simulink model "Control_model_10DOF_fin"  (R2016b)
settings: Solver=FixedStepAuto  StartTime=0.0  StopTime=10  FixedStep=0.0001  RelTol=1e-3
InitFcn:
  | Initialisation_ctr_10DOF_fin
values from neighbouring files (symbols this model uses):
  COM_Parameters = [-lpelvis/2;r2;0]    [Initialisation_ctr_10DOF_fin.m]
  DH_Parameters = [hfoot 0 ... (first row only)    [Initialisation_ctr_10DOF_fin.m]
  dTrunk = trunklbd(3)    [Initialisation_ctr_10DOF_fin.m]
  dxFootSM = dxFoot    [Initialisation_ctr_10DOF_fin.m]
  dxTrunk = 0.1    [Initialisation_ctr_10DOF_fin.m]
  Foot_Parameters = [0;-(lFoot/2-lHeel);0]    [Initialisation_ctr_10DOF_fin.m]
  HAA2HEE = [0; 0; 0.001]    [Initialisation_ctr_10DOF_fin.m]
  HEE2HFE = 0.5*[0.2; 0; 0]    [Initialisation_ctr_10DOF_fin.m]
  height_vrp = CoM_position(1)    [Initialisation_ctr_10DOF_fin.m]
  hTrunk = trunklbd(1)    [Initialisation_ctr_10DOF_fin.m]
  initial_CoM_position = R*CoM_position    [Initialisation_ctr_10DOF_fin.m]
  initial_CoM_velocity = [0;0;0]    [Initialisation_ctr_10DOF_fin.m]
  initial_left_foot = [0;0;-stance_width/2]    [Initialisation_ctr_10DOF_fin.m]
  initial_right_foot = [0;0;stance_width/2]    [Initialisation_ctr_10DOF_fin.m]
  initial_RorL = 0    [Initialisation_ctr_10DOF_fin.m]
  jointsinitial = [9;-15;6;0;0;6;-15;9]/180*pi    [Initialisation_ctr_10DOF_fin.m]
  K_DCM = 4.3*[1 0 0 ... (first row only)    [Initialisation_ctr_10DOF_fin.m]
  kD_left = mbody*[0.95 0 0 0 ... (first row only)    [Initialisation_ctr_10DOF_fin.m]
  kD_right = mbody*[0.12 0 0 0 ... (first row only)    [Initialisation_ctr_10DOF_fin.m]
  kI_left = mbody*[35 0 0 0 ... (first row only)    [Initialisation_ctr_10DOF_fin.m]
  kI_right = mbody*[38.2 0 0 0 ... (first row only)    [Initialisation_ctr_10DOF_fin.m]
  kP_left = mbody*[75 0 0 0 ... (first row only)    [Initialisation_ctr_10DOF_fin.m]
  kP_right = mbody*[5.6 0 0 0 ... (first row only)    [Initialisation_ctr_10DOF_fin.m]
  Lenght = [lShank;lThigh]    [Initialisation_ctr_10DOF_fin.m]
  lFootSM = lFoot    [Initialisation_ctr_10DOF_fin.m]
  lpelvis = wPelvis    [Initialisation_ctr_10DOF_fin.m]
  mass = mbody    (= 60)    [Initialisation_ctr_10DOF_fin.m]
  Masses = [mThigh; mShank; mTrunk]    [Initialisation_ctr_10DOF_fin.m]
  nb_step = 4    [Initialisation_ctr_10DOF_fin.m]
  nb_step_pattern = 20    [Initialisation_ctr_10DOF_fin.m]
  Pelvis_Parameters = [-lpelvis/2;hTrunk/2;0]    [Initialisation_ctr_10DOF_fin.m]
  stance_width = lpelvis    [Initialisation_ctr_10DOF_fin.m]
  stride_lenght = 0.50    (= 0.5)    [Initialisation_ctr_10DOF_fin.m]
  T_DS = time_DS    (= 0.4)    [Initialisation_ctr_10DOF_fin.m]
  T_IT = time_DS    (= 0.4)    [Initialisation_ctr_10DOF_fin.m]
  T_SS = time_swing    (= 1.6)    [Initialisation_ctr_10DOF_fin.m]
  time_DS = (time_stance-time_swing)/2    (= 0.4)    [Initialisation_ctr_10DOF_fin.m]
  time_stance = 60/100*time_stride    (= 2.4)    [Initialisation_ctr_10DOF_fin.m]
  time_step = time_stride/2    (= 2)    [Initialisation_ctr_10DOF_fin.m]
  time_swing = 40/100*time_stride    (= 1.6)    [Initialisation_ctr_10DOF_fin.m]
  validity_angle = [-20*pi/180 20*pi/180 ... (first row only)    [Initialisation_ctr_10DOF_fin.m]
  wTrunk = trunklbd(2)    [Initialisation_ctr_10DOF_fin.m]
  x4CoM = CoM_position(1)-XR4(1)    [Initialisation_ctr_10DOF_fin.m]
undefined symbols (not defined in the file or in its folder): dsegment, hFoot, l, lFoot, omega0_x, omega0_z, rho, wPelvis, X, Xp_x, Xp_z, Y, Z
undefined symbols (not defined in the file): k_grf, lShankSM, lThighSM, mShank, mThigh
libraries: nesl_utility x247, sm_lib x215, dspindex x12, FootPlacementLibrary x8, dspsigops x4, dspswit3 x1
(part 16 of 18)

== matlab function Control_model_10DOF_fin/Forward Kinematics/Forward Kinematics ==
  data: TR0 output; TR1 output; TR2 output; TR3 output; TR4 output; TR5 output; TR6 output; TR7 output; TR8 output; TR9 output; TRL output; TRthighR output; TRshankR output; TRtrunk output; TRshankL output; TRthighL output; TL9 output; TL8 output; TL7 output; TL6 output; TL5 output; TL4 output; TL3 output; TL2 output; TL1 output; TL0 output; TLR output; TLthighL output; TLshankL output; TLtrunk output; TLshankR output; TLthighR output; TWR output; TWL output; TW0 output; TW1 output; TW2 output; TW3 output; TW4 output; TW5 output; TW6 output; TW7 output; TW8 output; TW9 output; TWthighR output; TWthighL output; TWshankR output; TWshankL output; TWtrunk output; XRcom output; XLcom output; XWcom output; joint_angle input double; DH_Parameters parameter double size=[9 2]; COM_Parameters parameter double size=[3 1]; Foot_Parameters parameter double size=[3 1]; inactuated_joint_angle input; V_CoM input; R_foot_Rotation input; Masses parameter; Lenght parameter; Pelvis_Parameters parameter; R_foot_pos input; VWcom output; AWcom output; L_foot_Rotation input; L_foot_pos input; JRcom output; JLcom output; A_CoM input
function [TR0,TR1,TR2,TR3,TR4,TR5,TR6,TR7,TR8,TR9,TRL,TRthighR,TRshankR,TRtrunk,TRshankL,TRthighL,TL9,TL8,TL7,TL6,TL5,TL4,TL3,TL2,TL1,TL0,TLR,TLthighL,TLshankL,TLtrunk,TLshankR,TLthighR,TWR,TWL,TW0,TW1,TW2,TW3,TW4,TW5,TW6,TW7,TW8,TW9,TWthighR,TWthighL,TWshankR,TWshankL,TWtrunk,XRcom,XLcom,XWcom,VWcom,AWcom,JRcom,JLcom]=Forward_Kinematics(joint_angle,DH_Parameters, COM_Parameters, Foot_Parameters,inactuated_joint_angle,V_CoM,R_foot_Rotation,Masses, Lenght,Pelvis_Parameters,R_foot_pos,L_foot_Rotation,L_foot_pos,A_CoM)

%% angle
theta1=joint_angle(1);
theta2=joint_angle(2);
theta3=joint_angle(3);
theta4=joint_angle(4);
theta5=joint_angle(5);
theta6=joint_angle(6);
theta7=joint_angle(7);
theta8=joint_angle(8);
theta0=inactuated_joint_angle(1);
theta9=inactuated_joint_angle(2);

%% Denavit-Hartenberg parmeters
a0=DH_Parameters(1,1);
d1=DH_Parameters(1,2);
a1=DH_Parameters(2,1);
d2=DH_Parameters(2,2);
a2=DH_Parameters(3,1);
d3=DH_Parameters(3,2);
a3=DH_Parameters(4,1);
d4=DH_Parameters(4,2);
a4=DH_Parameters(5,1);
d5=DH_Parameters(5,2);
a5=DH_Parameters(6,1);
d6=DH_Parameters(6,2);
a6=DH_Parameters(7,1);
d7=DH_Parameters(7,2);
a7=DH_Parameters(8,1);
d8=DH_Parameters(8,2);
a8=DH_Parameters(9,1);
d9=DH_Parameters(9,2);

xcom=COM_Parameters(1);
ycom=COM_Parameters(2);
zcom=COM_Parameters(3);
xfoot=Foot_Parameters(1);
yfoot=Foot_Parameters(2);
zfoot=Foot_Parameters(3);

%% Pelvis Parameters
xpelvis=Pelvis_Parameters(1);
ypelvis=Pelvis_Parameters(2);
zpelvis=Pelvis_Parameters(3);


%% Masses
mthigh=Masses(1);
mshank=Masses(2);
mtrunk=Masses(3);

%% Lenght
lshank=Lenght(1);
lthigh=Lenght(2);


%Matrice de Transformation Homogéne

% World -> Right foot marker R

TWR_D=[R_foot_Rotation(1,1) R_foot_Rotation(1,2) R_foot_Rotation(1,3) R_foot_pos(1);
    R_foot_Rotation(2,1) R_foot_Rotation(2,2) R_foot_Rotation(2,3) R_foot_pos(2);
    R_foot_Rotation(3,1) R_foot_Rotation(3,2) R_foot_Rotation(3,3) R_foot_pos(3);
    0 0 0 1];

T=[0 1 0 0;
    1 0 0 0;
    0 0 -1 0;
    0 0 0 1];

TWR=TWR_D*T;

RWR=TWR(1:3,1:3);
XWR=TWR(1:3,4);

% World -> Left foot marker L

TWL_D=[L_foot_Rotation(1,1) L_foot_Rotation(1,2) L_foot_Rotation(1,3) L_foot_pos(1);
    L_foot_Rotation(2,1) L_foot_Rotation(2,2) L_foot_Rotation(2,3) L_foot_pos(2);
    L_foot_Rotation(3,1) L_foot_Rotation(3,2) L_foot_Rotation(3,3) L_foot_pos(3);
    0 0 0 1];

T=[0 -1 0 0;
    1 0 0 0;
    0 0 1 0;
    0 0 0 1];

TWL=TWL_D*T;

RWL=TWL(1:3,1:3);
XWL=TWL(1:3,4);


%Right foot marker R -> Right foot marker 0

TR0=[1 0 0 xfoot;
    0 1 0 yfoot;
    0 0 1 zfoot;
    0 0 0 1];

T0R=[1 0 0 -xfoot;
    0 1 0 -yfoot;
    0 0 1 -zfoot;
    0 0 0 1];

% Right foot marker 0 -> Right ankle eversion/inversion

T0ankleR=[cos(theta0) 0 sin(theta0) a0;
    0 1 0 0;
    -sin(theta0) 0 cos(theta0) 0;
    0 0 0 1];

R0ankleR=[cos(theta0) 0 sin(theta0);
    0 1 0;
    -sin(theta0) 0 cos(theta0)];

O0OankleR=[a0;0;0];

TankleR0=[R0ankleR.' -R0ankleR.'*O0OankleR;
    0 0 0 1];

% Right ankle eversion/inversion -> Right ankle flexion/extension

TankleR1=[cos(theta1) -sin(theta1) 0 0;
    sin(theta1) cos(theta1) 0 0;
    0 0 1 0;
    0 0 0 1];

RankleR1=[cos(theta1) -sin(theta1) 0;
    sin(theta1) cos(theta1) 0;
    0 0 1];

OankleRO1=[0;0;0];

T1ankleR=[RankleR1.' OankleRO1;
    0 0 0 1];

% Right ankle -> Right knee

T12=[cos(theta2) -sin(theta2) 0 a1;
    sin(theta2) cos(theta2) 0 0;
    0 0 1 0;
    0 0 0 1];

R12=[cos(theta2) -sin(theta2) 0;
    sin(theta2) cos(theta2) 0;
    0 0 1];

O1O2=[a1;0;0];

T21=[R12.' -R12.'*O1O2;
    0 0 0 1];

% Right knee -> Right hip flexion/extension

T23=[cos(theta3) -sin(theta3) 0 a2;
    sin(theta3) cos(theta3) 0 0;
    0 0 1 d3;
    0 0 0 1];

R23=[cos(theta3) -sin(theta3) 0;
    sin(theta3) cos(theta3) 0;
    0 0 1];

O2O3=[a2;0;d3];

T32=[R23.' -R23.'*O2O3;
    0 0 0 1];

% Right hip flexion/extension -> Right hip abduction

T34=[cos(theta4-pi/2) -sin(theta4-pi/2) 0 0;
    0 0 -1 0;
    sin(theta4-pi/2) cos(theta4-pi/2) 0 0;
    0 0 0 1];

R34=[cos(theta4-pi/2) -sin(theta4-pi/2) 0;
    0 0 -1;
    sin(theta4-pi/2) cos(theta4-pi/2) 0];

O3O4=[0;0;0];

T43=[R34.' -R34.'*O3O4;
    0 0 0 1];

%Right hip abduction -> Left hip aduction

T45=[cos(theta5-pi/2) -sin(theta5-pi/2) 0 a4;
    -sin(theta5-pi/2) -cos(theta5-pi/2) 0 0;
    0 0 -1 0;
    0 0 0 1];

R45=[cos(theta5-pi/2) -sin(theta5-pi/2) 0;
    -sin(theta5-pi/2) -cos(theta5-pi/2) 0;
    0 0 -1];

O4O5=[a4;0;0];

T54=[R45 -R45*O4O5;
    0 0 0 1];

% Left hip abduction -> Left hip flexion

T56=[cos(theta6) -sin(theta6) 0 0;
    0 0 1 0;
    -sin(theta6) -cos(theta6) 0 0;
    0 0 0 1];

R56=[cos(theta6) -sin(theta6) 0;
    0 0 1;
    -sin(theta6) -cos(theta6) 0];

O5O6=[0;0;0];

T65=[R56.' -R56.'*O5O6;
    0 0 0 1];

% Left hip flexion -> Left knee

T67=[cos(theta7) -sin(theta7) 0 a6;
    sin(theta7) cos(theta7) 0 0;
    0 0 1 d7;
    0 0 0 1];

R67=[cos(theta7) -sin(theta7) 0;
    sin(theta7) cos(theta7) 0;
    0 0 1];

O6O7=[a6;0;d7];

T76=[R67.' -R67.'*O6O7;
    0 0 0 1];

% Left knee -> Left ankle flexion/extension

T78=[cos(theta8) -sin(theta8) 0 a7;
    sin(theta8) cos(theta8) 0 0;
    0 0 1 0;
    0 0 0 1];

R78=[cos(theta8) -sin(theta8) 0;
    sin(theta8) cos(theta8) 0;
    0 0 1];

O7O8=[a7;0;0];

T87=[R78.' -R78.'*O7O8;
    0 0 0 1];

% Left ankle flexion/extension -> Left ankle eversion/inversion

T8ankleL=[cos(theta9) 0 -sin(theta9) 0;
    0 1 0 0;
    sin(theta9) 0 cos(theta9) 0;
    0 0 0 1];

R8ankleL=[cos(theta9) 0 -sin(theta9);
    0 1 0;
    sin(theta9) 0 cos(theta9)];

O8OankleL=[0;0;0];

TankleL8=[R8ankleL.' -R8ankleL.'*O8OankleL;
    0 0 0 1];


% Left ankle eversion/inversion -> Left foot marker 9

TankleL9=[1 0 0 a8;
    0 1 0 0;
    0 0 1 0;
    0 0 0 1];

T9ankleL=[1 0 0 -a8;
    0 1 0 0;
    0 0 1 0;
    0 0 0 1];

% Left foot marker L

T9L=[1 0 0 -xfoot;
    0 1 0 yfoot;
    0 0 1 zfoot;
    0 0 0 1];

TL9=[1 0 0 xfoot;
    0 1 0 -yfoot;
    0 0 1 -zfoot;
    0 0 0 1];

% Right ankle -> Right shank

T1shank=[1 0 0 lshank/2;
    0 1 0 0;
    0 0 1 0;
    0 0 0 1];

Tshank1=[1 0 0 -lshank/2;
    0 1 0 0;
    0 0 1 0;
    0 0 0 1];

% Left knee -> Left Shank

T7shank=[1 0 0 -lshank/2;
    0 1 0 0;
    0 0 1 0;
    0 0 0 1];

Tshank7=[1 0 0 lshank/2;
    0 1 0 0;
    0 0 1 0;
    0 0 0 1];

% Right knee -> Right thigh

T2thigh=[1 0 0 lthigh/2;
    0 1 0 0;
    0 0 1 0;
    0 0 0 1];

Tthigh2=[1 0 0 -lthigh/2;
    0 1 0 0;
    0 0 1 0;
    0 0 0 1];

% Left hip -> Left thigh

T6thigh=[1 0 0 -lthigh/2;
    0 1 0 0 ;
    0 0 1 d7;
    0 0 0 1];

Tthigh6=[1 0 0 lthigh/2;
    0 1 0 0 ;
    0 0 1 -d7;
    0 0 0 1];

% Right hip -> Trunk

T4trunk=[1 0 0 xpelvis;
    0 1 0 ypelvis;
    0 0 1 zpelvis;
    0 0 0 1];

Ttrunk4=[1 0 0 -xpelvis;
    0 1 0 -ypelvis;
    0 0 1 -zpelvis;
    0 0 0 1];

% Right foot frame marker 0

T01=T0ankleR*TankleR1;
T02=T01*T12;
T03=T02*T23;
T04=T03*T34;
T05=T04*T45;
T06=T05*T56;
T07=T06*T67;
T08=T07*T78;
T0ankleL=T08*T8ankleL;
T09=T0ankleL*TankleL9;
T0L=T09*T9L;

T0thighR=T02*T2thigh;
T0thighL=T06*T6thigh;
T0shankR=T01*T1shank;
T0shankL=T07*T7shank;
T0trunk=T04*T4trunk;

X0thighR=T0thighR(1:3,4);
X0thighL=T0thighL(1:3,4);
X0shankR=T0shankR(1:3,4);
X0shankL=T0shankL(1:3,4);
X0trunk=T0trunk(1:3,4);

X0com=(mthigh*X0thighR+mthigh*X0thighL+mshank*X0shankR+mshank*X0shankL+mtrunk*X0trunk)/(2*mthigh+2*mshank+mtrunk);


% Right foot frame marker R

TR1=TR0*T0ankleR*TankleR1;
TR2=TR1*T12;
TR3=TR2*T23;
TR4=TR3*T34;
TR5=TR4*T45;
TR6=TR5*T56;
TR7=TR6*T67;
TR8=TR7*T78;
TRankleL=TR8*T8ankleL;
TR9=TRankleL*TankleL9;
TRL=TR9*T9L;

TRthighR=TR2*T2thigh;
TRthighL=TR6*T6thigh;
TRshankR=TR1*T1shank;
TRshankL=TR7*T7shank;
TRtrunk=TR4*T4trunk;

XRthighR=TRthighR(1:3,4);
XRthighL=TRthighL(1:3,4);
XRshankR=TRshankR(1:3,4);
XRshankL=TRshankL(1:3,4);
XRtrunk=TRtrunk(1:3,4);

XRcom=(mthigh*XRthighR+mthigh*XRthighL+mshank*XRshankR+mshank*XRshankL+mtrunk*XRtrunk)/(2*mthigh+2*mshank+mtrunk);

% TRcom
% 
% xRcom=XRcom(1);
% yRcom=yRcom(2);

%Left foot frame marker 9

T98=T9ankleL*TankleL8;
T97=T98*T87;
T96=T97*T76;
T95=T96*T65;
T94=T95*T54;
T93=T94*T43;
T92=T93*T32;
T91=T92*T21;
T90=T91*T1ankleR*TankleR0;
T9R=T90*T0R;

T9thighL=T96*T6thigh;
T9thighR=T92*T2thigh;
T9shankL=T97*T7shank;
T9shankR=T91*T1shank;
T9trunk=T94*T4trunk;

X9thighL=T9thighL(1:3,4);
X9thighR=T9thighR(1:3,4);
X9shankL=T9shankL(1:3,4);
X9shankR=T9shankR(1:3,4);
X9trunk=T9trunk(1:3,4);

X9com=(mthigh*X9thighR+mthigh*X9thighL+mshank*X9shankR+mshank*X9shankL+mtrunk*X9trunk)/(2*mthigh+2*mshank+mtrunk);


%Left foot repere marker L

TL8=TL9*T9ankleL*TankleL8;
TL7=TL8*T87;
TL6=TL7*T76;
TL5=TL6*T65;
TL4=TL5*T54;
TL3=TL4*T43;
TL2=TL3*T32;
TL1=TL2*T21;
TL0=TL1*T1ankleR*TankleR0;
TLR=TL0*T0R;

TLthighL=TL6*T6thigh;
TLthighR=TL2*T2thigh;
TLshankL=TL7*T7shank;
TLshankR=TL1*T1shank;
TLtrunk=TL4*T4trunk;

XLthighL=TLthighL(1:3,4);
XLthighR=TLthighR(1:3,4);
XLshankL=TLshankL(1:3,4);
XLshankR=TLshankR(1:3,4);
XLtrunk=TLtrunk(1:3,4);

XLcom=(mthigh*XLthighR+mthigh*XLthighL+mshank*XLshankR+mshank*XLshankL+mtrunk*XLtrunk)/(2*mthigh+2*mshank+mtrunk);


% World frame

TW0=TWR*TR0;
TW1=TWR*TR1;
TW2=TWR*TR2;
TW3=TWR*TR3;
TW4=TWR*TR4;
TW5=TWL*TL5;
TW6=TWL*TL6;
TW7=TWL*TL7;
TW8=TWL*TL8;
TW9=TWL*TL9;


% TW0=TWL*TL0;
% TW1=TWL*TL1;
% TW2=TWL*TL2;
% TW3=TWL*TL3;
% TW4=TWL*TL4;
% TW5=TWL*TL5;
% TW6=TWL*TL6;
% TW7=TWL*TL7;
% TW8=TWL*TL8;
% TW9=TWL*TL9;



TWthighR=TW2*T2thigh;
TWthighL=TW6*T6thigh;
TWshankR=TW1*T1shank;
TWshankL=TW7*T7shank;
TWtrunk=TW4*T4trunk;

XWshankR=TWshankR(1:3,4);
XWshankL=TWshankL(1:3,4);
XWthighR=TWthighR(1:3,4);
XWthighL=TWthighL(1:3,4);
XWtrunk=TWtrunk(1:3,4);

XWcom=(mthigh*XWthighR+mthigh*XWthighL+mshank*XWshankR+mshank*XWshankL+mtrunk*XWtrunk)/(2*mthigh+2*mshank+mtrunk);



%%%%%%%%%%%%%%%%%%%%%%%%%%%%%%%%%%%%%%%%%%%%%%%%%%%%%%%%%%%%%%%%%%%%%%%%%%%%%%%%%%%%%%%%%%%%%%%%%%

JRcom=zeros(3,8);
JLcom=zeros(3,8);

    %CoM jacobian right foot repere

% JRcom(1,1)=zcom*cos(theta1 + theta2 + theta3)*cos(theta0) - a1*cos(theta0)*sin(theta1) - a2*sin(theta1 + theta2)*cos(theta0) - ycom*sin(theta1 + theta2 + theta3)*cos(theta0)*cos(theta4) - xcom*sin(theta1 + theta2 + theta3)*cos(theta0)*sin(theta4);
% JRcom(1,2)=zcom*cos(theta1 + theta2 + theta3)*cos(theta0) - a2*sin(theta1 + theta2)*cos(theta0) - ycom*sin(theta1 + theta2 + theta3)*cos(theta0)*cos(theta4) - xcom*sin(theta1 + theta2 + theta3)*cos(theta0)*sin(theta4);
% JRcom(1,3)=zcom*cos(theta1 + theta2 + theta3)*cos(theta0) - ycom*sin(theta1 + theta2 + theta3)*cos(theta0)*cos(theta4) - xcom*sin(theta1 + theta2 + theta3)*cos(theta0)*sin(theta4);
% JRcom(1,4)=ycom*cos(theta4)*sin(theta0) + xcom*sin(theta0)*sin(theta4) + xcom*cos(theta1 + theta2 + theta3)*cos(theta0)*cos(theta4) - ycom*cos(theta1 + theta2 + theta3)*cos(theta0)*sin(theta4);
% 
% JRcom(2,1)=zcom*sin(theta1 + theta2 + theta3) + a2*cos(theta1 + theta2) + (ycom*cos(theta1 + theta2 + theta3 + theta4))/2 + (xcom*sin(theta1 + theta2 + theta3 + theta4))/2 + a1*cos(theta1) + (ycom*cos(theta1 + theta2 + theta3 - theta4))/2 - (xcom*sin(theta1 + theta2 + theta3 - theta4))/2;
% JRcom(2,2)=zcom*sin(theta1 + theta2 + theta3) + a2*cos(theta1 + theta2) + (ycom*cos(theta1 + theta2 + theta3 + theta4))/2 + (xcom*sin(theta1 + theta2 + theta3 + theta4))/2 + (ycom*cos(theta1 + theta2 + theta3 - theta4))/2 - (xcom*sin(theta1 + theta2 + theta3 - theta4))/2;
% JRcom(2,3)=zcom*sin(theta1 + theta2 + theta3) + (ycom*cos(theta1 + theta2 + theta3 + theta4))/2 + (xcom*sin(theta1 + theta2 + theta3 + theta4))/2 + (ycom*cos(theta1 + theta2 + theta3 - theta4))/2 - (xcom*sin(theta1 + theta2 + theta3 - theta4))/2;
% JRcom(2,4)=(ycom*cos(theta1 + theta2 + theta3 + theta4))/2 + (xcom*sin(theta1 + theta2 + theta3 + theta4))/2 - (ycom*cos(theta1 + theta2 + theta3 - theta4))/2 + (xcom*sin(theta1 + theta2 + theta3 - theta4))/2;
% 
% JRcom(3,1)=a2*sin(theta1 + theta2)*sin(theta0) + a1*sin(theta0)*sin(theta1) - zcom*cos(theta1 + theta2 + theta3)*sin(theta0) + ycom*sin(theta1 + theta2 + theta3)*cos(theta4)*sin(theta0) + xcom*sin(theta1 + theta2 + theta3)*sin(theta0)*sin(theta4);
% JRcom(3,2)=a2*sin(theta1 + theta2)*sin(theta0) - zcom*cos(theta1 + theta2 + theta3)*sin(theta0) + ycom*sin(theta1 + theta2 + theta3)*cos(theta4)*sin(theta0) + xcom*sin(theta1 + theta2 + theta3)*sin(theta0)*sin(theta4);
% JRcom(3,3)=ycom*sin(theta1 + theta2 + theta3)*cos(theta4)*sin(theta0) - zcom*cos(theta1 + theta2 + theta3)*sin(theta0) + xcom*sin(theta1 + theta2 + theta3)*sin(theta0)*sin(theta4);
% JRcom(3,4)=xcom*(cos(theta0)*sin(theta4) - cos(theta1 + theta2 + theta3)*cos(theta4)*sin(theta0)) + ycom*(cos(theta0)*cos(theta4) + cos(theta1 + theta2 + theta3)*sin(theta0)*sin(theta4));

JRcom(1,1)=-(2*a1*mshank*cos(theta0)*sin(theta1) + 4*a1*mthigh*cos(theta0)*sin(theta1) + 2*a1*mtrunk*cos(theta0)*sin(theta1) + lshank*mshank*cos(theta0)*sin(theta1) + 2*a2*mshank*cos(theta0)*cos(theta1)*sin(theta2) + 2*a2*mshank*cos(theta0)*cos(theta2)*sin(theta1) + 2*a2*mthigh*cos(theta0)*cos(theta1)*sin(theta2) + 2*a2*mthigh*cos(theta0)*cos(theta2)*sin(theta1) + 2*a2*mtrunk*cos(theta0)*cos(theta1)*sin(theta2) + 2*a2*mtrunk*cos(theta0)*cos(theta2)*sin(theta1) + lthigh*mthigh*cos(theta0)*cos(theta1)*sin(theta2) + lthigh*mthigh*cos(theta0)*cos(theta2)*sin(theta1) - 2*mtrunk*zpelvis*cos(theta0)*cos(theta1)*cos(theta2)*cos(theta3) + 2*mtrunk*zpelvis*cos(theta0)*cos(theta1)*sin(theta2)*sin(theta3) + 2*mtrunk*zpelvis*cos(theta0)*cos(theta2)*sin(theta1)*sin(theta3) + 2*mtrunk*zpelvis*cos(theta0)*cos(theta3)*sin(theta1)*sin(theta2) - 2*a6*mshank*cos(theta0)*cos(theta1)*cos(theta2)*cos(theta3)*sin(theta6) + lthigh*mthigh*cos(theta0)*cos(theta1)*cos(theta2)*cos(theta3)*sin(theta6) + 2*a4*mshank*cos(theta0)*cos(theta1)*cos(theta2)*sin(theta3)*sin(theta4) + 2*a4*mshank*cos(theta0)*cos(theta1)*cos(theta3)*sin(theta2)*sin(theta4) + 2*a4*mshank*cos(theta0)*cos(theta2)*cos(theta3)*sin(theta1)*sin(theta4) + 2*a4*mthigh*cos(theta0)*cos(theta1)*cos(theta2)*sin(theta3)*sin(theta4) + 2*a4*mthigh*cos(theta0)*cos(theta1)*cos(theta3)*sin(theta2)*sin(theta4) + 2*a4*mthigh*cos(theta0)*cos(theta2)*cos(theta3)*sin(theta1)*sin(theta4) + 2*mtrunk*ypelvis*cos(theta0)*cos(theta1)*cos(theta2)*cos(theta4)*sin(theta3) + 2*mtrunk*ypelvis*cos(theta0)*cos(theta1)*cos(theta3)*cos(theta4)*sin(theta2) + 2*mtrunk*ypelvis*cos(theta0)*cos(theta2)*cos(theta3)*cos(theta4)*sin(theta1) + 2*a6*mshank*cos(theta0)*cos(theta1)*sin(theta2)*sin(theta3)*sin(theta6) + 2*a6*mshank*cos(theta0)*cos(theta2)*sin(theta1)*sin(theta3)*sin(theta6) + 2*a6*mshank*cos(theta0)*cos(theta3)*sin(theta1)*sin(theta2)*sin(theta6) + 2*mtrunk*xpelvis*cos(theta0)*cos(theta1)*cos(theta2)*sin(theta3)*sin(theta4) + 2*mtrunk*xpelvis*cos(theta0)*cos(theta1)*cos(theta3)*sin(theta2)*sin(theta4) + 2*mtrunk*xpelvis*cos(theta0)*cos(theta2)*cos(theta3)*sin(theta1)*sin(theta4) - lthigh*mthigh*cos(theta0)*cos(theta1)*sin(theta2)*sin(theta3)*sin(theta6) - lthigh*mthigh*cos(theta0)*cos(theta2)*sin(theta1)*sin(theta3)*sin(theta6) - lthigh*mthigh*cos(theta0)*cos(theta3)*sin(theta1)*sin(theta2)*sin(theta6) - 2*a4*mshank*cos(theta0)*sin(theta1)*sin(theta2)*sin(theta3)*sin(theta4) - 2*a4*mthigh*cos(theta0)*sin(theta1)*sin(theta2)*sin(theta3)*sin(theta4) - 2*mtrunk*ypelvis*cos(theta0)*cos(theta4)*sin(theta1)*sin(theta2)*sin(theta3) - 2*mtrunk*xpelvis*cos(theta0)*sin(theta1)*sin(theta2)*sin(theta3)*sin(theta4) + lshank*mshank*cos(theta0)*cos(theta1)*cos(theta2)*cos(theta3)*cos(theta6)*sin(theta7) + lshank*mshank*cos(theta0)*cos(theta1)*cos(theta2)*cos(theta3)*cos(theta7)*sin(theta6) - 2*d7*mshank*cos(theta0)*cos(theta1)*cos(theta2)*cos(theta4)*sin(theta3)*sin(theta5) + 2*d7*mshank*cos(theta0)*cos(theta1)*cos(theta2)*cos(theta5)*sin(theta3)*sin(theta4) - 2*d7*mshank*cos(theta0)*cos(theta1)*cos(theta3)*cos(theta4)*sin(theta2)*sin(theta5) + 2*d7*mshank*cos(theta0)*cos(theta1)*cos(theta3)*cos(theta5)*sin(theta2)*sin(theta4) - 2*d7*mshank*cos(theta0)*cos(theta2)*cos(theta3)*cos(theta4)*sin(theta1)*sin(theta5) + 2*d7*mshank*cos(theta0)*cos(theta2)*cos(theta3)*cos(theta5)*sin(theta1)*sin(theta4) - 2*d7*mthigh*cos(theta0)*cos(theta1)*cos(theta2)*cos(theta4)*sin(theta3)*sin(theta5) + 2*d7*mthigh*cos(theta0)*cos(theta1)*cos(theta2)*cos(theta5)*sin(theta3)*sin(theta4) - 2*d7*mthigh*cos(theta0)*cos(theta1)*cos(theta3)*cos(theta4)*sin(theta2)*sin(theta5) + 2*d7*mthigh*cos(theta0)*cos(theta1)*cos(theta3)*cos(theta5)*sin(theta2)*sin(theta4) - 2*d7*mthigh*cos(theta0)*cos(theta2)*cos(theta3)*cos(theta4)*sin(theta1)*sin(theta5) + 2*d7*mthigh*cos(theta0)*cos(theta2)*cos(theta3)*cos(theta5)*sin(theta1)*sin(theta4) - lshank*mshank*cos(theta0)*cos(theta1)*cos(theta6)*sin(theta2)*sin(theta3)*sin(theta7) - lshank*mshank*cos(theta0)*cos(theta1)*cos(theta7)*sin(theta2)*sin(theta3)*sin(theta6) - lshank*mshank*cos(theta0)*cos(theta2)*cos(theta6)*sin(theta1)*sin(theta3)*sin(theta7) - lshank*mshank*cos(theta0)*cos(theta2)*cos(theta7)*sin(theta1)*sin(theta3)*sin(theta6) - lshank*mshank*cos(theta0)*cos(theta3)*cos(theta6)*sin(theta1)*sin(theta2)*sin(theta7) - lshank*mshank*cos(theta0)*cos(theta3)*cos(theta7)*sin(theta1)*sin(theta2)*sin(theta6) + 2*d7*mshank*cos(theta0)*cos(theta4)*sin(theta1)*sin(theta2)*sin(theta3)*sin(theta5) - 2*d7*mshank*cos(theta0)*cos(theta5)*sin(theta1)*sin(theta2)*sin(theta3)*sin(theta4) + 2*d7*mthigh*cos(theta0)*cos(theta4)*sin(theta1)*sin(theta2)*sin(theta3)*sin(theta5) - 2*d7*mthigh*cos(theta0)*cos(theta5)*sin(theta1)*sin(theta2)*sin(theta3)*sin(theta4) + 2*a6*mshank*cos(theta0)*cos(theta1)*cos(theta2)*cos(theta4)*cos(theta5)*cos(theta6)*sin(theta3) + 2*a6*mshank*cos(theta0)*cos(theta1)*cos(theta3)*cos(theta4)*cos(theta5)*cos(theta6)*sin(theta2) + 2*a6*mshank*cos(theta0)*cos(theta2)*cos(theta3)*cos(theta4)*cos(theta5)*cos(theta6)*sin(theta1) - lthigh*mthigh*cos(theta0)*cos(theta1)*cos(theta2)*cos(theta4)*cos(theta5)*cos(theta6)*sin(theta3) - lthigh*mthigh*cos(theta0)*cos(theta1)*cos(theta3)*cos(theta4)*cos(theta5)*cos(theta6)*sin(theta2) - lthigh*mthigh*cos(theta0)*cos(theta2)*cos(theta3)*cos(theta4)*cos(theta5)*cos(theta6)*sin(theta1) + 2*a6*mshank*cos(theta0)*cos(theta1)*cos(theta2)*cos(theta6)*sin(theta3)*sin(theta4)*sin(theta5) + 2*a6*mshank*cos(theta0)*cos(theta1)*cos(theta3)*cos(theta6)*sin(theta2)*sin(theta4)*sin(theta5) + 2*a6*mshank*cos(theta0)*cos(theta2)*cos(theta3)*cos(theta6)*sin(theta1)*sin(theta4)*sin(theta5) - 2*a6*mshank*cos(theta0)*cos(theta4)*cos(theta5)*cos(theta6)*sin(theta1)*sin(theta2)*sin(theta3) - lthigh*mthigh*cos(theta0)*cos(theta1)*cos(theta2)*cos(theta6)*sin(theta3)*sin(theta4)*sin(theta5) - lthigh*mthigh*cos(theta0)*cos(theta1)*cos(theta3)*cos(theta6)*sin(theta2)*sin(theta4)*sin(theta5) - lthigh*mthigh*cos(theta0)*cos(theta2)*cos(theta3)*cos(theta6)*sin(theta1)*sin(theta4)*sin(theta5) + lthigh*mthigh*cos(theta0)*cos(theta4)*cos(theta5)*cos(theta6)*sin(theta1)*sin(theta2)*sin(theta3) - 2*a6*mshank*cos(theta0)*cos(theta6)*sin(theta1)*sin(theta2)*sin(theta3)*sin(theta4)*sin(theta5) + lthigh*mthigh*cos(theta0)*cos(theta6)*sin(theta1)*sin(theta2)*sin(theta3)*sin(theta4)*sin(theta5) - lshank*mshank*cos(theta0)*cos(theta1)*cos(theta2)*cos(theta4)*cos(theta5)*cos(theta6)*cos(theta7)*sin(theta3) - lshank*mshank*cos(theta0)*cos(theta1)*cos(theta3)*cos(theta4)*cos(theta5)*cos(theta6)*cos(theta7)*sin(theta2) - lshank*mshank*cos(theta0)*cos(theta2)*cos(theta3)*cos(theta4)*cos(theta5)*cos(theta6)*cos(theta7)*sin(theta1) + lshank*mshank*cos(theta0)*cos(theta1)*cos(theta2)*cos(theta4)*cos(theta5)*sin(theta3)*sin(theta6)*sin(theta7) - lshank*mshank*cos(theta0)*cos(theta1)*cos(theta2)*cos(theta6)*cos(theta7)*sin(theta3)*sin(theta4)*sin(theta5) + lshank*mshank*cos(theta0)*cos(theta1)*cos(theta3)*cos(theta4)*cos(theta5)*sin(theta2)*sin(theta6)*sin(theta7) - lshank*mshank*cos(theta0)*cos(theta1)*cos(theta3)*cos(theta6)*cos(theta7)*sin(theta2)*sin(theta4)*sin(theta5) + lshank*mshank*cos(theta0)*cos(theta2)*cos(theta3)*cos(theta4)*cos(theta5)*sin(theta1)*sin(theta6)*sin(theta7) - lshank*mshank*cos(theta0)*cos(theta2)*cos(theta3)*cos(theta6)*cos(theta7)*sin(theta1)*sin(theta4)*sin(theta5) + lshank*mshank*cos(theta0)*cos(theta4)*cos(theta5)*cos(theta6)*cos(theta7)*sin(theta1)*sin(theta2)*sin(theta3) + lshank*mshank*cos(theta0)*cos(theta1)*cos(theta2)*sin(theta3)*sin(theta4)*sin(theta5)*sin(theta6)*sin(theta7) + lshank*mshank*cos(theta0)*cos(theta1)*cos(theta3)*sin(theta2)*sin(theta4)*sin(theta5)*sin(theta6)*sin(theta7) + lshank*mshank*cos(theta0)*cos(theta2)*cos(theta3)*sin(theta1)*sin(theta4)*sin(theta5)*sin(theta6)*sin(theta7) - lshank*mshank*cos(theta0)*cos(theta4)*cos(theta5)*sin(theta1)*sin(theta2)*sin(theta3)*sin(theta6)*sin(theta7) + lshank*mshank*cos(theta0)*cos(theta6)*cos(theta7)*sin(theta1)*sin(theta2)*sin(theta3)*sin(theta4)*sin(theta5) - lshank*mshank*cos(theta0)*sin(theta1)*sin(theta2)*sin(theta3)*sin(theta4)*sin(theta5)*sin(theta6)*sin(theta7))/(4*mshank + 4*mthigh + 2*mtrunk);
JRcom(1,2)=-(2*a2*mshank*cos(theta0)*cos(theta1)*sin(theta2) + 2*a2*mshank*cos(theta0)*cos(theta2)*sin(theta1) + 2*a2*mthigh*cos(theta0)*cos(theta1)*sin(theta2) + 2*a2*mthigh*cos(theta0)*cos(theta2)*sin(theta1) + 2*a2*mtrunk*cos(theta0)*cos(theta1)*sin(theta2) + 2*a2*mtrunk*cos(theta0)*cos(theta2)*sin(theta1) + lthigh*mthigh*cos(theta0)*cos(theta1)*sin(theta2) + lthigh*mthigh*cos(theta0)*cos(theta2)*sin(theta1) - 2*mtrunk*zpelvis*cos(theta0)*cos(theta1)*cos(theta2)*cos(theta3) + 2*mtrunk*zpelvis*cos(theta0)*cos(theta1)*sin(theta2)*sin(theta3) + 2*mtrunk*zpelvis*cos(theta0)*cos(theta2)*sin(theta1)*sin(theta3) + 2*mtrunk*zpelvis*cos(theta0)*cos(theta3)*sin(theta1)*sin(theta2) - 2*a6*mshank*cos(theta0)*cos(theta1)*cos(theta2)*cos(theta3)*sin(theta6) + lthigh*mthigh*cos(theta0)*cos(theta1)*cos(theta2)*cos(theta3)*sin(theta6) + 2*a4*mshank*cos(theta0)*cos(theta1)*cos(theta2)*sin(theta3)*sin(theta4) + 2*a4*mshank*cos(theta0)*cos(theta1)*cos(theta3)*sin(theta2)*sin(theta4) + 2*a4*mshank*cos(theta0)*cos(theta2)*cos(theta3)*sin(theta1)*sin(theta4) + 2*a4*mthigh*cos(theta0)*cos(theta1)*cos(theta2)*sin(theta3)*sin(theta4) + 2*a4*mthigh*cos(theta0)*cos(theta1)*cos(theta3)*sin(theta2)*sin(theta4) + 2*a4*mthigh*cos(theta0)*cos(theta2)*cos(theta3)*sin(theta1)*sin(theta4) + 2*mtrunk*ypelvis*cos(theta0)*cos(theta1)*cos(theta2)*cos(theta4)*sin(theta3) + 2*mtrunk*ypelvis*cos(theta0)*cos(theta1)*cos(theta3)*cos(theta4)*sin(theta2) + 2*mtrunk*ypelvis*cos(theta0)*cos(theta2)*cos(theta3)*cos(theta4)*sin(theta1) + 2*a6*mshank*cos(theta0)*cos(theta1)*sin(theta2)*sin(theta3)*sin(theta6) + 2*a6*mshank*cos(theta0)*cos(theta2)*sin(theta1)*sin(theta3)*sin(theta6) + 2*a6*mshank*cos(theta0)*cos(theta3)*sin(theta1)*sin(theta2)*sin(theta6) + 2*mtrunk*xpelvis*cos(theta0)*cos(theta1)*cos(theta2)*sin(theta3)*sin(theta4) + 2*mtrunk*xpelvis*cos(theta0)*cos(theta1)*cos(theta3)*sin(theta2)*sin(theta4) + 2*mtrunk*xpelvis*cos(theta0)*cos(theta2)*cos(theta3)*sin(theta1)*sin(theta4) - lthigh*mthigh*cos(theta0)*cos(theta1)*sin(theta2)*sin(theta3)*sin(theta6) - lthigh*mthigh*cos(theta0)*cos(theta2)*sin(theta1)*sin(theta3)*sin(theta6) - lthigh*mthigh*cos(theta0)*cos(theta3)*sin(theta1)*sin(theta2)*sin(theta6) - 2*a4*mshank*cos(theta0)*sin(theta1)*sin(theta2)*sin(theta3)*sin(theta4) - 2*a4*mthigh*cos(theta0)*sin(theta1)*sin(theta2)*sin(theta3)*sin(theta4) - 2*mtrunk*ypelvis*cos(theta0)*cos(theta4)*sin(theta1)*sin(theta2)*sin(theta3) - 2*mtrunk*xpelvis*cos(theta0)*sin(theta1)*sin(theta2)*sin(theta3)*sin(theta4) + lshank*mshank*cos(theta0)*cos(theta1)*cos(theta2)*cos(theta3)*cos(theta6)*sin(theta7) + lshank*mshank*cos(theta0)*cos(theta1)*cos(theta2)*cos(theta3)*cos(theta7)*sin(theta6) - 2*d7*mshank*cos(theta0)*cos(theta1)*cos(theta2)*cos(theta4)*sin(theta3)*sin(theta5) + 2*d7*mshank*cos(theta0)*cos(theta1)*cos(theta2)*cos(theta5)*sin(theta3)*sin(theta4) - 2*d7*mshank*cos(theta0)*cos(theta1)*cos(theta3)*cos(theta4)*sin(theta2)*sin(theta5) + 2*d7*mshank*cos(theta0)*cos(theta1)*cos(theta3)*cos(theta5)*sin(theta2)*sin(theta4) - 2*d7*mshank*cos(theta0)*cos(theta2)*cos(theta3)*cos(theta4)*sin(theta1)*sin(theta5) + 2*d7*mshank*cos(theta0)*cos(theta2)*cos(theta3)*cos(theta5)*sin(theta1)*sin(theta4) - 2*d7*mthigh*cos(theta0)*cos(theta1)*cos(theta2)*cos(theta4)*sin(theta3)*sin(theta5) + 2*d7*mthigh*cos(theta0)*cos(theta1)*cos(theta2)*cos(theta5)*sin(theta3)*sin(theta4) - 2*d7*mthigh*cos(theta0)*cos(theta1)*cos(theta3)*cos(theta4)*sin(theta2)*sin(theta5) + 2*d7*mthigh*cos(theta0)*cos(theta1)*cos(theta3)*cos(theta5)*sin(theta2)*sin(theta4) - 2*d7*mthigh*cos(theta0)*cos(theta2)*cos(theta3)*cos(theta4)*sin(theta1)*sin(theta5) + 2*d7*mthigh*cos(theta0)*cos(theta2)*cos(theta3)*cos(theta5)*sin(theta1)*sin(theta4) - lshank*mshank*cos(theta0)*cos(theta1)*cos(theta6)*sin(theta2)*sin(theta3)*sin(theta7) - lshank*mshank*cos(theta0)*cos(theta1)*cos(theta7)*sin(theta2)*sin(theta3)*sin(theta6) - lshank*mshank*cos(theta0)*cos(theta2)*cos(theta6)*sin(theta1)*sin(theta3)*sin(theta7) - lshank*mshank*cos(theta0)*cos(theta2)*cos(theta7)*sin(theta1)*sin(theta3)*sin(theta6) - lshank*mshank*cos(theta0)*cos(theta3)*cos(theta6)*sin(theta1)*sin(theta2)*sin(theta7) - lshank*mshank*cos(theta0)*cos(theta3)*cos(theta7)*sin(theta1)*sin(theta2)*sin(theta6) + 2*d7*mshank*cos(theta0)*cos(theta4)*sin(theta1)*sin(theta2)*sin(theta3)*sin(theta5) - 2*d7*mshank*cos(theta0)*cos(theta5)*sin(theta1)*sin(theta2)*sin(theta3)*sin(theta4) + 2*d7*mthigh*cos(theta0)*cos(theta4)*sin(theta1)*sin(theta2)*sin(theta3)*sin(theta5) - 2*d7*mthigh*cos(theta0)*cos(theta5)*sin(theta1)*sin(theta2)*sin(theta3)*sin(theta4) + 2*a6*mshank*cos(theta0)*cos(theta1)*cos(theta2)*cos(theta4)*cos(theta5)*cos(theta6)*sin(theta3) + 2*a6*mshank*cos(theta0)*cos(theta1)*cos(theta3)*cos(theta4)*cos(theta5)*cos(theta6)*sin(theta2) + 2*a6*mshank*cos(theta0)*cos(theta2)*cos(theta3)*cos(theta4)*cos(theta5)*cos(theta6)*sin(theta1) - lthigh*mthigh*cos(theta0)*cos(theta1)*cos(theta2)*cos(theta4)*cos(theta5)*cos(theta6)*sin(theta3) - lthigh*mthigh*cos(theta0)*cos(theta1)*cos(theta3)*cos(theta4)*cos(theta5)*cos(theta6)*sin(theta2) - lthigh*mthigh*cos(theta0)*cos(theta2)*cos(theta3)*cos(theta4)*cos(theta5)*cos(theta6)*sin(theta1) + 2*a6*mshank*cos(theta0)*cos(theta1)*cos(theta2)*cos(theta6)*sin(theta3)*sin(theta4)*sin(theta5) + 2*a6*mshank*cos(theta0)*cos(theta1)*cos(theta3)*cos(theta6)*sin(theta2)*sin(theta4)*sin(theta5) + 2*a6*mshank*cos(theta0)*cos(theta2)*cos(theta3)*cos(theta6)*sin(theta1)*sin(theta4)*sin(theta5) - 2*a6*mshank*cos(theta0)*cos(theta4)*cos(theta5)*cos(theta6)*sin(theta1)*sin(theta2)*sin(theta3) - lthigh*mthigh*cos(theta0)*cos(theta1)*cos(theta2)*cos(theta6)*sin(theta3)*sin(theta4)*sin(theta5) - lthigh*mthigh*cos(theta0)*cos(theta1)*cos(theta3)*cos(theta6)*sin(theta2)*sin(theta4)*sin(theta5) - lthigh*mthigh*cos(theta0)*cos(theta2)*cos(theta3)*cos(theta6)*sin(theta1)*sin(theta4)*sin(theta5) + lthigh*mthigh*cos(theta0)*cos(theta4)*cos(theta5)*cos(theta6)*sin(theta1)*sin(theta2)*sin(theta3) - 2*a6*mshank*cos(theta0)*cos(theta6)*sin(theta1)*sin(theta2)*sin(theta3)*sin(theta4)*sin(theta5) + lthigh*mthigh*cos(theta0)*cos(theta6)*sin(theta1)*sin(theta2)*sin(theta3)*sin(theta4)*sin(theta5) - lshank*mshank*cos(theta0)*cos(theta1)*cos(theta2)*cos(theta4)*cos(theta5)*cos(theta6)*cos(theta7)*sin(theta3) - lshank*mshank*cos(theta0)*cos(theta1)*cos(theta3)*cos(theta4)*cos(theta5)*cos(theta6)*cos(theta7)*sin(theta2) - lshank*mshank*cos(theta0)*cos(theta2)*cos(theta3)*cos(theta4)*cos(theta5)*cos(theta6)*cos(theta7)*sin(theta1) + lshank*mshank*cos(theta0)*cos(theta1)*cos(theta2)*cos(theta4)*cos(theta5)*sin(theta3)*sin(theta6)*sin(theta7) - lshank*mshank*cos(theta0)*cos(theta1)*cos(theta2)*cos(theta6)*cos(theta7)*sin(theta3)*sin(theta4)*sin(theta5) + lshank*mshank*cos(theta0)*cos(theta1)*cos(theta3)*cos(theta4)*cos(theta5)*sin(theta2)*sin(theta6)*sin(theta7) - lshank*mshank*cos(theta0)*cos(theta1)*cos(theta3)*cos(theta6)*cos(theta7)*sin(theta2)*sin(theta4)*sin(theta5) + lshank*mshank*cos(theta0)*cos(theta2)*cos(theta3)*cos(theta4)*cos(theta5)*sin(theta1)*sin(theta6)*sin(theta7) - lshank*mshank*cos(theta0)*cos(theta2)*cos(theta3)*cos(theta6)*cos(theta7)*sin(theta1)*sin(theta4)*sin(theta5) + lshank*mshank*cos(theta0)*cos(theta4)*cos(theta5)*cos(theta6)*cos(theta7)*sin(theta1)*sin(theta2)*sin(theta3) + lshank*mshank*cos(theta0)*cos(theta1)*cos(theta2)*sin(theta3)*sin(theta4)*sin(theta5)*sin(theta6)*sin(theta7) + lshank*mshank*cos(theta0)*cos(theta1)*cos(theta3)*sin(theta2)*sin(theta4)*sin(theta5)*sin(theta6)*sin(theta7) + lshank*mshank*cos(theta0)*cos(theta2)*cos(theta3)*sin(theta1)*sin(theta4)*sin(theta5)*sin(theta6)*sin(theta7) - lshank*mshank*cos(theta0)*cos(theta4)*cos(theta5)*sin(theta1)*sin(theta2)*sin(theta3)*sin(theta6)*sin(theta7) + lshank*mshank*cos(theta0)*cos(theta6)*cos(theta7)*sin(theta1)*sin(theta2)*sin(theta3)*sin(theta4)*sin(theta5) - lshank*mshank*cos(theta0)*sin(theta1)*sin(theta2)*sin(theta3)*sin(theta4)*sin(theta5)*sin(theta6)*sin(theta7))/(4*mshank + 4*mthigh + 2*mtrunk);
JRcom(1,3)=-(2*mtrunk*zpelvis*cos(theta0)*cos(theta1)*sin(theta2)*sin(theta3) - 2*mtrunk*zpelvis*cos(theta0)*cos(theta1)*cos(theta2)*cos(theta3) + 2*mtrunk*zpelvis*cos(theta0)*cos(theta2)*sin(theta1)*sin(theta3) + 2*mtrunk*zpelvis*cos(theta0)*cos(theta3)*sin(theta1)*sin(theta2) - 2*a6*mshank*cos(theta0)*cos(theta1)*cos(theta2)*cos(theta3)*sin(theta6) + lthigh*mthigh*cos(theta0)*cos(theta1)*cos(theta2)*cos(theta3)*sin(theta6) + 2*a4*mshank*cos(theta0)*cos(theta1)*cos(theta2)*sin(theta3)*sin(theta4) + 2*a4*mshank*cos(theta0)*cos(theta1)*cos(theta3)*sin(theta2)*sin(theta4) + 2*a4*mshank*cos(theta0)*cos(theta2)*cos(theta3)*sin(theta1)*sin(theta4) + 2*a4*mthigh*cos(theta0)*cos(theta1)*cos(theta2)*sin(theta3)*sin(theta4) + 2*a4*mthigh*cos(theta0)*cos(theta1)*cos(theta3)*sin(theta2)*sin(theta4) + 2*a4*mthigh*cos(theta0)*cos(theta2)*cos(theta3)*sin(theta1)*sin(theta4) + 2*mtrunk*ypelvis*cos(theta0)*cos(theta1)*cos(theta2)*cos(theta4)*sin(theta3) + 2*mtrunk*ypelvis*cos(theta0)*cos(theta1)*cos(theta3)*cos(theta4)*sin(theta2) + 2*mtrunk*ypelvis*cos(theta0)*cos(theta2)*cos(theta3)*cos(theta4)*sin(theta1) + 2*a6*mshank*cos(theta0)*cos(theta1)*sin(theta2)*sin(theta3)*sin(theta6) + 2*a6*mshank*cos(theta0)*cos(theta2)*sin(theta1)*sin(theta3)*sin(theta6) + 2*a6*mshank*cos(theta0)*cos(theta3)*sin(theta1)*sin(theta2)*sin(theta6) + 2*mtrunk*xpelvis*cos(theta0)*cos(theta1)*cos(theta2)*sin(theta3)*sin(theta4) + 2*mtrunk*xpelvis*cos(theta0)*cos(theta1)*cos(theta3)*sin(theta2)*sin(theta4) + 2*mtrunk*xpelvis*cos(theta0)*cos(theta2)*cos(theta3)*sin(theta1)*sin(theta4) - lthigh*mthigh*cos(theta0)*cos(theta1)*sin(theta2)*sin(theta3)*sin(theta6) - lthigh*mthigh*cos(theta0)*cos(theta2)*sin(theta1)*sin(theta3)*sin(theta6) - lthigh*mthigh*cos(theta0)*cos(theta3)*sin(theta1)*sin(theta2)*sin(theta6) - 2*a4*mshank*cos(theta0)*sin(theta1)*sin(theta2)*sin(theta3)*sin(theta4) - 2*a4*mthigh*cos(theta0)*sin(theta1)*sin(theta2)*sin(theta3)*sin(theta4) - 2*mtrunk*ypelvis*cos(theta0)*cos(theta4)*sin(theta1)*sin(theta2)*sin(theta3) - 2*mtrunk*xpelvis*cos(theta0)*sin(theta1)*sin(theta2)*sin(theta3)*sin(theta4) + lshank*mshank*cos(theta0)*cos(theta1)*cos(theta2)*cos(theta3)*cos(theta6)*sin(theta7) + lshank*mshank*cos(theta0)*cos(theta1)*cos(theta2)*cos(theta3)*cos(theta7)*sin(theta6) - 2*d7*mshank*cos(theta0)*cos(theta1)*cos(theta2)*cos(theta4)*sin(theta3)*sin(theta5) + 2*d7*mshank*cos(theta0)*cos(theta1)*cos(theta2)*cos(theta5)*sin(theta3)*sin(theta4) - 2*d7*mshank*cos(theta0)*cos(theta1)*cos(theta3)*cos(theta4)*sin(theta2)*sin(theta5) + 2*d7*mshank*cos(theta0)*cos(theta1)*cos(theta3)*cos(theta5)*sin(theta2)*sin(theta4) - 2*d7*mshank*cos(theta0)*cos(theta2)*cos(theta3)*cos(theta4)*sin(theta1)*sin(theta5) + 2*d7*mshank*cos(theta0)*cos(theta2)*cos(theta3)*cos(theta5)*sin(theta1)*sin(theta4) - 2*d7*mthigh*cos(theta0)*cos(theta1)*cos(theta2)*cos(theta4)*sin(theta3)*sin(theta5) + 2*d7*mthigh*cos(theta0)*cos(theta1)*cos(theta2)*cos(theta5)*sin(theta3)*sin(theta4) - 2*d7*mthigh*cos(theta0)*cos(theta1)*cos(theta3)*cos(theta4)*sin(theta2)*sin(theta5) + 2*d7*mthigh*cos(theta0)*cos(theta1)*cos(theta3)*cos(theta5)*sin(theta2)*sin(theta4) - 2*d7*mthigh*cos(theta0)*cos(theta2)*cos(theta3)*cos(theta4)*sin(theta1)*sin(theta5) + 2*d7*mthigh*cos(theta0)*cos(theta2)*cos(theta3)*cos(theta5)*sin(theta1)*sin(theta4) - lshank*mshank*cos(theta0)*cos(theta1)*cos(theta6)*sin(theta2)*sin(theta3)*sin(theta7) - lshank*mshank*cos(theta0)*cos(theta1)*cos(theta7)*sin(theta2)*sin(theta3)*sin(theta6) - lshank*mshank*cos(theta0)*cos(theta2)*cos(theta6)*sin(theta1)*sin(theta3)*sin(theta7) - lshank*mshank*cos(theta0)*cos(theta2)*cos(theta7)*sin(theta1)*sin(theta3)*sin(theta6) - lshank*mshank*cos(theta0)*cos(theta3)*cos(theta6)*sin(theta1)*sin(theta2)*sin(theta7) - lshank*mshank*cos(theta0)*cos(theta3)*cos(theta7)*sin(theta1)*sin(theta2)*sin(theta6) + 2*d7*mshank*cos(theta0)*cos(theta4)*sin(theta1)*sin(theta2)*sin(theta3)*sin(theta5) - 2*d7*mshank*cos(theta0)*cos(theta5)*sin(theta1)*sin(theta2)*sin(theta3)*sin(theta4) + 2*d7*mthigh*cos(theta0)*cos(theta4)*sin(theta1)*sin(theta2)*sin(theta3)*sin(theta5) - 2*d7*mthigh*cos(theta0)*cos(theta5)*sin(theta1)*sin(theta2)*sin(theta3)*sin(theta4) + 2*a6*mshank*cos(theta0)*cos(theta1)*cos(theta2)*cos(theta4)*cos(theta5)*cos(theta6)*sin(theta3) + 2*a6*mshank*cos(theta0)*cos(theta1)*cos(theta3)*cos(theta4)*cos(theta5)*cos(theta6)*sin(theta2) + 2*a6*mshank*cos(theta0)*cos(theta2)*cos(theta3)*cos(theta4)*cos(theta5)*cos(theta6)*sin(theta1) - lthigh*mthigh*cos(theta0)*cos(theta1)*cos(theta2)*cos(theta4)*cos(theta5)*cos(theta6)*sin(theta3) - lthigh*mthigh*cos(theta0)*cos(theta1)*cos(theta3)*cos(theta4)*cos(theta5)*cos(theta6)*sin(theta2) - lthigh*mthigh*cos(theta0)*cos(theta2)*cos(theta3)*cos(theta4)*cos(theta5)*cos(theta6)*sin(theta1) + 2*a6*mshank*cos(theta0)*cos(theta1)*cos(theta2)*cos(theta6)*sin(theta3)*sin(theta4)*sin(theta5) + 2*a6*mshank*cos(theta0)*cos(theta1)*cos(theta3)*cos(theta6)*sin(theta2)*sin(theta4)*sin(theta5) + 2*a6*mshank*cos(theta0)*cos(theta2)*cos(theta3)*cos(theta6)*sin(theta1)*sin(theta4)*sin(theta5) - 2*a6*mshank*cos(theta0)*cos(theta4)*cos(theta5)*cos(theta6)*sin(theta1)*sin(theta2)*sin(theta3) - lthigh*mthigh*cos(theta0)*cos(theta1)*cos(theta2)*cos(theta6)*sin(theta3)*sin(theta4)*sin(theta5) - lthigh*mthigh*cos(theta0)*cos(theta1)*cos(theta3)*cos(theta6)*sin(theta2)*sin(theta4)*sin(theta5) - lthigh*mthigh*cos(theta0)*cos(theta2)*cos(theta3)*cos(theta6)*sin(theta1)*sin(theta4)*sin(theta5) + lthigh*mthigh*cos(theta0)*cos(theta4)*cos(theta5)*cos(theta6)*sin(theta1)*sin(theta2)*sin(theta3) - 2*a6*mshank*cos(theta0)*cos(theta6)*sin(theta1)*sin(theta2)*sin(theta3)*sin(theta4)*sin(theta5) + lthigh*mthigh*cos(theta0)*cos(theta6)*sin(theta1)*sin(theta2)*sin(theta3)*sin(theta4)*sin(theta5) - lshank*mshank*cos(theta0)*cos(theta1)*cos(theta2)*cos(theta4)*cos(theta5)*cos(theta6)*cos(theta7)*sin(theta3) - lshank*mshank*cos(theta0)*cos(theta1)*cos(theta3)*cos(theta4)*cos(theta5)*cos(theta6)*cos(theta7)*sin(theta2) - lshank*mshank*cos(theta0)*cos(theta2)*cos(theta3)*cos(theta4)*cos(theta5)*cos(theta6)*cos(theta7)*sin(theta1) + lshank*mshank*cos(theta0)*cos(theta1)*cos(theta2)*cos(theta4)*cos(theta5)*sin(theta3)*sin(theta6)*sin(theta7) - lshank*mshank*cos(theta0)*cos(theta1)*cos(theta2)*cos(theta6)*cos(theta7)*sin(theta3)*sin(theta4)*sin(theta5) + lshank*mshank*cos(theta0)*cos(theta1)*cos(theta3)*cos(theta4)*cos(theta5)*sin(theta2)*sin(theta6)*sin(theta7) - lshank*mshank*cos(theta0)*cos(theta1)*cos(theta3)*cos(theta6)*cos(theta7)*sin(theta2)*sin(theta4)*sin(theta5) + lshank*mshank*cos(theta0)*cos(theta2)*cos(theta3)*cos(theta4)*cos(theta5)*sin(theta1)*sin(theta6)*sin(theta7) - lshank*mshank*cos(theta0)*cos(theta2)*cos(theta3)*cos(theta6)*cos(theta7)*sin(theta1)*sin(theta4)*sin(theta5) + lshank*mshank*cos(theta0)*cos(theta4)*cos(theta5)*cos(theta6)*cos(theta7)*sin(theta1)*sin(theta2)*sin(theta3) + lshank*mshank*cos(theta0)*cos(theta1)*cos(theta2)*sin(theta3)*sin(theta4)*sin(theta5)*sin(theta6)*sin(theta7) + lshank*mshank*cos(theta0)*cos(theta1)*cos(theta3)*sin(theta2)*sin(theta4)*sin(theta5)*sin(theta6)*sin(theta7) + lshank*mshank*cos(theta0)*cos(theta2)*cos(theta3)*sin(theta1)*sin(theta4)*sin(theta5)*sin(theta6)*sin(theta7) - lshank*mshank*cos(theta0)*cos(theta4)*cos(theta5)*sin(theta1)*sin(theta2)*sin(theta3)*sin(theta6)*sin(theta7) + lshank*mshank*cos(theta0)*cos(theta6)*cos(theta7)*sin(theta1)*sin(theta2)*sin(theta3)*sin(theta4)*sin(theta5) - lshank*mshank*cos(theta0)*sin(theta1)*sin(theta2)*sin(theta3)*sin(theta4)*sin(theta5)*sin(theta6)*sin(theta7))/(4*mshank + 4*mthigh + 2*mtrunk);
JRcom(1,4)=-(2*d7*mshank*cos(theta4)*sin(theta0)*sin(theta5) - 2*mtrunk*xpelvis*sin(theta0)*sin(theta4) - 2*a4*mshank*sin(theta0)*sin(theta4) - 2*a4*mthigh*sin(theta0)*sin(theta4) - 2*mtrunk*ypelvis*cos(theta4)*sin(theta0) - 2*d7*mshank*cos(theta5)*sin(theta0)*sin(theta4) + 2*d7*mthigh*cos(theta4)*sin(theta0)*sin(theta5) - 2*d7*mthigh*cos(theta5)*sin(theta0)*sin(theta4) - 2*a6*mshank*cos(theta4)*cos(theta5)*cos(theta6)*sin(theta0) + lthigh*mthigh*cos(theta4)*cos(theta5)*cos(theta6)*sin(theta0) - 2*a6*mshank*cos(theta6)*sin(theta0)*sin(theta4)*sin(theta5) + lthigh*mthigh*cos(theta6)*sin(theta0)*sin(theta4)*sin(theta5) - 2*a4*mshank*cos(theta0)*cos(theta1)*cos(theta2)*cos(theta3)*cos(theta4) - 2*a4*mthigh*cos(theta0)*cos(theta1)*cos(theta2)*cos(theta3)*cos(theta4) - 2*mtrunk*xpelvis*cos(theta0)*cos(theta1)*cos(theta2)*cos(theta3)*cos(theta4) + lshank*mshank*cos(theta4)*cos(theta5)*cos(theta6)*cos(theta7)*sin(theta0) + 2*a4*mshank*cos(theta0)*cos(theta1)*cos(theta4)*sin(theta2)*sin(theta3) + 2*a4*mshank*cos(theta0)*cos(theta2)*cos(theta4)*sin(theta1)*sin(theta3) + 2*a4*mshank*cos(theta0)*cos(theta3)*cos(theta4)*sin(theta1)*sin(theta2) + 2*a4*mthigh*cos(theta0)*cos(theta1)*cos(theta4)*sin(theta2)*sin(theta3) + 2*a4*mthigh*cos(theta0)*cos(theta2)*cos(theta4)*sin(theta1)*sin(theta3) + 2*a4*mthigh*cos(theta0)*cos(theta3)*cos(theta4)*sin(theta1)*sin(theta2) + 2*mtrunk*ypelvis*cos(theta0)*cos(theta1)*cos(theta2)*cos(theta3)*sin(theta4) + 2*mtrunk*xpelvis*cos(theta0)*cos(theta1)*cos(theta4)*sin(theta2)*sin(theta3) + 2*mtrunk*xpelvis*cos(theta0)*cos(theta2)*cos(theta4)*sin(theta1)*sin(theta3) + 2*mtrunk*xpelvis*cos(theta0)*cos(theta3)*cos(theta4)*sin(theta1)*sin(theta2) - lshank*mshank*cos(theta4)*cos(theta5)*sin(theta0)*sin(theta6)*sin(theta7) + lshank*mshank*cos(theta6)*cos(theta7)*sin(theta0)*sin(theta4)*sin(theta5) - 2*mtrunk*ypelvis*cos(theta0)*cos(theta1)*sin(theta2)*sin(theta3)*sin(theta4) - 2*mtrunk*ypelvis*cos(theta0)*cos(theta2)*sin(theta1)*sin(theta3)*sin(theta4) - 2*mtrunk*ypelvis*cos(theta0)*cos(theta3)*sin(theta1)*sin(theta2)*sin(theta4) - lshank*mshank*sin(theta0)*sin(theta4)*sin(theta5)*sin(theta6)*sin(theta7) - 2*d7*mshank*cos(theta0)*cos(theta1)*cos(theta2)*cos(theta3)*cos(theta4)*cos(theta5) - 2*d7*mthigh*cos(theta0)*cos(theta1)*cos(theta2)*cos(theta3)*cos(theta4)*cos(theta5) - 2*d7*mshank*cos(theta0)*cos(theta1)*cos(theta2)*cos(theta3)*sin(theta4)*sin(theta5) + 2*d7*mshank*cos(theta0)*cos(theta1)*cos(theta4)*cos(theta5)*sin(theta2)*sin(theta3) + 2*d7*mshank*cos(theta0)*cos(theta2)*cos(theta4)*cos(theta5)*sin(theta1)*sin(theta3) + 2*d7*mshank*cos(theta0)*cos(theta3)*cos(theta4)*cos(theta5)*sin(theta1)*sin(theta2) - 2*d7*mthigh*cos(theta0)*cos(theta1)*cos(theta2)*cos(theta3)*sin(theta4)*sin(theta5) + 2*d7*mthigh*cos(theta0)*cos(theta1)*cos(theta4)*cos(theta5)*sin(theta2)*sin(theta3) + 2*d7*mthigh*cos(theta0)*cos(theta2)*cos(theta4)*cos(theta5)*sin(theta1)*sin(theta3) + 2*d7*mthigh*cos(theta0)*cos(theta3)*cos(theta4)*cos(theta5)*sin(theta1)*sin(theta2) + 2*d7*mshank*cos(theta0)*cos(theta1)*sin(theta2)*sin(theta3)*sin(theta4)*sin(theta5) + 2*d7*mshank*cos(theta0)*cos(theta2)*sin(theta1)*sin(theta3)*sin(theta4)*sin(theta5) + 2*d7*mshank*cos(theta0)*cos(theta3)*sin(theta1)*sin(theta2)*sin(theta4)*sin(theta5) + 2*d7*mthigh*cos(theta0)*cos(theta1)*sin(theta2)*sin(theta3)*sin(theta4)*sin(theta5) + 2*d7*mthigh*cos(theta0)*cos(theta2)*sin(theta1)*sin(theta3)*sin(theta4)*sin(theta5) + 2*d7*mthigh*cos(theta0)*cos(theta3)*sin(theta1)*sin(theta2)*sin(theta4)*sin(theta5) - 2*a6*mshank*cos(theta0)*cos(theta1)*cos(theta2)*cos(theta3)*cos(theta4)*cos(theta6)*sin(theta5) + 2*a6*mshank*cos(theta0)*cos(theta1)*cos(theta2)*cos(theta3)*cos(theta5)*cos(theta6)*sin(theta4) + lthigh*mthigh*cos(theta0)*cos(theta1)*cos(theta2)*cos(theta3)*cos(theta4)*cos(theta6)*sin(theta5) - lthigh*mthigh*cos(theta0)*cos(theta1)*cos(theta2)*cos(theta3)*cos(theta5)*cos(theta6)*sin(theta4) + 2*a6*mshank*cos(theta0)*cos(theta1)*cos(theta4)*cos(theta6)*sin(theta2)*sin(theta3)*sin(theta5) - 2*a6*mshank*cos(theta0)*cos(theta1)*cos(theta5)*cos(theta6)*sin(theta2)*sin(theta3)*sin(theta4) + 2*a6*mshank*cos(theta0)*cos(theta2)*cos(theta4)*cos(theta6)*sin(theta1)*sin(theta3)*sin(theta5) - 2*a6*mshank*cos(theta0)*cos(theta2)*cos(theta5)*cos(theta6)*sin(theta1)*sin(theta3)*sin(theta4) + 2*a6*mshank*cos(theta0)*cos(theta3)*cos(theta4)*cos(theta6)*sin(theta1)*sin(theta2)*sin(theta5) - 2*a6*mshank*cos(theta0)*cos(theta3)*cos(theta5)*cos(theta6)*sin(theta1)*sin(theta2)*sin(theta4) - lthigh*mthigh*cos(theta0)*cos(theta1)*cos(theta4)*cos(theta6)*sin(theta2)*sin(theta3)*sin(theta5) + lthigh*mthigh*cos(theta0)*cos(theta1)*cos(theta5)*cos(theta6)*sin(theta2)*sin(theta3)*sin(theta4) - lthigh*mthigh*cos(theta0)*cos(theta2)*cos(theta4)*cos(theta6)*sin(theta1)*sin(theta3)*sin(theta5) + lthigh*mthigh*cos(theta0)*cos(theta2)*cos(theta5)*cos(theta6)*sin(theta1)*sin(theta3)*sin(theta4) - lthigh*mthigh*cos(theta0)*cos(theta3)*cos(theta4)*cos(theta6)*sin(theta1)*sin(theta2)*sin(theta5) + lthigh*mthigh*cos(theta0)*cos(theta3)*cos(theta5)*cos(theta6)*sin(theta1)*sin(theta2)*sin(theta4) + lshank*mshank*cos(theta0)*cos(theta1)*cos(theta2)*cos(theta3)*cos(theta4)*cos(theta6)*cos(theta7)*sin(theta5) - lshank*mshank*cos(theta0)*cos(theta1)*cos(theta2)*cos(theta3)*cos(theta5)*cos(theta6)*cos(theta7)*sin(theta4) - lshank*mshank*cos(theta0)*cos(theta1)*cos(theta2)*cos(theta3)*cos(theta4)*sin(theta5)*sin(theta6)*sin(theta7) + lshank*mshank*cos(theta0)*cos(theta1)*cos(theta2)*cos(theta3)*cos(theta5)*sin(theta4)*sin(theta6)*sin(theta7) - lshank*mshank*cos(theta0)*cos(theta1)*cos(theta4)*cos(theta6)*cos(theta7)*sin(theta2)*sin(theta3)*sin(theta5) + lshank*mshank*cos(theta0)*cos(theta1)*cos(theta5)*cos(theta6)*cos(theta7)*sin(theta2)*sin(theta3)*sin(theta4) - lshank*mshank*cos(theta0)*cos(theta2)*cos(theta4)*cos(theta6)*cos(theta7)*sin(theta1)*sin(theta3)*sin(theta5) + lshank*mshank*cos(theta0)*cos(theta2)*cos(theta5)*cos(theta6)*cos(theta7)*sin(theta1)*sin(theta3)*sin(theta4) - lshank*mshank*cos(theta0)*cos(theta3)*cos(theta4)*cos(theta6)*cos(theta7)*sin(theta1)*sin(theta2)*sin(theta5) + lshank*mshank*cos(theta0)*cos(theta3)*cos(theta5)*cos(theta6)*cos(theta7)*sin(theta1)*sin(theta2)*sin(theta4) + lshank*mshank*cos(theta0)*cos(theta1)*cos(theta4)*sin(theta2)*sin(theta3)*sin(theta5)*sin(theta6)*sin(theta7) - lshank*mshank*cos(theta0)*cos(theta1)*cos(theta5)*sin(theta2)*sin(theta3)*sin(theta4)*sin(theta6)*sin(theta7) + lshank*mshank*cos(theta0)*cos(theta2)*cos(theta4)*sin(theta1)*sin(theta3)*sin(theta5)*sin(theta6)*sin(theta7) - lshank*mshank*cos(theta0)*cos(theta2)*cos(theta5)*sin(theta1)*sin(theta3)*sin(theta4)*sin(theta6)*sin(theta7) + lshank*mshank*cos(theta0)*cos(theta3)*cos(theta4)*sin(theta1)*sin(theta2)*sin(theta5)*sin(theta6)*sin(theta7) - lshank*mshank*cos(theta0)*cos(theta3)*cos(theta5)*sin(theta1)*sin(theta2)*sin(theta4)*sin(theta6)*sin(theta7))/(4*mshank + 4*mthigh + 2*mtrunk);

JRcom(2,1)=(8*a1*mshank*cos(theta1) - 2*lshank*mshank*cos(theta1 + theta2 + theta3 - theta6 - theta7) + 16*a1*mthigh*cos(theta1) + 8*a1*mtrunk*cos(theta1) + 2*a6*mshank*cos(theta1 + theta2 + theta3 + theta4 - theta5 + theta6) + 2*a6*mshank*cos(theta1 + theta2 + theta3 - theta4 + theta5 + theta6) + 4*lshank*mshank*cos(theta1) - lthigh*mthigh*cos(theta1 + theta2 + theta3 + theta4 - theta5 + theta6) - lthigh*mthigh*cos(theta1 + theta2 + theta3 - theta4 + theta5 + theta6) + 4*a6*mshank*cos(theta1 + theta2 + theta3 - theta6) - 2*lthigh*mthigh*cos(theta1 + theta2 + theta3 - theta6) - 4*a4*mshank*sin(theta1 + theta2 + theta3 - theta4) - 4*a4*mthigh*sin(theta1 + theta2 + theta3 - theta4) + 4*mtrunk*ypelvis*cos(theta1 + theta2 + theta3 - theta4) + 2*lshank*mshank*cos(theta1 + theta2 + theta3 + theta6 + theta7) - 4*mtrunk*xpelvis*sin(theta1 + theta2 + theta3 - theta4) - lshank*mshank*cos(theta1 + theta2 + theta3 + theta4 - theta5 - theta6 - theta7) - lshank*mshank*cos(theta1 + theta2 + theta3 - theta4 + theta5 - theta6 - theta7) + 2*a6*mshank*cos(theta1 + theta2 + theta3 + theta4 - theta5 - theta6) + 2*a6*mshank*cos(theta1 + theta2 + theta3 - theta4 + theta5 - theta6) - lthigh*mthigh*cos(theta1 + theta2 + theta3 + theta4 - theta5 - theta6) - lthigh*mthigh*cos(theta1 + theta2 + theta3 - theta4 + theta5 - theta6) + 8*mtrunk*zpelvis*sin(theta1 + theta2 + theta3) - lshank*mshank*cos(theta1 + theta2 + theta3 + theta4 - theta5 + theta6 + theta7) - lshank*mshank*cos(theta1 + theta2 + theta3 - theta4 + theta5 + theta6 + theta7) + 4*d7*mshank*sin(theta1 + theta2 + theta3 + theta4 - theta5) - 4*d7*mshank*sin(theta1 + theta2 + theta3 - theta4 + theta5) + 4*d7*mthigh*sin(theta1 + theta2 + theta3 + theta4 - theta5) - 4*d7*mthigh*sin(theta1 + theta2 + theta3 - theta4 + theta5) - 4*a6*mshank*cos(theta1 + theta2 + theta3 + theta6) + 2*lthigh*mthigh*cos(theta1 + theta2 + theta3 + theta6) + 4*a4*mshank*sin(theta1 + theta2 + theta3 + theta4) + 4*a4*mthigh*sin(theta1 + theta2 + theta3 + theta4) + 8*a2*mshank*cos(theta1 + theta2) + 8*a2*mthigh*cos(theta1 + theta2) + 8*a2*mtrunk*cos(theta1 + theta2) + 4*mtrunk*ypelvis*cos(theta1 + theta2 + theta3 + theta4) + 4*lthigh*mthigh*cos(theta1 + theta2) + 4*mtrunk*xpelvis*sin(theta1 + theta2 + theta3 + theta4))/(8*(2*mshank + 2*mthigh + mtrunk));
JRcom(2,2)=(2*a6*mshank*cos(theta1 + theta2 + theta3 + theta4 - theta5 + theta6) - 2*lshank*mshank*cos(theta1 + theta2 + theta3 - theta6 - theta7) + 2*a6*mshank*cos(theta1 + theta2 + theta3 - theta4 + theta5 + theta6) - lthigh*mthigh*cos(theta1 + theta2 + theta3 + theta4 - theta5 + theta6) - lthigh*mthigh*cos(theta1 + theta2 + theta3 - theta4 + theta5 + theta6) + 4*a6*mshank*cos(theta1 + theta2 + theta3 - theta6) - 2*lthigh*mthigh*cos(theta1 + theta2 + theta3 - theta6) - 4*a4*mshank*sin(theta1 + theta2 + theta3 - theta4) - 4*a4*mthigh*sin(theta1 + theta2 + theta3 - theta4) + 4*mtrunk*ypelvis*cos(theta1 + theta2 + theta3 - theta4) + 2*lshank*mshank*cos(theta1 + theta2 + theta3 + theta6 + theta7) - 4*mtrunk*xpelvis*sin(theta1 + theta2 + theta3 - theta4) - lshank*mshank*cos(theta1 + theta2 + theta3 + theta4 - theta5 - theta6 - theta7) - lshank*mshank*cos(theta1 + theta2 + theta3 - theta4 + theta5 - theta6 - theta7) + 2*a6*mshank*cos(theta1 + theta2 + theta3 + theta4 - theta5 - theta6) + 2*a6*mshank*cos(theta1 + theta2 + theta3 - theta4 + theta5 - theta6) - lthigh*mthigh*cos(theta1 + theta2 + theta3 + theta4 - theta5 - theta6) - lthigh*mthigh*cos(theta1 + theta2 + theta3 - theta4 + theta5 - theta6) + 8*mtrunk*zpelvis*sin(theta1 + theta2 + theta3) - lshank*mshank*cos(theta1 + theta2 + theta3 + theta4 - theta5 + theta6 + theta7) - lshank*mshank*cos(theta1 + theta2 + theta3 - theta4 + theta5 + theta6 + theta7) + 4*d7*mshank*sin(theta1 + theta2 + theta3 + theta4 - theta5) - 4*d7*mshank*sin(theta1 + theta2 + theta3 - theta4 + theta5) + 4*d7*mthigh*sin(theta1 + theta2 + theta3 + theta4 - theta5) - 4*d7*mthigh*sin(theta1 + theta2 + theta3 - theta4 + theta5) - 4*a6*mshank*cos(theta1 + theta2 + theta3 + theta6) + 2*lthigh*mthigh*cos(theta1 + theta2 + theta3 + theta6) + 4*a4*mshank*sin(theta1 + theta2 + theta3 + theta4) + 4*a4*mthigh*sin(theta1 + theta2 + theta3 + theta4) + 8*a2*mshank*cos(theta1 + theta2) + 8*a2*mthigh*cos(theta1 + theta2) + 8*a2*mtrunk*cos(theta1 + theta2) + 4*mtrunk*ypelvis*cos(theta1 + theta2 + theta3 + theta4) + 4*lthigh*mthigh*cos(theta1 + theta2) + 4*mtrunk*xpelvis*sin(theta1 + theta2 + theta3 + theta4))/(8*(2*mshank + 2*mthigh + mtrunk));
JRcom(2,3)=-(2*lshank*mshank*cos(theta1 + theta2 + theta3 - theta6 - theta7) - 2*a6*mshank*cos(theta1 + theta2 + theta3 + theta4 - theta5 + theta6) - 2*a6*mshank*cos(theta1 + theta2 + theta3 - theta4 + theta5 + theta6) + lthigh*mthigh*cos(theta1 + theta2 + theta3 + theta4 - theta5 + theta6) + lthigh*mthigh*cos(theta1 + theta2 + theta3 - theta4 + theta5 + theta6) - 4*a6*mshank*cos(theta1 + theta2 + theta3 - theta6) + 2*lthigh*mthigh*cos(theta1 + theta2 + theta3 - theta6) + 4*a4*mshank*sin(theta1 + theta2 + theta3 - theta4) + 4*a4*mthigh*sin(theta1 + theta2 + theta3 - theta4) - 4*mtrunk*ypelvis*cos(theta1 + theta2 + theta3 - theta4) - 2*lshank*mshank*cos(theta1 + theta2 + theta3 + theta6 + theta7) + 4*mtrunk*xpelvis*sin(theta1 + theta2 + theta3 - theta4) + lshank*mshank*cos(theta1 + theta2 + theta3 + theta4 - theta5 - theta6 - theta7) + lshank*mshank*cos(theta1 + theta2 + theta3 - theta4 + theta5 - theta6 - theta7) - 2*a6*mshank*cos(theta1 + theta2 + theta3 + theta4 - theta5 - theta6) - 2*a6*mshank*cos(theta1 + theta2 + theta3 - theta4 + theta5 - theta6) + lthigh*mthigh*cos(theta1 + theta2 + theta3 + theta4 - theta5 - theta6) + lthigh*mthigh*cos(theta1 + theta2 + theta3 - theta4 + theta5 - theta6) - 8*mtrunk*zpelvis*sin(theta1 + theta2 + theta3) + lshank*mshank*cos(theta1 + theta2 + theta3 + theta4 - theta5 + theta6 + theta7) + lshank*mshank*cos(theta1 + theta2 + theta3 - theta4 + theta5 + theta6 + theta7) - 4*d7*mshank*sin(theta1 + theta2 + theta3 + theta4 - theta5) + 4*d7*mshank*sin(theta1 + theta2 + theta3 - theta4 + theta5) - 4*d7*mthigh*sin(theta1 + theta2 + theta3 + theta4 - theta5) + 4*d7*mthigh*sin(theta1 + theta2 + theta3 - theta4 + theta5) + 4*a6*mshank*cos(theta1 + theta2 + theta3 + theta6) - 2*lthigh*mthigh*cos(theta1 + theta2 + theta3 + theta6) - 4*a4*mshank*sin(theta1 + theta2 + theta3 + theta4) - 4*a4*mthigh*sin(theta1 + theta2 + theta3 + theta4) - 4*mtrunk*ypelvis*cos(theta1 + theta2 + theta3 + theta4) - 4*mtrunk*xpelvis*sin(theta1 + theta2 + theta3 + theta4))/(8*(2*mshank + 2*mthigh + mtrunk));
JRcom(2,4)=(2*a6*mshank*cos(theta1 + theta2 + theta3 + theta4 - theta5 + theta6) - 2*a6*mshank*cos(theta1 + theta2 + theta3 - theta4 + theta5 + theta6) - lthigh*mthigh*cos(theta1 + theta2 + theta3 + theta4 - theta5 + theta6) + lthigh*mthigh*cos(theta1 + theta2 + theta3 - theta4 + theta5 + theta6) + 4*a4*mshank*sin(theta1 + theta2 + theta3 - theta4) + 4*a4*mthigh*sin(theta1 + theta2 + theta3 - theta4) - 4*mtrunk*ypelvis*cos(theta1 + theta2 + theta3 - theta4) + 4*mtrunk*xpelvis*sin(theta1 + theta2 + theta3 - theta4) - lshank*mshank*cos(theta1 + theta2 + theta3 + theta4 - theta5 - theta6 - theta7) + lshank*mshank*cos(theta1 + theta2 + theta3 - theta4 + theta5 - theta6 - theta7) + 2*a6*mshank*cos(theta1 + theta2 + theta3 + theta4 - theta5 - theta6) - 2*a6*mshank*cos(theta1 + theta2 + theta3 - theta4 + theta5 - theta6) - lthigh*mthigh*cos(theta1 + theta2 + theta3 + theta4 - theta5 - theta6) + lthigh*mthigh*cos(theta1 + theta2 + theta3 - theta4 + theta5 - theta6) - lshank*mshank*cos(theta1 + theta2 + theta3 + theta4 - theta5 + theta6 + theta7) + lshank*mshank*cos(theta1 + theta2 + theta3 - theta4 + theta5 + theta6 + theta7) + 4*d7*mshank*sin(theta1 + theta2 + theta3 + theta4 - theta5) + 4*d7*mshank*sin(theta1 + theta2 + theta3 - theta4 + theta5) + 4*d7*mthigh*sin(theta1 + theta2 + theta3 + theta4 - theta5) + 4*d7*mthigh*sin(theta1 + theta2 + theta3 - theta4 + theta5) + 4*a4*mshank*sin(theta1 + theta2 + theta3 + theta4) + 4*a4*mthigh*sin(theta1 + theta2 + theta3 + theta4) + 4*mtrunk*ypelvis*cos(theta1 + theta2 + theta3 + theta4) + 4*mtrunk*xpelvis*sin(theta1 + theta2 + theta3 + theta4))/(8*(2*mshank + 2*mthigh + mtrunk));

JRcom(3,1)=(lshank*mshank*sin(theta0)*sin(theta1) + 2*a1*mshank*sin(theta0)*sin(theta1) + 4*a1*mthigh*sin(theta0)*sin(theta1) + 2*a1*mtrunk*sin(theta0)*sin(theta1) + 2*a2*mshank*cos(theta1)*sin(theta0)*sin(theta2) + 2*a2*mshank*cos(theta2)*sin(theta0)*sin(theta1) + 2*a2*mthigh*cos(theta1)*sin(theta0)*sin(theta2) + 2*a2*mthigh*cos(theta2)*sin(theta0)*sin(theta1) + 2*a2*mtrunk*cos(theta1)*sin(theta0)*sin(theta2) + 2*a2*mtrunk*cos(theta2)*sin(theta0)*sin(theta1) + lthigh*mthigh*cos(theta1)*sin(theta0)*sin(theta2) + lthigh*mthigh*cos(theta2)*sin(theta0)*sin(theta1) - 2*mtrunk*zpelvis*cos(theta1)*cos(theta2)*cos(theta3)*sin(theta0) + 2*mtrunk*zpelvis*cos(theta1)*sin(theta0)*sin(theta2)*sin(theta3) + 2*mtrunk*zpelvis*cos(theta2)*sin(theta0)*sin(theta1)*sin(theta3) + 2*mtrunk*zpelvis*cos(theta3)*sin(theta0)*sin(theta1)*sin(theta2) - 2*a6*mshank*cos(theta1)*cos(theta2)*cos(theta3)*sin(theta0)*sin(theta6) + lthigh*mthigh*cos(theta1)*cos(theta2)*cos(theta3)*sin(theta0)*sin(theta6) + 2*a4*mshank*cos(theta1)*cos(theta2)*sin(theta0)*sin(theta3)*sin(theta4) + 2*a4*mshank*cos(theta1)*cos(theta3)*sin(theta0)*sin(theta2)*sin(theta4) + 2*a4*mshank*cos(theta2)*cos(theta3)*sin(theta0)*sin(theta1)*sin(theta4) + 2*a4*mthigh*cos(theta1)*cos(theta2)*sin(theta0)*sin(theta3)*sin(theta4) + 2*a4*mthigh*cos(theta1)*cos(theta3)*sin(theta0)*sin(theta2)*sin(theta4) + 2*a4*mthigh*cos(theta2)*cos(theta3)*sin(theta0)*sin(theta1)*sin(theta4) + 2*mtrunk*ypelvis*cos(theta1)*cos(theta2)*cos(theta4)*sin(theta0)*sin(theta3) + 2*mtrunk*ypelvis*cos(theta1)*cos(theta3)*cos(theta4)*sin(theta0)*sin(theta2) + 2*mtrunk*ypelvis*cos(theta2)*cos(theta3)*cos(theta4)*sin(theta0)*sin(theta1) + 2*a6*mshank*cos(theta1)*sin(theta0)*sin(theta2)*sin(theta3)*sin(theta6) + 2*a6*mshank*cos(theta2)*sin(theta0)*sin(theta1)*sin(theta3)*sin(theta6) + 2*a6*mshank*cos(theta3)*sin(theta0)*sin(theta1)*sin(theta2)*sin(theta6) + 2*mtrunk*xpelvis*cos(theta1)*cos(theta2)*sin(theta0)*sin(theta3)*sin(theta4) + 2*mtrunk*xpelvis*cos(theta1)*cos(theta3)*sin(theta0)*sin(theta2)*sin(theta4) + 2*mtrunk*xpelvis*cos(theta2)*cos(theta3)*sin(theta0)*sin(theta1)*sin(theta4) - lthigh*mthigh*cos(theta1)*sin(theta0)*sin(theta2)*sin(theta3)*sin(theta6) - lthigh*mthigh*cos(theta2)*sin(theta0)*sin(theta1)*sin(theta3)*sin(theta6) - lthigh*mthigh*cos(theta3)*sin(theta0)*sin(theta1)*sin(theta2)*sin(theta6) - 2*a4*mshank*sin(theta0)*sin(theta1)*sin(theta2)*sin(theta3)*sin(theta4) - 2*a4*mthigh*sin(theta0)*sin(theta1)*sin(theta2)*sin(theta3)*sin(theta4) - 2*mtrunk*ypelvis*cos(theta4)*sin(theta0)*sin(theta1)*sin(theta2)*sin(theta3) - 2*mtrunk*xpelvis*sin(theta0)*sin(theta1)*sin(theta2)*sin(theta3)*sin(theta4) + lshank*mshank*cos(theta1)*cos(theta2)*cos(theta3)*cos(theta6)*sin(theta0)*sin(theta7) + lshank*mshank*cos(theta1)*cos(theta2)*cos(theta3)*cos(theta7)*sin(theta0)*sin(theta6) - 2*d7*mshank*cos(theta1)*cos(theta2)*cos(theta4)*sin(theta0)*sin(theta3)*sin(theta5) + 2*d7*mshank*cos(theta1)*cos(theta2)*cos(theta5)*sin(theta0)*sin(theta3)*sin(theta4) - 2*d7*mshank*cos(theta1)*cos(theta3)*cos(theta4)*sin(theta0)*sin(theta2)*sin(theta5) + 2*d7*mshank*cos(theta1)*cos(theta3)*cos(theta5)*sin(theta0)*sin(theta2)*sin(theta4) - 2*d7*mshank*cos(theta2)*cos(theta3)*cos(theta4)*sin(theta0)*sin(theta1)*sin(theta5) + 2*d7*mshank*cos(theta2)*cos(theta3)*cos(theta5)*sin(theta0)*sin(theta1)*sin(theta4) - 2*d7*mthigh*cos(theta1)*cos(theta2)*cos(theta4)*sin(theta0)*sin(theta3)*sin(theta5) + 2*d7*mthigh*cos(theta1)*cos(theta2)*cos(theta5)*sin(theta0)*sin(theta3)*sin(theta4) - 2*d7*mthigh*cos(theta1)*cos(theta3)*cos(theta4)*sin(theta0)*sin(theta2)*sin(theta5) + 2*d7*mthigh*cos(theta1)*cos(theta3)*cos(theta5)*sin(theta0)*sin(theta2)*sin(theta4) - 2*d7*mthigh*cos(theta2)*cos(theta3)*cos(theta4)*sin(theta0)*sin(theta1)*sin(theta5) + 2*d7*mthigh*cos(theta2)*cos(theta3)*cos(theta5)*sin(theta0)*sin(theta1)*sin(theta4) - lshank*mshank*cos(theta1)*cos(theta6)*sin(theta0)*sin(theta2)*sin(theta3)*sin(theta7) - lshank*mshank*cos(theta1)*cos(theta7)*sin(theta0)*sin(theta2)*sin(theta3)*sin(theta6) - lshank*mshank*cos(theta2)*cos(theta6)*sin(theta0)*sin(theta1)*sin(theta3)*sin(theta7) - lshank*mshank*cos(theta2)*cos(theta7)*sin(theta0)*sin(theta1)*sin(theta3)*sin(theta6) - lshank*mshank*cos(theta3)*cos(theta6)*sin(theta0)*sin(theta1)*sin(theta2)*sin(theta7) - lshank*mshank*cos(theta3)*cos(theta7)*sin(theta0)*sin(theta1)*sin(theta2)*sin(theta6) + 2*d7*mshank*cos(theta4)*sin(theta0)*sin(theta1)*sin(theta2)*sin(theta3)*sin(theta5) - 2*d7*mshank*cos(theta5)*sin(theta0)*sin(theta1)*sin(theta2)*sin(theta3)*sin(theta4) + 2*d7*mthigh*cos(theta4)*sin(theta0)*sin(theta1)*sin(theta2)*sin(theta3)*sin(theta5) - 2*d7*mthigh*cos(theta5)*sin(theta0)*sin(theta1)*sin(theta2)*sin(theta3)*sin(theta4) + 2*a6*mshank*cos(theta1)*cos(theta2)*cos(theta4)*cos(theta5)*cos(theta6)*sin(theta0)*sin(theta3) + 2*a6*mshank*cos(theta1)*cos(theta3)*cos(theta4)*cos(theta5)*cos(theta6)*sin(theta0)*sin(theta2) + 2*a6*mshank*cos(theta2)*cos(theta3)*cos(theta4)*cos(theta5)*cos(theta6)*sin(theta0)*sin(theta1) - lthigh*mthigh*cos(theta1)*cos(theta2)*cos(theta4)*cos(theta5)*cos(theta6)*sin(theta0)*sin(theta3) - lthigh*mthigh*cos(theta1)*cos(theta3)*cos(theta4)*cos(theta5)*cos(theta6)*sin(theta0)*sin(theta2) - lthigh*mthigh*cos(theta2)*cos(theta3)*cos(theta4)*cos(theta5)*cos(theta6)*sin(theta0)*sin(theta1) + 2*a6*mshank*cos(theta1)*cos(theta2)*cos(theta6)*sin(theta0)*sin(theta3)*sin(theta4)*sin(theta5) + 2*a6*mshank*cos(theta1)*cos(theta3)*cos(theta6)*sin(theta0)*sin(theta2)*sin(theta4)*sin(theta5) + 2*a6*mshank*cos(theta2)*cos(theta3)*cos(theta6)*sin(theta0)*sin(theta1)*sin(theta4)*sin(theta5) - 2*a6*mshank*cos(theta4)*cos(theta5)*cos(theta6)*sin(theta0)*sin(theta1)*sin(theta2)*sin(theta3) - lthigh*mthigh*cos(theta1)*cos(theta2)*cos(theta6)*sin(theta0)*sin(theta3)*sin(theta4)*sin(theta5) - lthigh*mthigh*cos(theta1)*cos(theta3)*cos(theta6)*sin(theta0)*sin(theta2)*sin(theta4)*sin(theta5) - lthigh*mthigh*cos(theta2)*cos(theta3)*cos(theta6)*sin(theta0)*sin(theta1)*sin(theta4)*sin(theta5) + lthigh*mthigh*cos(theta4)*cos(theta5)*cos(theta6)*sin(theta0)*sin(theta1)*sin(theta2)*sin(theta3) - 2*a6*mshank*cos(theta6)*sin(theta0)*sin(theta1)*sin(theta2)*sin(theta3)*sin(theta4)*sin(theta5) + lthigh*mthigh*cos(theta6)*sin(theta0)*sin(theta1)*sin(theta2)*sin(theta3)*sin(theta4)*sin(theta5) - lshank*mshank*cos(theta1)*cos(theta2)*cos(theta4)*cos(theta5)*cos(theta6)*cos(theta7)*sin(theta0)*sin(theta3) - lshank*mshank*cos(theta1)*cos(theta3)*cos(theta4)*cos(theta5)*cos(theta6)*cos(theta7)*sin(theta0)*sin(theta2) - lshank*mshank*cos(theta2)*cos(theta3)*cos(theta4)*cos(theta5)*cos(theta6)*cos(theta7)*sin(theta0)*sin(theta1) + lshank*mshank*cos(theta1)*cos(theta2)*cos(theta4)*cos(theta5)*sin(theta0)*sin(theta3)*sin(theta6)*sin(theta7) - lshank*mshank*cos(theta1)*cos(theta2)*cos(theta6)*cos(theta7)*sin(theta0)*sin(theta3)*sin(theta4)*sin(theta5) + lshank*mshank*cos(theta1)*cos(theta3)*cos(theta4)*cos(theta5)*sin(theta0)*sin(theta2)*sin(theta6)*sin(theta7) - lshank*mshank*cos(theta1)*cos(theta3)*cos(theta6)*cos(theta7)*sin(theta0)*sin(theta2)*sin(theta4)*sin(theta5) + lshank*mshank*cos(theta2)*cos(theta3)*cos(theta4)*cos(theta5)*sin(theta0)*sin(theta1)*sin(theta6)*sin(theta7) - lshank*mshank*cos(theta2)*cos(theta3)*cos(theta6)*cos(theta7)*sin(theta0)*sin(theta1)*sin(theta4)*sin(theta5) + lshank*mshank*cos(theta4)*cos(theta5)*cos(theta6)*cos(theta7)*sin(theta0)*sin(theta1)*sin(theta2)*sin(theta3) + lshank*mshank*cos(theta1)*cos(theta2)*sin(theta0)*sin(theta3)*sin(theta4)*sin(theta5)*sin(theta6)*sin(theta7) + lshank*mshank*cos(theta1)*cos(theta3)*sin(theta0)*sin(theta2)*sin(theta4)*sin(theta5)*sin(theta6)*sin(theta7) + lshank*mshank*cos(theta2)*cos(theta3)*sin(theta0)*sin(theta1)*sin(theta4)*sin(theta5)*sin(theta6)*sin(theta7) - lshank*mshank*cos(theta4)*cos(theta5)*sin(theta0)*sin(theta1)*sin(theta2)*sin(theta3)*sin(theta6)*sin(theta7) + lshank*mshank*cos(theta6)*cos(theta7)*sin(theta0)*sin(theta1)*sin(theta2)*sin(theta3)*sin(theta4)*sin(theta5) - lshank*mshank*sin(theta0)*sin(theta1)*sin(theta2)*sin(theta3)*sin(theta4)*sin(theta5)*sin(theta6)*sin(theta7))/(4*mshank + 4*mthigh + 2*mtrunk);
JRcom(3,2)=(2*a2*mshank*cos(theta1)*sin(theta0)*sin(theta2) + 2*a2*mshank*cos(theta2)*sin(theta0)*sin(theta1) + 2*a2*mthigh*cos(theta1)*sin(theta0)*sin(theta2) + 2*a2*mthigh*cos(theta2)*sin(theta0)*sin(theta1) + 2*a2*mtrunk*cos(theta1)*sin(theta0)*sin(theta2) + 2*a2*mtrunk*cos(theta2)*sin(theta0)*sin(theta1) + lthigh*mthigh*cos(theta1)*sin(theta0)*sin(theta2) + lthigh*mthigh*cos(theta2)*sin(theta0)*sin(theta1) - 2*mtrunk*zpelvis*cos(theta1)*cos(theta2)*cos(theta3)*sin(theta0) + 2*mtrunk*zpelvis*cos(theta1)*sin(theta0)*sin(theta2)*sin(theta3) + 2*mtrunk*zpelvis*cos(theta2)*sin(theta0)*sin(theta1)*sin(theta3) + 2*mtrunk*zpelvis*cos(theta3)*sin(theta0)*sin(theta1)*sin(theta2) - 2*a6*mshank*cos(theta1)*cos(theta2)*cos(theta3)*sin(theta0)*sin(theta6) + lthigh*mthigh*cos(theta1)*cos(theta2)*cos(theta3)*sin(theta0)*sin(theta6) + 2*a4*mshank*cos(theta1)*cos(theta2)*sin(theta0)*sin(theta3)*sin(theta4) + 2*a4*mshank*cos(theta1)*cos(theta3)*sin(theta0)*sin(theta2)*sin(theta4) + 2*a4*mshank*cos(theta2)*cos(theta3)*sin(theta0)*sin(theta1)*sin(theta4) + 2*a4*mthigh*cos(theta1)*cos(theta2)*sin(theta0)*sin(theta3)*sin(theta4) + 2*a4*mthigh*cos(theta1)*cos(theta3)*sin(theta0)*sin(theta2)*sin(theta4) + 2*a4*mthigh*cos(theta2)*cos(theta3)*sin(theta0)*sin(theta1)*sin(theta4) + 2*mtrunk*ypelvis*cos(theta1)*cos(theta2)*cos(theta4)*sin(theta0)*sin(theta3) + 2*mtrunk*ypelvis*cos(theta1)*cos(theta3)*cos(theta4)*sin(theta0)*sin(theta2) + 2*mtrunk*ypelvis*cos(theta2)*cos(theta3)*cos(theta4)*sin(theta0)*sin(theta1) + 2*a6*mshank*cos(theta1)*sin(theta0)*sin(theta2)*sin(theta3)*sin(theta6) + 2*a6*mshank*cos(theta2)*sin(theta0)*sin(theta1)*sin(theta3)*sin(theta6) + 2*a6*mshank*cos(theta3)*sin(theta0)*sin(theta1)*sin(theta2)*sin(theta6) + 2*mtrunk*xpelvis*cos(theta1)*cos(theta2)*sin(theta0)*sin(theta3)*sin(theta4) + 2*mtrunk*xpelvis*cos(theta1)*cos(theta3)*sin(theta0)*sin(theta2)*sin(theta4) + 2*mtrunk*xpelvis*cos(theta2)*cos(theta3)*sin(theta0)*sin(theta1)*sin(theta4) - lthigh*mthigh*cos(theta1)*sin(theta0)*sin(theta2)*sin(theta3)*sin(theta6) - lthigh*mthigh*cos(theta2)*sin(theta0)*sin(theta1)*sin(theta3)*sin(theta6) - lthigh*mthigh*cos(theta3)*sin(theta0)*sin(theta1)*sin(theta2)*sin(theta6) - 2*a4*mshank*sin(theta0)*sin(theta1)*sin(theta2)*sin(theta3)*sin(theta4) - 2*a4*mthigh*sin(theta0)*sin(theta1)*sin(theta2)*sin(theta3)*sin(theta4) - 2*mtrunk*ypelvis*cos(theta4)*sin(theta0)*sin(theta1)*sin(theta2)*sin(theta3) - 2*mtrunk*xpelvis*sin(theta0)*sin(theta1)*sin(theta2)*sin(theta3)*sin(theta4) + lshank*mshank*cos(theta1)*cos(theta2)*cos(theta3)*cos(theta6)*sin(theta0)*sin(theta7) + lshank*mshank*cos(theta1)*cos(theta2)*cos(theta3)*cos(theta7)*sin(theta0)*sin(theta6) - 2*d7*mshank*cos(theta1)*cos(theta2)*cos(theta4)*sin(theta0)*sin(theta3)*sin(theta5) + 2*d7*mshank*cos(theta1)*cos(theta2)*cos(theta5)*sin(theta0)*sin(theta3)*sin(theta4) - 2*d7*mshank*cos(theta1)*cos(theta3)*cos(theta4)*sin(theta0)*sin(theta2)*sin(theta5) + 2*d7*mshank*cos(theta1)*cos(theta3)*cos(theta5)*sin(theta0)*sin(theta2)*sin(theta4) - 2*d7*mshank*cos(theta2)*cos(theta3)*cos(theta4)*sin(theta0)*sin(theta1)*sin(theta5) + 2*d7*mshank*cos(theta2)*cos(theta3)*cos(theta5)*sin(theta0)*sin(theta1)*sin(theta4) - 2*d7*mthigh*cos(theta1)*cos(theta2)*cos(theta4)*sin(theta0)*sin(theta3)*sin(theta5) + 2*d7*mthigh*cos(theta1)*cos(theta2)*cos(theta5)*sin(theta0)*sin(theta3)*sin(theta4) - 2*d7*mthigh*cos(theta1)*cos(theta3)*cos(theta4)*sin(theta0)*sin(theta2)*sin(theta5) + 2*d7*mthigh*cos(theta1)*cos(theta3)*cos(theta5)*sin(theta0)*sin(theta2)*sin(theta4) - 2*d7*mthigh*cos(theta2)*cos(theta3)*cos(theta4)*sin(theta0)*sin(theta1)*sin(theta5) + 2*d7*mthigh*cos(theta2)*cos(theta3)*cos(theta5)*sin(theta0)*sin(theta1)*sin(theta4) - lshank*mshank*cos(theta1)*cos(theta6)*sin(theta0)*sin(theta2)*sin(theta3)*sin(theta7) - lshank*mshank*cos(theta1)*cos(theta7)*sin(theta0)*sin(theta2)*sin(theta3)*sin(theta6) - lshank*mshank*cos(theta2)*cos(theta6)*sin(theta0)*sin(theta1)*sin(theta3)*sin(theta7) - lshank*mshank*cos(theta2)*cos(theta7)*sin(theta0)*sin(theta1)*sin(theta3)*sin(theta6) - lshank*mshank*cos(theta3)*cos(theta6)*sin(theta0)*sin(theta1)*sin(theta2)*sin(theta7) - lshank*mshank*cos(theta3)*cos(theta7)*sin(theta0)*sin(theta1)*sin(theta2)*sin(theta6) + 2*d7*mshank*cos(theta4)*sin(theta0)*sin(theta1)*sin(theta2)*sin(theta3)*sin(theta5) - 2*d7*mshank*cos(theta5)*sin(theta0)*sin(theta1)*sin(theta2)*sin(theta3)*sin(theta4) + 2*d7*mthigh*cos(theta4)*sin(theta0)*sin(theta1)*sin(theta2)*sin(theta3)*sin(theta5) - 2*d7*mthigh*cos(theta5)*sin(theta0)*sin(theta1)*sin(theta2)*sin(theta3)*sin(theta4) + 2*a6*mshank*cos(theta1)*cos(theta2)*cos(theta4)*cos(theta5)*cos(theta6)*sin(theta0)*sin(theta3) + 2*a6*mshank*cos(theta1)*cos(theta3)*cos(theta4)*cos(theta5)*cos(theta6)*sin(theta0)*sin(theta2) + 2*a6*mshank*cos(theta2)*cos(theta3)*cos(theta4)*cos(theta5)*cos(theta6)*sin(theta0)*sin(theta1) - lthigh*mthigh*cos(theta1)*cos(theta2)*cos(theta4)*cos(theta5)*cos(theta6)*sin(theta0)*sin(theta3) - lthigh*mthigh*cos(theta1)*cos(theta3)*cos(theta4)*cos(theta5)*cos(theta6)*sin(theta0)*sin(theta2) - lthigh*mthigh*cos(theta2)*cos(theta3)*cos(theta4)*cos(theta5)*cos(theta6)*sin(theta0)*sin(theta1) + 2*a6*mshank*cos(theta1)*cos(theta2)*cos(theta6)*sin(theta0)*sin(theta3)*sin(theta4)*sin(theta5) + 2*a6*mshank*cos(theta1)*cos(theta3)*cos(theta6)*sin(theta0)*sin(theta2)*sin(theta4)*sin(theta5) + 2*a6*mshank*cos(theta2)*cos(theta3)*cos(theta6)*sin(theta0)*sin(theta1)*sin(theta4)*sin(theta5) - 2*a6*mshank*cos(theta4)*cos(theta5)*cos(theta6)*sin(theta0)*sin(theta1)*sin(theta2)*sin(theta3) - lthigh*mthigh*cos(theta1)*cos(theta2)*cos(theta6)*sin(theta0)*sin(theta3)*sin(theta4)*sin(theta5) - lthigh*mthigh*cos(theta1)*cos(theta3)*cos(theta6)*sin(theta0)*sin(theta2)*sin(theta4)*sin(theta5) - lthigh*mthigh*cos(theta2)*cos(theta3)*cos(theta6)*sin(theta0)*sin(theta1)*sin(theta4)*sin(theta5) + lthigh*mthigh*cos(theta4)*cos(theta5)*cos(theta6)*sin(theta0)*sin(theta1)*sin(theta2)*sin(theta3) - 2*a6*mshank*cos(theta6)*sin(theta0)*sin(theta1)*sin(theta2)*sin(theta3)*sin(theta4)*sin(theta5) + lthigh*mthigh*cos(theta6)*sin(theta0)*sin(theta1)*sin(theta2)*sin(theta3)*sin(theta4)*sin(theta5) - lshank*mshank*cos(theta1)*cos(theta2)*cos(theta4)*cos(theta5)*cos(theta6)*cos(theta7)*sin(theta0)*sin(theta3) - lshank*mshank*cos(theta1)*cos(theta3)*cos(theta4)*cos(theta5)*cos(theta6)*cos(theta7)*sin(theta0)*sin(theta2) - lshank*mshank*cos(theta2)*cos(theta3)*cos(theta4)*cos(theta5)*cos(theta6)*cos(theta7)*sin(theta0)*sin(theta1) + lshank*mshank*cos(theta1)*cos(theta2)*cos(theta4)*cos(theta5)*sin(theta0)*sin(theta3)*sin(theta6)*sin(theta7) - lshank*mshank*cos(theta1)*cos(theta2)*cos(theta6)*cos(theta7)*sin(theta0)*sin(theta3)*sin(theta4)*sin(theta5) + lshank*mshank*cos(theta1)*cos(theta3)*cos(theta4)*cos(theta5)*sin(theta0)*sin(theta2)*sin(theta6)*sin(theta7) - lshank*mshank*cos(theta1)*cos(theta3)*cos(theta6)*cos(theta7)*sin(theta0)*sin(theta2)*sin(theta4)*sin(theta5) + lshank*mshank*cos(theta2)*cos(theta3)*cos(theta4)*cos(theta5)*sin(theta0)*sin(theta1)*sin(theta6)*sin(theta7) - lshank*mshank*cos(theta2)*cos(theta3)*cos(theta6)*cos(theta7)*sin(theta0)*sin(theta1)*sin(theta4)*sin(theta5) + lshank*mshank*cos(theta4)*cos(theta5)*cos(theta6)*cos(theta7)*sin(theta0)*sin(theta1)*sin(theta2)*sin(theta3) + lshank*mshank*cos(theta1)*cos(theta2)*sin(theta0)*sin(theta3)*sin(theta4)*sin(theta5)*sin(theta6)*sin(theta7) + lshank*mshank*cos(theta1)*cos(theta3)*sin(theta0)*sin(theta2)*sin(theta4)*sin(theta5)*sin(theta6)*sin(theta7) + lshank*mshank*cos(theta2)*cos(theta3)*sin(theta0)*sin(theta1)*sin(theta4)*sin(theta5)*sin(theta6)*sin(theta7) - lshank*mshank*cos(theta4)*cos(theta5)*sin(theta0)*sin(theta1)*sin(theta2)*sin(theta3)*sin(theta6)*sin(theta7) + lshank*mshank*cos(theta6)*cos(theta7)*sin(theta0)*sin(theta1)*sin(theta2)*sin(theta3)*sin(theta4)*sin(theta5) - lshank*mshank*sin(theta0)*sin(theta1)*sin(theta2)*sin(theta3)*sin(theta4)*sin(theta5)*sin(theta6)*sin(theta7))/(4*mshank + 4*mthigh + 2*mtrunk);
JRcom(3,3)=(2*mtrunk*zpelvis*cos(theta1)*sin(theta0)*sin(theta2)*sin(theta3) - 2*mtrunk*zpelvis*cos(theta1)*cos(theta2)*cos(theta3)*sin(theta0) + 2*mtrunk*zpelvis*cos(theta2)*sin(theta0)*sin(theta1)*sin(theta3) + 2*mtrunk*zpelvis*cos(theta3)*sin(theta0)*sin(theta1)*sin(theta2) - 2*a6*mshank*cos(theta1)*cos(theta2)*cos(theta3)*sin(theta0)*sin(theta6) + lthigh*mthigh*cos(theta1)*cos(theta2)*cos(theta3)*sin(theta0)*sin(theta6) + 2*a4*mshank*cos(theta1)*cos(theta2)*sin(theta0)*sin(theta3)*sin(theta4) + 2*a4*mshank*cos(theta1)*cos(theta3)*sin(theta0)*sin(theta2)*sin(theta4) + 2*a4*mshank*cos(theta2)*cos(theta3)*sin(theta0)*sin(theta1)*sin(theta4) + 2*a4*mthigh*cos(theta1)*cos(theta2)*sin(theta0)*sin(theta3)*sin(theta4) + 2*a4*mthigh*cos(theta1)*cos(theta3)*sin(theta0)*sin(theta2)*sin(theta4) + 2*a4*mthigh*cos(theta2)*cos(theta3)*sin(theta0)*sin(theta1)*sin(theta4) + 2*mtrunk*ypelvis*cos(theta1)*cos(theta2)*cos(theta4)*sin(theta0)*sin(theta3) + 2*mtrunk*ypelvis*cos(theta1)*cos(theta3)*cos(theta4)*sin(theta0)*sin(theta2) + 2*mtrunk*ypelvis*cos(theta2)*cos(theta3)*cos(theta4)*sin(theta0)*sin(theta1) + 2*a6*mshank*cos(theta1)*sin(theta0)*sin(theta2)*sin(theta3)*sin(theta6) + 2*a6*mshank*cos(theta2)*sin(theta0)*sin(theta1)*sin(theta3)*sin(theta6) + 2*a6*mshank*cos(theta3)*sin(theta0)*sin(theta1)*sin(theta2)*sin(theta6) + 2*mtrunk*xpelvis*cos(theta1)*cos(theta2)*sin(theta0)*sin(theta3)*sin(theta4) + 2*mtrunk*xpelvis*cos(theta1)*cos(theta3)*sin(theta0)*sin(theta2)*sin(theta4) + 2*mtrunk*xpelvis*cos(theta2)*cos(theta3)*sin(theta0)*sin(theta1)*sin(theta4) - lthigh*mthigh*cos(theta1)*sin(theta0)*sin(theta2)*sin(theta3)*sin(theta6) - lthigh*mthigh*cos(theta2)*sin(theta0)*sin(theta1)*sin(theta3)*sin(theta6) - lthigh*mthigh*cos(theta3)*sin(theta0)*sin(theta1)*sin(theta2)*sin(theta6) - 2*a4*mshank*sin(theta0)*sin(theta1)*sin(theta2)*sin(theta3)*sin(theta4) - 2*a4*mthigh*sin(theta0)*sin(theta1)*sin(theta2)*sin(theta3)*sin(theta4) - 2*mtrunk*ypelvis*cos(theta4)*sin(theta0)*sin(theta1)*sin(theta2)*sin(theta3) - 2*mtrunk*xpelvis*sin(theta0)*sin(theta1)*sin(theta2)*sin(theta3)*sin(theta4) + lshank*mshank*cos(theta1)*cos(theta2)*cos(theta3)*cos(theta6)*sin(theta0)*sin(theta7) + lshank*mshank*cos(theta1)*cos(theta2)*cos(theta3)*cos(theta7)*sin(theta0)*sin(theta6) - 2*d7*mshank*cos(theta1)*cos(theta2)*cos(theta4)*sin(theta0)*sin(theta3)*sin(theta5) + 2*d7*mshank*cos(theta1)*cos(theta2)*cos(theta5)*sin(theta0)*sin(theta3)*sin(theta4) - 2*d7*mshank*cos(theta1)*cos(theta3)*cos(theta4)*sin(theta0)*sin(theta2)*sin(theta5) + 2*d7*mshank*cos(theta1)*cos(theta3)*cos(theta5)*sin(theta0)*sin(theta2)*sin(theta4) - 2*d7*mshank*cos(theta2)*cos(theta3)*cos(theta4)*sin(theta0)*sin(theta1)*sin(theta5) + 2*d7*mshank*cos(theta2)*cos(theta3)*cos(theta5)*sin(theta0)*sin(theta1)*sin(theta4) - 2*d7*mthigh*cos(theta1)*cos(theta2)*cos(theta4)*sin(theta0)*sin(theta3)*sin(theta5) + 2*d7*mthigh*cos(theta1)*cos(theta2)*cos(theta5)*sin(theta0)*sin(theta3)*sin(theta4) - 2*d7*mthigh*cos(theta1)*cos(theta3)*cos(theta4)*sin(theta0)*sin(theta2)*sin(theta5) + 2*d7*mthigh*cos(theta1)*cos(theta3)*cos(theta5)*sin(theta0)*sin(theta2)*sin(theta4) - 2*d7*mthigh*cos(theta2)*cos(theta3)*cos(theta4)*sin(theta0)*sin(theta1)*sin(theta5) + 2*d7*mthigh*cos(theta2)*cos(theta3)*cos(theta5)*sin(theta0)*sin(theta1)*sin(theta4) - lshank*mshank*cos(theta1)*cos(theta6)*sin(theta0)*sin(theta2)*sin(theta3)*sin(theta7) - lshank*mshank*cos(theta1)*cos(theta7)*sin(theta0)*sin(theta2)*sin(theta3)*sin(theta6) - lshank*mshank*cos(theta2)*cos(theta6)*sin(theta0)*sin(theta1)*sin(theta3)*sin(theta7) - lshank*mshank*cos(theta2)*cos(theta7)*sin(theta0)*sin(theta1)*sin(theta3)*sin(theta6) - lshank*mshank*cos(theta3)*cos(theta6)*sin(theta0)*sin(theta1)*sin(theta2)*sin(theta7) - lshank*mshank*cos(theta3)*cos(theta7)*sin(theta0)*sin(theta1)*sin(theta2)*sin(theta6) + 2*d7*mshank*cos(theta4)*sin(theta0)*sin(theta1)*sin(theta2)*sin(theta3)*sin(theta5) - 2*d7*mshank*cos(theta5)*sin(theta0)*sin(theta1)*sin(theta2)*sin(theta3)*sin(theta4) + 2*d7*mthigh*cos(theta4)*sin(theta0)*sin(theta1)*sin(theta2)*sin(theta3)*sin(theta5) - 2*d7*mthigh*cos(theta5)*sin(theta0)*sin(theta1)*sin(theta2)*sin(theta3)*sin(theta4) + 2*a6*mshank*cos(theta1)*cos(theta2)*cos(theta4)*cos(theta5)*cos(theta6)*sin(theta0)*sin(theta3) + 2*a6*mshank*cos(theta1)*cos(theta3)*cos(theta4)*cos(theta5)*cos(theta6)*sin(theta0)*sin(theta2) + 2*a6*mshank*cos(theta2)*cos(theta3)*cos(theta4)*cos(theta5)*cos(theta6)*sin(theta0)*sin(theta1) - lthigh*mthigh*cos(theta1)*cos(theta2)*cos(theta4)*cos(theta5)*cos(theta6)*sin(theta0)*sin(theta3) - lthigh*mthigh*cos(theta1)*cos(theta3)*cos(theta4)*cos(theta5)*cos(theta6)*sin(theta0)*sin(theta2) - lthigh*mthigh*cos(theta2)*cos(theta3)*cos(theta4)*cos(theta5)*cos(theta6)*sin(theta0)*sin(theta1) + 2*a6*mshank*cos(theta1)*cos(theta2)*cos(theta6)*sin(theta0)*sin(theta3)*sin(theta4)*sin(theta5) + 2*a6*mshank*cos(theta1)*cos(theta3)*cos(theta6)*sin(theta0)*sin(theta2)*sin(theta4)*sin(theta5) + 2*a6*mshank*cos(theta2)*cos(theta3)*cos(theta6)*sin(theta0)*sin(theta1)*sin(theta4)*sin(theta5) - 2*a6*mshank*cos(theta4)*cos(theta5)*cos(theta6)*sin(theta0)*sin(theta1)*sin(theta2)*sin(theta3) - lthigh*mthigh*cos(theta1)*cos(theta2)*cos(theta6)*sin(theta0)*sin(theta3)*sin(theta4)*sin(theta5) - lthigh*mthigh*cos(theta1)*cos(theta3)*cos(theta6)*sin(theta0)*sin(theta2)*sin(theta4)*sin(theta5) - lthigh*mthigh*cos(theta2)*cos(theta3)*cos(theta6)*sin(theta0)*sin(theta1)*sin(theta4)*sin(theta5) + lthigh*mthigh*cos(theta4)*cos(theta5)*cos(theta6)*sin(theta0)*sin(theta1)*sin(theta2)*sin(theta3) - 2*a6*mshank*cos(theta6)*sin(theta0)*sin(theta1)*sin(theta2)*sin(theta3)*sin(theta4)*sin(theta5) + lthigh*mthigh*cos(theta6)*sin(theta0)*sin(theta1)*sin(theta2)*sin(theta3)*sin(theta4)*sin(theta5) - lshank*mshank*cos(theta1)*cos(theta2)*cos(theta4)*cos(theta5)*cos(theta6)*cos(theta7)*sin(theta0)*sin(theta3) - lshank*mshank*cos(theta1)*cos(theta3)*cos(theta4)*cos(theta5)*cos(theta6)*cos(theta7)*sin(theta0)*sin(theta2) - lshank*mshank*cos(theta2)*cos(theta3)*cos(theta4)*cos(theta5)*cos(theta6)*cos(theta7)*sin(theta0)*sin(theta1) + lshank*mshank*cos(theta1)*cos(theta2)*cos(theta4)*cos(theta5)*sin(theta0)*sin(theta3)*sin(theta6)*sin(theta7) - lshank*mshank*cos(theta1)*cos(theta2)*cos(theta6)*cos(theta7)*sin(theta0)*sin(theta3)*sin(theta4)*sin(theta5) + lshank*mshank*cos(theta1)*cos(theta3)*cos(theta4)*cos(theta5)*sin(theta0)*sin(theta2)*sin(theta6)*sin(theta7) - lshank*mshank*cos(theta1)*cos(theta3)*cos(theta6)*cos(theta7)*sin(theta0)*sin(theta2)*sin(theta4)*sin(theta5) + lshank*mshank*cos(theta2)*cos(theta3)*cos(theta4)*cos(theta5)*sin(theta0)*sin(theta1)*sin(theta6)*sin(theta7) - lshank*mshank*cos(theta2)*cos(theta3)*cos(theta6)*cos(theta7)*sin(theta0)*sin(theta1)*sin(theta4)*sin(theta5) + lshank*mshank*cos(theta4)*cos(theta5)*cos(theta6)*cos(theta7)*sin(theta0)*sin(theta1)*sin(theta2)*sin(theta3) + lshank*mshank*cos(theta1)*cos(theta2)*sin(theta0)*sin(theta3)*sin(theta4)*sin(theta5)*sin(theta6)*sin(theta7) + lshank*mshank*cos(theta1)*cos(theta3)*sin(theta0)*sin(theta2)*sin(theta4)*sin(theta5)*sin(theta6)*sin(theta7) + lshank*mshank*cos(theta2)*cos(theta3)*sin(theta0)*sin(theta1)*sin(theta4)*sin(theta5)*sin(theta6)*sin(theta7) - lshank*mshank*cos(theta4)*cos(theta5)*sin(theta0)*sin(theta1)*sin(theta2)*sin(theta3)*sin(theta6)*sin(theta7) + lshank*mshank*cos(theta6)*cos(theta7)*sin(theta0)*sin(theta1)*sin(theta2)*sin(theta3)*sin(theta4)*sin(theta5) - lshank*mshank*sin(theta0)*sin(theta1)*sin(theta2)*sin(theta3)*sin(theta4)*sin(theta5)*sin(theta6)*sin(theta7))/(4*mshank + 4*mthigh + 2*mtrunk);
JRcom(3,4)=(2*mtrunk*xpelvis*cos(theta0)*sin(theta4) + 2*a4*mshank*cos(theta0)*sin(theta4) + 2*a4*mthigh*cos(theta0)*sin(theta4) + 2*mtrunk*ypelvis*cos(theta0)*cos(theta4) - 2*d7*mshank*cos(theta0)*cos(theta4)*sin(theta5) + 2*d7*mshank*cos(theta0)*cos(theta5)*sin(theta4) - 2*d7*mthigh*cos(theta0)*cos(theta4)*sin(theta5) + 2*d7*mthigh*cos(theta0)*cos(theta5)*sin(theta4) + 2*a6*mshank*cos(theta0)*cos(theta4)*cos(theta5)*cos(theta6) - lthigh*mthigh*cos(theta0)*cos(theta4)*cos(theta5)*cos(theta6) + 2*a6*mshank*cos(theta0)*cos(theta6)*sin(theta4)*sin(theta5) - lthigh*mthigh*cos(theta0)*cos(theta6)*sin(theta4)*sin(theta5) - lshank*mshank*cos(theta0)*cos(theta4)*cos(theta5)*cos(theta6)*cos(theta7) - 2*a4*mshank*cos(theta1)*cos(theta2)*cos(theta3)*cos(theta4)*sin(theta0) - 2*a4*mthigh*cos(theta1)*cos(theta2)*cos(theta3)*cos(theta4)*sin(theta0) - 2*mtrunk*xpelvis*cos(theta1)*cos(theta2)*cos(theta3)*cos(theta4)*sin(theta0) + lshank*mshank*cos(theta0)*cos(theta4)*cos(theta5)*sin(theta6)*sin(theta7) - lshank*mshank*cos(theta0)*cos(theta6)*cos(theta7)*sin(theta4)*sin(theta5) + 2*a4*mshank*cos(theta1)*cos(theta4)*sin(theta0)*sin(theta2)*sin(theta3) + 2*a4*mshank*cos(theta2)*cos(theta4)*sin(theta0)*sin(theta1)*sin(theta3) + 2*a4*mshank*cos(theta3)*cos(theta4)*sin(theta0)*sin(theta1)*sin(theta2) + 2*a4*mthigh*cos(theta1)*cos(theta4)*sin(theta0)*sin(theta2)*sin(theta3) + 2*a4*mthigh*cos(theta2)*cos(theta4)*sin(theta0)*sin(theta1)*sin(theta3) + 2*a4*mthigh*cos(theta3)*cos(theta4)*sin(theta0)*sin(theta1)*sin(theta2) + 2*mtrunk*ypelvis*cos(theta1)*cos(theta2)*cos(theta3)*sin(theta0)*sin(theta4) + 2*mtrunk*xpelvis*cos(theta1)*cos(theta4)*sin(theta0)*sin(theta2)*sin(theta3) + 2*mtrunk*xpelvis*cos(theta2)*cos(theta4)*sin(theta0)*sin(theta1)*sin(theta3) + 2*mtrunk*xpelvis*cos(theta3)*cos(theta4)*sin(theta0)*sin(theta1)*sin(theta2) + lshank*mshank*cos(theta0)*sin(theta4)*sin(theta5)*sin(theta6)*sin(theta7) - 2*mtrunk*ypelvis*cos(theta1)*sin(theta0)*sin(theta2)*sin(theta3)*sin(theta4) - 2*mtrunk*ypelvis*cos(theta2)*sin(theta0)*sin(theta1)*sin(theta3)*sin(theta4) - 2*mtrunk*ypelvis*cos(theta3)*sin(theta0)*sin(theta1)*sin(theta2)*sin(theta4) - 2*d7*mshank*cos(theta1)*cos(theta2)*cos(theta3)*cos(theta4)*cos(theta5)*sin(theta0) - 2*d7*mthigh*cos(theta1)*cos(theta2)*cos(theta3)*cos(theta4)*cos(theta5)*sin(theta0) - 2*d7*mshank*cos(theta1)*cos(theta2)*cos(theta3)*sin(theta0)*sin(theta4)*sin(theta5) + 2*d7*mshank*cos(theta1)*cos(theta4)*cos(theta5)*sin(theta0)*sin(theta2)*sin(theta3) + 2*d7*mshank*cos(theta2)*cos(theta4)*cos(theta5)*sin(theta0)*sin(theta1)*sin(theta3) + 2*d7*mshank*cos(theta3)*cos(theta4)*cos(theta5)*sin(theta0)*sin(theta1)*sin(theta2) - 2*d7*mthigh*cos(theta1)*cos(theta2)*cos(theta3)*sin(theta0)*sin(theta4)*sin(theta5) + 2*d7*mthigh*cos(theta1)*cos(theta4)*cos(theta5)*sin(theta0)*sin(theta2)*sin(theta3) + 2*d7*mthigh*cos(theta2)*cos(theta4)*cos(theta5)*sin(theta0)*sin(theta1)*sin(theta3) + 2*d7*mthigh*cos(theta3)*cos(theta4)*cos(theta5)*sin(theta0)*sin(theta1)*sin(theta2) + 2*d7*mshank*cos(theta1)*sin(theta0)*sin(theta2)*sin(theta3)*sin(theta4)*sin(theta5) + 2*d7*mshank*cos(theta2)*sin(theta0)*sin(theta1)*sin(theta3)*sin(theta4)*sin(theta5) + 2*d7*mshank*cos(theta3)*sin(theta0)*sin(theta1)*sin(theta2)*sin(theta4)*sin(theta5) + 2*d7*mthigh*cos(theta1)*sin(theta0)*sin(theta2)*sin(theta3)*sin(theta4)*sin(theta5) + 2*d7*mthigh*cos(theta2)*sin(theta0)*sin(theta1)*sin(theta3)*sin(theta4)*sin(theta5) + 2*d7*mthigh*cos(theta3)*sin(theta0)*sin(theta1)*sin(theta2)*sin(theta4)*sin(theta5) - 2*a6*mshank*cos(theta1)*cos(theta2)*cos(theta3)*cos(theta4)*cos(theta6)*sin(theta0)*sin(theta5) + 2*a6*mshank*cos(theta1)*cos(theta2)*cos(theta3)*cos(theta5)*cos(theta6)*sin(theta0)*sin(theta4) + lthigh*mthigh*cos(theta1)*cos(theta2)*cos(theta3)*cos(theta4)*cos(theta6)*sin(theta0)*sin(theta5) - lthigh*mthigh*cos(theta1)*cos(theta2)*cos(theta3)*cos(theta5)*cos(theta6)*sin(theta0)*sin(theta4) + 2*a6*mshank*cos(theta1)*cos(theta4)*cos(theta6)*sin(theta0)*sin(theta2)*sin(theta3)*sin(theta5) - 2*a6*mshank*cos(theta1)*cos(theta5)*cos(theta6)*sin(theta0)*sin(theta2)*sin(theta3)*sin(theta4) + 2*a6*mshank*cos(theta2)*cos(theta4)*cos(theta6)*sin(theta0)*sin(theta1)*sin(theta3)*sin(theta5) - 2*a6*mshank*cos(theta2)*cos(theta5)*cos(theta6)*sin(theta0)*sin(theta1)*sin(theta3)*sin(theta4) + 2*a6*mshank*cos(theta3)*cos(theta4)*cos(theta6)*sin(theta0)*sin(theta1)*sin(theta2)*sin(theta5) - 2*a6*mshank*cos(theta3)*cos(theta5)*cos(theta6)*sin(theta0)*sin(theta1)*sin(theta2)*sin(theta4) - lthigh*mthigh*cos(theta1)*cos(theta4)*cos(theta6)*sin(theta0)*sin(theta2)*sin(theta3)*sin(theta5) + lthigh*mthigh*cos(theta1)*cos(theta5)*cos(theta6)*sin(theta0)*sin(theta2)*sin(theta3)*sin(theta4) - lthigh*mthigh*cos(theta2)*cos(theta4)*cos(theta6)*sin(theta0)*sin(theta1)*sin(theta3)*sin(theta5) + lthigh*mthigh*cos(theta2)*cos(theta5)*cos(theta6)*sin(theta0)*sin(theta1)*sin(theta3)*sin(theta4) - lthigh*mthigh*cos(theta3)*cos(theta4)*cos(theta6)*sin(theta0)*sin(theta1)*sin(theta2)*sin(theta5) + lthigh*mthigh*cos(theta3)*cos(theta5)*cos(theta6)*sin(theta0)*sin(theta1)*sin(theta2)*sin(theta4) + lshank*mshank*cos(theta1)*cos(theta2)*cos(theta3)*cos(theta4)*cos(theta6)*cos(theta7)*sin(theta0)*sin(theta5) - lshank*mshank*cos(theta1)*cos(theta2)*cos(theta3)*cos(theta5)*cos(theta6)*cos(theta7)*sin(theta0)*sin(theta4) - lshank*mshank*cos(theta1)*cos(theta2)*cos(theta3)*cos(theta4)*sin(theta0)*sin(theta5)*sin(theta6)*sin(theta7) + lshank*mshank*cos(theta1)*cos(theta2)*cos(theta3)*cos(theta5)*sin(theta0)*sin(theta4)*sin(theta6)*sin(theta7) - lshank*mshank*cos(theta1)*cos(theta4)*cos(theta6)*cos(theta7)*sin(theta0)*sin(theta2)*sin(theta3)*sin(theta5) + lshank*mshank*cos(theta1)*cos(theta5)*cos(theta6)*cos(theta7)*sin(theta0)*sin(theta2)*sin(theta3)*sin(theta4) - lshank*mshank*cos(theta2)*cos(theta4)*cos(theta6)*cos(theta7)*sin(theta0)*sin(theta1)*sin(theta3)*sin(theta5) + lshank*mshank*cos(theta2)*cos(theta5)*cos(theta6)*cos(theta7)*sin(theta0)*sin(theta1)*sin(theta3)*sin(theta4) - lshank*mshank*cos(theta3)*cos(theta4)*cos(theta6)*cos(theta7)*sin(theta0)*sin(theta1)*sin(theta2)*sin(theta5) + lshank*mshank*cos(theta3)*cos(theta5)*cos(theta6)*cos(theta7)*sin(theta0)*sin(theta1)*sin(theta2)*sin(theta4) + lshank*mshank*cos(theta1)*cos(theta4)*sin(theta0)*sin(theta2)*sin(theta3)*sin(theta5)*sin(theta6)*sin(theta7) - lshank*mshank*cos(theta1)*cos(theta5)*sin(theta0)*sin(theta2)*sin(theta3)*sin(theta4)*sin(theta6)*sin(theta7) + lshank*mshank*cos(theta2)*cos(theta4)*sin(theta0)*sin(theta1)*sin(theta3)*sin(theta5)*sin(theta6)*sin(theta7) - lshank*mshank*cos(theta2)*cos(theta5)*sin(theta0)*sin(theta1)*sin(theta3)*sin(theta4)*sin(theta6)*sin(theta7) + lshank*mshank*cos(theta3)*cos(theta4)*sin(theta0)*sin(theta1)*sin(theta2)*sin(theta5)*sin(theta6)*sin(theta7) - lshank*mshank*cos(theta3)*cos(theta5)*sin(theta0)*sin(theta1)*sin(theta2)*sin(theta4)*sin(theta6)*sin(theta7))/(4*mshank + 4*mthigh + 2*mtrunk);

    %CoM jacobian left foot repere
    
% JLcom(1,5)= sin(theta9)*(- a4*sin(theta5) + xcom*sin(theta5) + ycom*cos(theta5)) + cos(theta6 + theta7 + theta8)*cos(theta9)*( - ycom*sin(theta5) - a4*cos(theta5) + xcom*cos(theta5));
% JLcom(1,6)= - sin(theta6 + theta7 + theta8)*cos(theta9)*(ycom*cos(theta5) - a4*sin(theta5) + xcom*sin(theta5)) + zcom*cos(theta6 + theta7 + theta8)*cos(theta9);
% JLcom(1,7)= - sin(theta6 + theta7 + theta8)*cos(theta9)*(ycom*cos(theta5) - a4*sin(theta5) + xcom*sin(theta5)) + zcom*cos(theta6 + theta7 + theta8)*cos(theta9) - a6*sin(theta7)*cos(theta8)*cos(theta9) + a6*cos(theta9)*cos(theta7)*sin(theta8);
% JLcom(1,8)= a7*sin(theta8)*cos(theta9) - sin(theta6 + theta7 + theta8)*cos(theta9)*(ycom*cos(theta5) - a4*sin(theta5) + xcom*sin(theta5)) + zcom*cos(theta6 + theta7 + theta8)*cos(theta9) + a6*cos(theta7)*sin(theta8)*cos(theta9) + a6*cos(theta9)*sin(theta7)*cos(theta8);
% 
% JLcom(2,5)= - sin(theta6 + theta7 + theta8)*( - ycom*sin(theta5) - a4*cos(theta5) + xcom*cos(theta5));
% JLcom(2,6)= - cos(theta6 + theta7 + theta8)*(ycom*cos(theta5) - a4*sin(theta5) + xcom*sin(theta5)) - zcom*sin(theta6 + theta7 + theta8);
% JLcom(2,7)= - cos(theta6 + theta7 + theta8)*(ycom*cos(theta5) - a4*sin(theta5) + xcom*sin(theta5)) - zcom*sin(theta6 + theta7 + theta8) - a6*sin(theta7)*sin(theta8) + a6*cos(theta8)*cos(theta7);
% JLcom(2,8)= a7*cos(theta8) - cos(theta6 + theta7 + theta8)*(ycom*cos(theta5) - a4*sin(theta5) + xcom*sin(theta5)) - zcom*sin(theta6 + theta7 + theta8) + a6*cos(theta7)*cos(theta8) - a6*sin(theta8)*sin(theta7);
% 
% JLcom(3,5)=cos(theta6 + theta7 + theta8)*sin(theta9)*( - ycom*sin(theta5) - a4*cos(theta5) + xcom*cos(theta5)) - cos(theta9)*( - a4*sin(theta5) + xcom*sin(theta5) + ycom*cos(theta5));
% JLcom(3,6)= - sin(theta6 + theta7 + theta8)*sin(theta9)*(ycom*cos(theta5) - a4*sin(theta5) + xcom*sin(theta5)) + zcom*cos(theta6 + theta7 + theta8)*sin(theta9);
% JLcom(3,7)= - sin(theta6 + theta7 + theta8)*sin(theta9)*(ycom*cos(theta5) - a4*sin(theta5) + xcom*sin(theta5)) + zcom*cos(theta6 + theta7 + theta8)*sin(theta9) + a6*sin(theta7)*cos(theta8)*sin(theta9) + a6*cos(theta7)*sin(theta8)*sin(theta9);
% JLcom(3,8)= - sin(theta6 + theta7 + theta8)*sin(theta9)*(ycom*cos(theta5) - a4*sin(theta5) + xcom*sin(theta5)) + a7*sin(theta8)*sin(theta9) + zcom*cos(theta6 + theta7 + theta8)*sin(theta9) + a6*cos(theta7)*sin(theta8)*sin(theta9) + a6*sin(theta7)*cos(theta8)*sin(theta9);

JLcom(1,5)=(2*a4*mshank*sin(theta5)*sin(theta9) - 2*mtrunk*xpelvis*sin(theta5)*sin(theta9) - 2*mtrunk*ypelvis*cos(theta5)*sin(theta9) + 2*a4*mthigh*sin(theta5)*sin(theta9) + 2*a4*mtrunk*sin(theta5)*sin(theta9) - 2*d3*mshank*cos(theta4)*sin(theta5)*sin(theta9) + 2*d3*mshank*cos(theta5)*sin(theta4)*sin(theta9) - 2*d3*mthigh*cos(theta4)*sin(theta5)*sin(theta9) + 2*d3*mthigh*cos(theta5)*sin(theta4)*sin(theta9) + 2*a2*mshank*cos(theta3)*cos(theta4)*cos(theta5)*sin(theta9) + 2*a2*mthigh*cos(theta3)*cos(theta4)*cos(theta5)*sin(theta9) - lthigh*mthigh*cos(theta3)*cos(theta4)*cos(theta5)*sin(theta9) + 2*a2*mshank*cos(theta3)*sin(theta4)*sin(theta5)*sin(theta9) + 2*a2*mthigh*cos(theta3)*sin(theta4)*sin(theta5)*sin(theta9) - lthigh*mthigh*cos(theta3)*sin(theta4)*sin(theta5)*sin(theta9) - 2*a4*mshank*cos(theta5)*cos(theta6)*cos(theta7)*cos(theta8)*cos(theta9) - 2*a4*mthigh*cos(theta5)*cos(theta6)*cos(theta7)*cos(theta8)*cos(theta9) - 2*a4*mtrunk*cos(theta5)*cos(theta6)*cos(theta7)*cos(theta8)*cos(theta9) + 2*a1*mshank*cos(theta2)*cos(theta3)*cos(theta4)*cos(theta5)*sin(theta9) + 2*mtrunk*xpelvis*cos(theta5)*cos(theta6)*cos(theta7)*cos(theta8)*cos(theta9) - lshank*mshank*cos(theta2)*cos(theta3)*cos(theta4)*cos(theta5)*sin(theta9) + 2*a4*mshank*cos(theta5)*cos(theta6)*cos(theta9)*sin(theta7)*sin(theta8) + 2*a4*mshank*cos(theta5)*cos(theta7)*cos(theta9)*sin(theta6)*sin(theta8) + 2*a4*mshank*cos(theta5)*cos(theta8)*cos(theta9)*sin(theta6)*sin(theta7) + 2*a4*mthigh*cos(theta5)*cos(theta6)*cos(theta9)*sin(theta7)*sin(theta8) + 2*a4*mthigh*cos(theta5)*cos(theta7)*cos(theta9)*sin(theta6)*sin(theta8) + 2*a4*mthigh*cos(theta5)*cos(theta8)*cos(theta9)*sin(theta6)*sin(theta7) + 2*a4*mtrunk*cos(theta5)*cos(theta6)*cos(theta9)*sin(theta7)*sin(theta8) + 2*a4*mtrunk*cos(theta5)*cos(theta7)*cos(theta9)*sin(theta6)*sin(theta8) + 2*a4*mtrunk*cos(theta5)*cos(theta8)*cos(theta9)*sin(theta6)*sin(theta7) - 2*mtrunk*ypelvis*cos(theta6)*cos(theta7)*cos(theta8)*cos(theta9)*sin(theta5) + 2*a1*mshank*cos(theta2)*cos(theta3)*sin(theta4)*sin(theta5)*sin(theta9) - 2*a1*mshank*cos(theta4)*cos(theta5)*sin(theta2)*sin(theta3)*sin(theta9) - 2*mtrunk*xpelvis*cos(theta5)*cos(theta6)*cos(theta9)*sin(theta7)*sin(theta8) - 2*mtrunk*xpelvis*cos(theta5)*cos(theta7)*cos(theta9)*sin(theta6)*sin(theta8) - 2*mtrunk*xpelvis*cos(theta5)*cos(theta8)*cos(theta9)*sin(theta6)*sin(theta7) - lshank*mshank*cos(theta2)*cos(theta3)*sin(theta4)*sin(theta5)*sin(theta9) + lshank*mshank*cos(theta4)*cos(theta5)*sin(theta2)*sin(theta3)*sin(theta9) + 2*mtrunk*ypelvis*cos(theta6)*cos(theta9)*sin(theta5)*sin(theta7)*sin(theta8) + 2*mtrunk*ypelvis*cos(theta7)*cos(theta9)*sin(theta5)*sin(theta6)*sin(theta8) + 2*mtrunk*ypelvis*cos(theta8)*cos(theta9)*sin(theta5)*sin(theta6)*sin(theta7) - 2*a1*mshank*sin(theta2)*sin(theta3)*sin(theta4)*sin(theta5)*sin(theta9) + lshank*mshank*sin(theta2)*sin(theta3)*sin(theta4)*sin(theta5)*sin(theta9) + 2*d3*mshank*cos(theta4)*cos(theta5)*cos(theta6)*cos(theta7)*cos(theta8)*cos(theta9) + 2*d3*mthigh*cos(theta4)*cos(theta5)*cos(theta6)*cos(theta7)*cos(theta8)*cos(theta9) - 2*d3*mshank*cos(theta4)*cos(theta5)*cos(theta6)*cos(theta9)*sin(theta7)*sin(theta8) - 2*d3*mshank*cos(theta4)*cos(theta5)*cos(theta7)*cos(theta9)*sin(theta6)*sin(theta8) - 2*d3*mshank*cos(theta4)*cos(theta5)*cos(theta8)*cos(theta9)*sin(theta6)*sin(theta7) + 2*d3*mshank*cos(theta6)*cos(theta7)*cos(theta8)*cos(theta9)*sin(theta4)*sin(theta5) - 2*d3*mthigh*cos(theta4)*cos(theta5)*cos(theta6)*cos(theta9)*sin(theta7)*sin(theta8) - 2*d3*mthigh*cos(theta4)*cos(theta5)*cos(theta7)*cos(theta9)*sin(theta6)*sin(theta8) - 2*d3*mthigh*cos(theta4)*cos(theta5)*cos(theta8)*cos(theta9)*sin(theta6)*sin(theta7) + 2*d3*mthigh*cos(theta6)*cos(theta7)*cos(theta8)*cos(theta9)*sin(theta4)*sin(theta5) - 2*d3*mshank*cos(theta6)*cos(theta9)*sin(theta4)*sin(theta5)*sin(theta7)*sin(theta8) - 2*d3*mshank*cos(theta7)*cos(theta9)*sin(theta4)*sin(theta5)*sin(theta6)*sin(theta8) - 2*d3*mshank*cos(theta8)*cos(theta9)*sin(theta4)*sin(theta5)*sin(theta6)*sin(theta7) - 2*d3*mthigh*cos(theta6)*cos(theta9)*sin(theta4)*sin(theta5)*sin(theta7)*sin(theta8) - 2*d3*mthigh*cos(theta7)*cos(theta9)*sin(theta4)*sin(theta5)*sin(theta6)*sin(theta8) - 2*d3*mthigh*cos(theta8)*cos(theta9)*sin(theta4)*sin(theta5)*sin(theta6)*sin(theta7) + 2*a2*mshank*cos(theta3)*cos(theta4)*cos(theta6)*cos(theta7)*cos(theta8)*cos(theta9)*sin(theta5) - 2*a2*mshank*cos(theta3)*cos(theta5)*cos(theta6)*cos(theta7)*cos(theta8)*cos(theta9)*sin(theta4) + 2*a2*mthigh*cos(theta3)*cos(theta4)*cos(theta6)*cos(theta7)*cos(theta8)*cos(theta9)*sin(theta5) - 2*a2*mthigh*cos(theta3)*cos(theta5)*cos(theta6)*cos(theta7)*cos(theta8)*cos(theta9)*sin(theta4) - lthigh*mthigh*cos(theta3)*cos(theta4)*cos(theta6)*cos(theta7)*cos(theta8)*cos(theta9)*sin(theta5) + lthigh*mthigh*cos(theta3)*cos(theta5)*cos(theta6)*cos(theta7)*cos(theta8)*cos(theta9)*sin(theta4) - 2*a2*mshank*cos(theta3)*cos(theta4)*cos(theta6)*cos(theta9)*sin(theta5)*sin(theta7)*sin(theta8) - 2*a2*mshank*cos(theta3)*cos(theta4)*cos(theta7)*cos(theta9)*sin(theta5)*sin(theta6)*sin(theta8) - 2*a2*mshank*cos(theta3)*cos(theta4)*cos(theta8)*cos(theta9)*sin(theta5)*sin(theta6)*sin(theta7) + 2*a2*mshank*cos(theta3)*cos(theta5)*cos(theta6)*cos(theta9)*sin(theta4)*sin(theta7)*sin(theta8) + 2*a2*mshank*cos(theta3)*cos(theta5)*cos(theta7)*cos(theta9)*sin(theta4)*sin(theta6)*sin(theta8) + 2*a2*mshank*cos(theta3)*cos(theta5)*cos(theta8)*cos(theta9)*sin(theta4)*sin(theta6)*sin(theta7) - 2*a2*mthigh*cos(theta3)*cos(theta4)*cos(theta6)*cos(theta9)*sin(theta5)*sin(theta7)*sin(theta8) - 2*a2*mthigh*cos(theta3)*cos(theta4)*cos(theta7)*cos(theta9)*sin(theta5)*sin(theta6)*sin(theta8) - 2*a2*mthigh*cos(theta3)*cos(theta4)*cos(theta8)*cos(theta9)*sin(theta5)*sin(theta6)*sin(theta7) + 2*a2*mthigh*cos(theta3)*cos(theta5)*cos(theta6)*cos(theta9)*sin(theta4)*sin(theta7)*sin(theta8) + 2*a2*mthigh*cos(theta3)*cos(theta5)*cos(theta7)*cos(theta9)*sin(theta4)*sin(theta6)*sin(theta8) + 2*a2*mthigh*cos(theta3)*cos(theta5)*cos(theta8)*cos(theta9)*sin(theta4)*sin(theta6)*sin(theta7) + lthigh*mthigh*cos(theta3)*cos(theta4)*cos(theta6)*cos(theta9)*sin(theta5)*sin(theta7)*sin(theta8) + lthigh*mthigh*cos(theta3)*cos(theta4)*cos(theta7)*cos(theta9)*sin(theta5)*sin(theta6)*sin(theta8) + lthigh*mthigh*cos(theta3)*cos(theta4)*cos(theta8)*cos(theta9)*sin(theta5)*sin(theta6)*sin(theta7) - lthigh*mthigh*cos(theta3)*cos(theta5)*cos(theta6)*cos(theta9)*sin(theta4)*sin(theta7)*sin(theta8) - lthigh*mthigh*cos(theta3)*cos(theta5)*cos(theta7)*cos(theta9)*sin(theta4)*sin(theta6)*sin(theta8) - lthigh*mthigh*cos(theta3)*cos(theta5)*cos(theta8)*cos(theta9)*sin(theta4)*sin(theta6)*sin(theta7) - lshank*mshank*cos(theta2)*cos(theta3)*cos(theta4)*cos(theta6)*cos(theta7)*cos(theta8)*cos(theta9)*sin(theta5) + lshank*mshank*cos(theta2)*cos(theta3)*cos(theta5)*cos(theta6)*cos(theta7)*cos(theta8)*cos(theta9)*sin(theta4) - 2*a1*mshank*cos(theta2)*cos(theta3)*cos(theta4)*cos(theta6)*cos(theta9)*sin(theta5)*sin(theta7)*sin(theta8) - 2*a1*mshank*cos(theta2)*cos(theta3)*cos(theta4)*cos(theta7)*cos(theta9)*sin(theta5)*sin(theta6)*sin(theta8) - 2*a1*mshank*cos(theta2)*cos(theta3)*cos(theta4)*cos(theta8)*cos(theta9)*sin(theta5)*sin(theta6)*sin(theta7) + 2*a1*mshank*cos(theta2)*cos(theta3)*cos(theta5)*cos(theta6)*cos(theta9)*sin(theta4)*sin(theta7)*sin(theta8) + 2*a1*mshank*cos(theta2)*cos(theta3)*cos(theta5)*cos(theta7)*cos(theta9)*sin(theta4)*sin(theta6)*sin(theta8) + 2*a1*mshank*cos(theta2)*cos(theta3)*cos(theta5)*cos(theta8)*cos(theta9)*sin(theta4)*sin(theta6)*sin(theta7) - 2*a1*mshank*cos(theta4)*cos(theta6)*cos(theta7)*cos(theta8)*cos(theta9)*sin(theta2)*sin(theta3)*sin(theta5) + 2*a1*mshank*cos(theta5)*cos(theta6)*cos(theta7)*cos(theta8)*cos(theta9)*sin(theta2)*sin(theta3)*sin(theta4) + lshank*mshank*cos(theta2)*cos(theta3)*cos(theta4)*cos(theta6)*cos(theta9)*sin(theta5)*sin(theta7)*sin(theta8) + lshank*mshank*cos(theta2)*cos(theta3)*cos(theta4)*cos(theta7)*cos(theta9)*sin(theta5)*sin(theta6)*sin(theta8) + lshank*mshank*cos(theta2)*cos(theta3)*cos(theta4)*cos(theta8)*cos(theta9)*sin(theta5)*sin(theta6)*sin(theta7) - lshank*mshank*cos(theta2)*cos(theta3)*cos(theta5)*cos(theta6)*cos(theta9)*sin(theta4)*sin(theta7)*sin(theta8) - lshank*mshank*cos(theta2)*cos(theta3)*cos(theta5)*cos(theta7)*cos(theta9)*sin(theta4)*sin(theta6)*sin(theta8) - lshank*mshank*cos(theta2)*cos(theta3)*cos(theta5)*cos(theta8)*cos(theta9)*sin(theta4)*sin(theta6)*sin(theta7) + lshank*mshank*cos(theta4)*cos(theta6)*cos(theta7)*cos(theta8)*cos(theta9)*sin(theta2)*sin(theta3)*sin(theta5) - lshank*mshank*cos(theta5)*cos(theta6)*cos(theta7)*cos(theta8)*cos(theta9)*sin(theta2)*sin(theta3)*sin(theta4) + 2*a1*mshank*cos(theta4)*cos(theta6)*cos(theta9)*sin(theta2)*sin(theta3)*sin(theta5)*sin(theta7)*sin(theta8) + 2*a1*mshank*cos(theta4)*cos(theta7)*cos(theta9)*sin(theta2)*sin(theta3)*sin(theta5)*sin(theta6)*sin(theta8) + 2*a1*mshank*cos(theta4)*cos(theta8)*cos(theta9)*sin(theta2)*sin(theta3)*sin(theta5)*sin(theta6)*sin(theta7) - 2*a1*mshank*cos(theta5)*cos(theta6)*cos(theta9)*sin(theta2)*sin(theta3)*sin(theta4)*sin(theta7)*sin(theta8) - 2*a1*mshank*cos(theta5)*cos(theta7)*cos(theta9)*sin(theta2)*sin(theta3)*sin(theta4)*sin(theta6)*sin(theta8) - 2*a1*mshank*cos(theta5)*cos(theta8)*cos(theta9)*sin(theta2)*sin(theta3)*sin(theta4)*sin(theta6)*sin(theta7) - lshank*mshank*cos(theta4)*cos(theta6)*cos(theta9)*sin(theta2)*sin(theta3)*sin(theta5)*sin(theta7)*sin(theta8) - lshank*mshank*cos(theta4)*cos(theta7)*cos(theta9)*sin(theta2)*sin(theta3)*sin(theta5)*sin(theta6)*sin(theta8) - lshank*mshank*cos(theta4)*cos(theta8)*cos(theta9)*sin(theta2)*sin(theta3)*sin(theta5)*sin(theta6)*sin(theta7) + lshank*mshank*cos(theta5)*cos(theta6)*cos(theta9)*sin(theta2)*sin(theta3)*sin(theta4)*sin(theta7)*sin(theta8) + lshank*mshank*cos(theta5)*cos(theta7)*cos(theta9)*sin(theta2)*sin(theta3)*sin(theta4)*sin(theta6)*sin(theta8) + lshank*mshank*cos(theta5)*cos(theta8)*cos(theta9)*sin(theta2)*sin(theta3)*sin(theta4)*sin(theta6)*sin(theta7) + 2*a1*mshank*cos(theta2)*cos(theta3)*cos(theta4)*cos(theta6)*cos(theta7)*cos(theta8)*cos(theta9)*sin(theta5) - 2*a1*mshank*cos(theta2)*cos(theta3)*cos(theta5)*cos(theta6)*cos(theta7)*cos(theta8)*cos(theta9)*sin(theta4))/(4*mshank + 4*mthigh + 2*mtrunk);
JLcom(1,6)=(2*mtrunk*zpelvis*cos(theta6)*cos(theta7)*cos(theta8)*cos(theta9) - 2*mtrunk*zpelvis*cos(theta6)*cos(theta9)*sin(theta7)*sin(theta8) - 2*mtrunk*zpelvis*cos(theta7)*cos(theta9)*sin(theta6)*sin(theta8) - 2*mtrunk*zpelvis*cos(theta8)*cos(theta9)*sin(theta6)*sin(theta7) - 2*a2*mshank*cos(theta6)*cos(theta7)*cos(theta8)*cos(theta9)*sin(theta3) - 2*a2*mthigh*cos(theta6)*cos(theta7)*cos(theta8)*cos(theta9)*sin(theta3) + lthigh*mthigh*cos(theta6)*cos(theta7)*cos(theta8)*cos(theta9)*sin(theta3) + 2*a4*mshank*cos(theta6)*cos(theta7)*cos(theta9)*sin(theta5)*sin(theta8) + 2*a4*mshank*cos(theta6)*cos(theta8)*cos(theta9)*sin(theta5)*sin(theta7) + 2*a4*mshank*cos(theta7)*cos(theta8)*cos(theta9)*sin(theta5)*sin(theta6) + 2*a4*mthigh*cos(theta6)*cos(theta7)*cos(theta9)*sin(theta5)*sin(theta8) + 2*a4*mthigh*cos(theta6)*cos(theta8)*cos(theta9)*sin(theta5)*sin(theta7) + 2*a4*mthigh*cos(theta7)*cos(theta8)*cos(theta9)*sin(theta5)*sin(theta6) + 2*a4*mtrunk*cos(theta6)*cos(theta7)*cos(theta9)*sin(theta5)*sin(theta8) + 2*a4*mtrunk*cos(theta6)*cos(theta8)*cos(theta9)*sin(theta5)*sin(theta7) + 2*a4*mtrunk*cos(theta7)*cos(theta8)*cos(theta9)*sin(theta5)*sin(theta6) - 2*mtrunk*ypelvis*cos(theta5)*cos(theta6)*cos(theta7)*cos(theta9)*sin(theta8) - 2*mtrunk*ypelvis*cos(theta5)*cos(theta6)*cos(theta8)*cos(theta9)*sin(theta7) - 2*mtrunk*ypelvis*cos(theta5)*cos(theta7)*cos(theta8)*cos(theta9)*sin(theta6) + 2*a2*mshank*cos(theta6)*cos(theta9)*sin(theta3)*sin(theta7)*sin(theta8) + 2*a2*mshank*cos(theta7)*cos(theta9)*sin(theta3)*sin(theta6)*sin(theta8) + 2*a2*mshank*cos(theta8)*cos(theta9)*sin(theta3)*sin(theta6)*sin(theta7) + 2*a2*mthigh*cos(theta6)*cos(theta9)*sin(theta3)*sin(theta7)*sin(theta8) + 2*a2*mthigh*cos(theta7)*cos(theta9)*sin(theta3)*sin(theta6)*sin(theta8) + 2*a2*mthigh*cos(theta8)*cos(theta9)*sin(theta3)*sin(theta6)*sin(theta7) - 2*mtrunk*xpelvis*cos(theta6)*cos(theta7)*cos(theta9)*sin(theta5)*sin(theta8) - 2*mtrunk*xpelvis*cos(theta6)*cos(theta8)*cos(theta9)*sin(theta5)*sin(theta7) - 2*mtrunk*xpelvis*cos(theta7)*cos(theta8)*cos(theta9)*sin(theta5)*sin(theta6) - lthigh*mthigh*cos(theta6)*cos(theta9)*sin(theta3)*sin(theta7)*sin(theta8) - lthigh*mthigh*cos(theta7)*cos(theta9)*sin(theta3)*sin(theta6)*sin(theta8) - lthigh*mthigh*cos(theta8)*cos(theta9)*sin(theta3)*sin(theta6)*sin(theta7) - 2*a4*mshank*cos(theta9)*sin(theta5)*sin(theta6)*sin(theta7)*sin(theta8) - 2*a4*mthigh*cos(theta9)*sin(theta5)*sin(theta6)*sin(theta7)*sin(theta8) - 2*a4*mtrunk*cos(theta9)*sin(theta5)*sin(theta6)*sin(theta7)*sin(theta8) + 2*mtrunk*ypelvis*cos(theta5)*cos(theta9)*sin(theta6)*sin(theta7)*sin(theta8) + 2*mtrunk*xpelvis*cos(theta9)*sin(theta5)*sin(theta6)*sin(theta7)*sin(theta8) - 2*a1*mshank*cos(theta2)*cos(theta6)*cos(theta7)*cos(theta8)*cos(theta9)*sin(theta3) - 2*a1*mshank*cos(theta3)*cos(theta6)*cos(theta7)*cos(theta8)*cos(theta9)*sin(theta2) + lshank*mshank*cos(theta2)*cos(theta6)*cos(theta7)*cos(theta8)*cos(theta9)*sin(theta3) + lshank*mshank*cos(theta3)*cos(theta6)*cos(theta7)*cos(theta8)*cos(theta9)*sin(theta2) - 2*d3*mshank*cos(theta4)*cos(theta6)*cos(theta7)*cos(theta9)*sin(theta5)*sin(theta8) - 2*d3*mshank*cos(theta4)*cos(theta6)*cos(theta8)*cos(theta9)*sin(theta5)*sin(theta7) - 2*d3*mshank*cos(theta4)*cos(theta7)*cos(theta8)*cos(theta9)*sin(theta5)*sin(theta6) + 2*d3*mshank*cos(theta5)*cos(theta6)*cos(theta7)*cos(theta9)*sin(theta4)*sin(theta8) + 2*d3*mshank*cos(theta5)*cos(theta6)*cos(theta8)*cos(theta9)*sin(theta4)*sin(theta7) + 2*d3*mshank*cos(theta5)*cos(theta7)*cos(theta8)*cos(theta9)*sin(theta4)*sin(theta6) - 2*d3*mthigh*cos(theta4)*cos(theta6)*cos(theta7)*cos(theta9)*sin(theta5)*sin(theta8) - 2*d3*mthigh*cos(theta4)*cos(theta6)*cos(theta8)*cos(theta9)*sin(theta5)*sin(theta7) - 2*d3*mthigh*cos(theta4)*cos(theta7)*cos(theta8)*cos(theta9)*sin(theta5)*sin(theta6) + 2*d3*mthigh*cos(theta5)*cos(theta6)*cos(theta7)*cos(theta9)*sin(theta4)*sin(theta8) + 2*d3*mthigh*cos(theta5)*cos(theta6)*cos(theta8)*cos(theta9)*sin(theta4)*sin(theta7) + 2*d3*mthigh*cos(theta5)*cos(theta7)*cos(theta8)*cos(theta9)*sin(theta4)*sin(theta6) + 2*a1*mshank*cos(theta2)*cos(theta6)*cos(theta9)*sin(theta3)*sin(theta7)*sin(theta8) + 2*a1*mshank*cos(theta2)*cos(theta7)*cos(theta9)*sin(theta3)*sin(theta6)*sin(theta8) + 2*a1*mshank*cos(theta2)*cos(theta8)*cos(theta9)*sin(theta3)*sin(theta6)*sin(theta7) + 2*a1*mshank*cos(theta3)*cos(theta6)*cos(theta9)*sin(theta2)*sin(theta7)*sin(theta8) + 2*a1*mshank*cos(theta3)*cos(theta7)*cos(theta9)*sin(theta2)*sin(theta6)*sin(theta8) + 2*a1*mshank*cos(theta3)*cos(theta8)*cos(theta9)*sin(theta2)*sin(theta6)*sin(theta7) - lshank*mshank*cos(theta2)*cos(theta6)*cos(theta9)*sin(theta3)*sin(theta7)*sin(theta8) - lshank*mshank*cos(theta2)*cos(theta7)*cos(theta9)*sin(theta3)*sin(theta6)*sin(theta8) - lshank*mshank*cos(theta2)*cos(theta8)*cos(theta9)*sin(theta3)*sin(theta6)*sin(theta7) - lshank*mshank*cos(theta3)*cos(theta6)*cos(theta9)*sin(theta2)*sin(theta7)*sin(theta8) - lshank*mshank*cos(theta3)*cos(theta7)*cos(theta9)*sin(theta2)*sin(theta6)*sin(theta8) - lshank*mshank*cos(theta3)*cos(theta8)*cos(theta9)*sin(theta2)*sin(theta6)*sin(theta7) + 2*d3*mshank*cos(theta4)*cos(theta9)*sin(theta5)*sin(theta6)*sin(theta7)*sin(theta8) - 2*d3*mshank*cos(theta5)*cos(theta9)*sin(theta4)*sin(theta6)*sin(theta7)*sin(theta8) + 2*d3*mthigh*cos(theta4)*cos(theta9)*sin(theta5)*sin(theta6)*sin(theta7)*sin(theta8) - 2*d3*mthigh*cos(theta5)*cos(theta9)*sin(theta4)*sin(theta6)*sin(theta7)*sin(theta8) + 2*a2*mshank*cos(theta3)*cos(theta4)*cos(theta5)*cos(theta6)*cos(theta7)*cos(theta9)*sin(theta8) + 2*a2*mshank*cos(theta3)*cos(theta4)*cos(theta5)*cos(theta6)*cos(theta8)*cos(theta9)*sin(theta7) + 2*a2*mshank*cos(theta3)*cos(theta4)*cos(theta5)*cos(theta7)*cos(theta8)*cos(theta9)*sin(theta6) + 2*a2*mthigh*cos(theta3)*cos(theta4)*cos(theta5)*cos(theta6)*cos(theta7)*cos(theta9)*sin(theta8) + 2*a2*mthigh*cos(theta3)*cos(theta4)*cos(theta5)*cos(theta6)*cos(theta8)*cos(theta9)*sin(theta7) + 2*a2*mthigh*cos(theta3)*cos(theta4)*cos(theta5)*cos(theta7)*cos(theta8)*cos(theta9)*sin(theta6) - lthigh*mthigh*cos(theta3)*cos(theta4)*cos(theta5)*cos(theta6)*cos(theta7)*cos(theta9)*sin(theta8) - lthigh*mthigh*cos(theta3)*cos(theta4)*cos(theta5)*cos(theta6)*cos(theta8)*cos(theta9)*sin(theta7) - lthigh*mthigh*cos(theta3)*cos(theta4)*cos(theta5)*cos(theta7)*cos(theta8)*cos(theta9)*sin(theta6) - 2*a2*mshank*cos(theta3)*cos(theta4)*cos(theta5)*cos(theta9)*sin(theta6)*sin(theta7)*sin(theta8) + 2*a2*mshank*cos(theta3)*cos(theta6)*cos(theta7)*cos(theta9)*sin(theta4)*sin(theta5)*sin(theta8) + 2*a2*mshank*cos(theta3)*cos(theta6)*cos(theta8)*cos(theta9)*sin(theta4)*sin(theta5)*sin(theta7) + 2*a2*mshank*cos(theta3)*cos(theta7)*cos(theta8)*cos(theta9)*sin(theta4)*sin(theta5)*sin(theta6) - 2*a2*mthigh*cos(theta3)*cos(theta4)*cos(theta5)*cos(theta9)*sin(theta6)*sin(theta7)*sin(theta8) + 2*a2*mthigh*cos(theta3)*cos(theta6)*cos(theta7)*cos(theta9)*sin(theta4)*sin(theta5)*sin(theta8) + 2*a2*mthigh*cos(theta3)*cos(theta6)*cos(theta8)*cos(theta9)*sin(theta4)*sin(theta5)*sin(theta7) + 2*a2*mthigh*cos(theta3)*cos(theta7)*cos(theta8)*cos(theta9)*sin(theta4)*sin(theta5)*sin(theta6) + lthigh*mthigh*cos(theta3)*cos(theta4)*cos(theta5)*cos(theta9)*sin(theta6)*sin(theta7)*sin(theta8) - lthigh*mthigh*cos(theta3)*cos(theta6)*cos(theta7)*cos(theta9)*sin(theta4)*sin(theta5)*sin(theta8) - lthigh*mthigh*cos(theta3)*cos(theta6)*cos(theta8)*cos(theta9)*sin(theta4)*sin(theta5)*sin(theta7) - lthigh*mthigh*cos(theta3)*cos(theta7)*cos(theta8)*cos(theta9)*sin(theta4)*sin(theta5)*sin(theta6) - 2*a2*mshank*cos(theta3)*cos(theta9)*sin(theta4)*sin(theta5)*sin(theta6)*sin(theta7)*sin(theta8) - 2*a2*mthigh*cos(theta3)*cos(theta9)*sin(theta4)*sin(theta5)*sin(theta6)*sin(theta7)*sin(theta8) + lthigh*mthigh*cos(theta3)*cos(theta9)*sin(theta4)*sin(theta5)*sin(theta6)*sin(theta7)*sin(theta8) - lshank*mshank*cos(theta2)*cos(theta3)*cos(theta4)*cos(theta5)*cos(theta6)*cos(theta7)*cos(theta9)*sin(theta8) - lshank*mshank*cos(theta2)*cos(theta3)*cos(theta4)*cos(theta5)*cos(theta6)*cos(theta8)*cos(theta9)*sin(theta7) - lshank*mshank*cos(theta2)*cos(theta3)*cos(theta4)*cos(theta5)*cos(theta7)*cos(theta8)*cos(theta9)*sin(theta6) - 2*a1*mshank*cos(theta2)*cos(theta3)*cos(theta4)*cos(theta5)*cos(theta9)*sin(theta6)*sin(theta7)*sin(theta8) + 2*a1*mshank*cos(theta2)*cos(theta3)*cos(theta6)*cos(theta7)*cos(theta9)*sin(theta4)*sin(theta5)*sin(theta8) + 2*a1*mshank*cos(theta2)*cos(theta3)*cos(theta6)*cos(theta8)*cos(theta9)*sin(theta4)*sin(theta5)*sin(theta7) + 2*a1*mshank*cos(theta2)*cos(theta3)*cos(theta7)*cos(theta8)*cos(theta9)*sin(theta4)*sin(theta5)*sin(theta6) - 2*a1*mshank*cos(theta4)*cos(theta5)*cos(theta6)*cos(theta7)*cos(theta9)*sin(theta2)*sin(theta3)*sin(theta8) - 2*a1*mshank*cos(theta4)*cos(theta5)*cos(theta6)*cos(theta8)*cos(theta9)*sin(theta2)*sin(theta3)*sin(theta7) - 2*a1*mshank*cos(theta4)*cos(theta5)*cos(theta7)*cos(theta8)*cos(theta9)*sin(theta2)*sin(theta3)*sin(theta6) + lshank*mshank*cos(theta2)*cos(theta3)*cos(theta4)*cos(theta5)*cos(theta9)*sin(theta6)*sin(theta7)*sin(theta8) - lshank*mshank*cos(theta2)*cos(theta3)*cos(theta6)*cos(theta7)*cos(theta9)*sin(theta4)*sin(theta5)*sin(theta8) - lshank*mshank*cos(theta2)*cos(theta3)*cos(theta6)*cos(theta8)*cos(theta9)*sin(theta4)*sin(theta5)*sin(theta7) - lshank*mshank*cos(theta2)*cos(theta3)*cos(theta7)*cos(theta8)*cos(theta9)*sin(theta4)*sin(theta5)*sin(theta6) + lshank*mshank*cos(theta4)*cos(theta5)*cos(theta6)*cos(theta7)*cos(theta9)*sin(theta2)*sin(theta3)*sin(theta8) + lshank*mshank*cos(theta4)*cos(theta5)*cos(theta6)*cos(theta8)*cos(theta9)*sin(theta2)*sin(theta3)*sin(theta7) + lshank*mshank*cos(theta4)*cos(theta5)*cos(theta7)*cos(theta8)*cos(theta9)*sin(theta2)*sin(theta3)*sin(theta6) - 2*a1*mshank*cos(theta2)*cos(theta3)*cos(theta9)*sin(theta4)*sin(theta5)*sin(theta6)*sin(theta7)*sin(theta8) + 2*a1*mshank*cos(theta4)*cos(theta5)*cos(theta9)*sin(theta2)*sin(theta3)*sin(theta6)*sin(theta7)*sin(theta8) - 2*a1*mshank*cos(theta6)*cos(theta7)*cos(theta9)*sin(theta2)*sin(theta3)*sin(theta4)*sin(theta5)*sin(theta8) - 2*a1*mshank*cos(theta6)*cos(theta8)*cos(theta9)*sin(theta2)*sin(theta3)*sin(theta4)*sin(theta5)*sin(theta7) - 2*a1*mshank*cos(theta7)*cos(theta8)*cos(theta9)*sin(theta2)*sin(theta3)*sin(theta4)*sin(theta5)*sin(theta6) + lshank*mshank*cos(theta2)*cos(theta3)*cos(theta9)*sin(theta4)*sin(theta5)*sin(theta6)*sin(theta7)*sin(theta8) - lshank*mshank*cos(theta4)*cos(theta5)*cos(theta9)*sin(theta2)*sin(theta3)*sin(theta6)*sin(theta7)*sin(theta8) + lshank*mshank*cos(theta6)*cos(theta7)*cos(theta9)*sin(theta2)*sin(theta3)*sin(theta4)*sin(theta5)*sin(theta8) + lshank*mshank*cos(theta6)*cos(theta8)*cos(theta9)*sin(theta2)*sin(theta3)*sin(theta4)*sin(theta5)*sin(theta7) + lshank*mshank*cos(theta7)*cos(theta8)*cos(theta9)*sin(theta2)*sin(theta3)*sin(theta4)*sin(theta5)*sin(theta6) + 2*a1*mshank*cos(theta9)*sin(theta2)*sin(theta3)*sin(theta4)*sin(theta5)*sin(theta6)*sin(theta7)*sin(theta8) - lshank*mshank*cos(theta9)*sin(theta2)*sin(theta3)*sin(theta4)*sin(theta5)*sin(theta6)*sin(theta7)*sin(theta8) + 2*a1*mshank*cos(theta2)*cos(theta3)*cos(theta4)*cos(theta5)*cos(theta6)*cos(theta7)*cos(theta9)*sin(theta8) + 2*a1*mshank*cos(theta2)*cos(theta3)*cos(theta4)*cos(theta5)*cos(theta6)*cos(theta8)*cos(theta9)*sin(theta7) + 2*a1*mshank*cos(theta2)*cos(theta3)*cos(theta4)*cos(theta5)*cos(theta7)*cos(theta8)*cos(theta9)*sin(theta6))/(4*mshank + 4*mthigh + 2*mtrunk);
JLcom(1,7)=(2*a6*mshank*cos(theta7)*cos(theta9)*sin(theta8) + 2*a6*mshank*cos(theta8)*cos(theta9)*sin(theta7) + 4*a6*mthigh*cos(theta7)*cos(theta9)*sin(theta8) + 4*a6*mthigh*cos(theta8)*cos(theta9)*sin(theta7) + 2*a6*mtrunk*cos(theta7)*cos(theta9)*sin(theta8) + 2*a6*mtrunk*cos(theta8)*cos(theta9)*sin(theta7) + lthigh*mthigh*cos(theta7)*cos(theta9)*sin(theta8) + lthigh*mthigh*cos(theta8)*cos(theta9)*sin(theta7) + 2*mtrunk*zpelvis*cos(theta6)*cos(theta7)*cos(theta8)*cos(theta9) - 2*mtrunk*zpelvis*cos(theta6)*cos(theta9)*sin(theta7)*sin(theta8) - 2*mtrunk*zpelvis*cos(theta7)*cos(theta9)*sin(theta6)*sin(theta8) - 2*mtrunk*zpelvis*cos(theta8)*cos(theta9)*sin(theta6)*sin(theta7) - 2*a2*mshank*cos(theta6)*cos(theta7)*cos(theta8)*cos(theta9)*sin(theta3) - 2*a2*mthigh*cos(theta6)*cos(theta7)*cos(theta8)*cos(theta9)*sin(theta3) + lthigh*mthigh*cos(theta6)*cos(theta7)*cos(theta8)*cos(theta9)*sin(theta3) + 2*a4*mshank*cos(theta6)*cos(theta7)*cos(theta9)*sin(theta5)*sin(theta8) + 2*a4*mshank*cos(theta6)*cos(theta8)*cos(theta9)*sin(theta5)*sin(theta7) + 2*a4*mshank*cos(theta7)*cos(theta8)*cos(theta9)*sin(theta5)*sin(theta6) + 2*a4*mthigh*cos(theta6)*cos(theta7)*cos(theta9)*sin(theta5)*sin(theta8) + 2*a4*mthigh*cos(theta6)*cos(theta8)*cos(theta9)*sin(theta5)*sin(theta7) + 2*a4*mthigh*cos(theta7)*cos(theta8)*cos(theta9)*sin(theta5)*sin(theta6) + 2*a4*mtrunk*cos(theta6)*cos(theta7)*cos(theta9)*sin(theta5)*sin(theta8) + 2*a4*mtrunk*cos(theta6)*cos(theta8)*cos(theta9)*sin(theta5)*sin(theta7) + 2*a4*mtrunk*cos(theta7)*cos(theta8)*cos(theta9)*sin(theta5)*sin(theta6) - 2*mtrunk*ypelvis*cos(theta5)*cos(theta6)*cos(theta7)*cos(theta9)*sin(theta8) - 2*mtrunk*ypelvis*cos(theta5)*cos(theta6)*cos(theta8)*cos(theta9)*sin(theta7) - 2*mtrunk*ypelvis*cos(theta5)*cos(theta7)*cos(theta8)*cos(theta9)*sin(theta6) + 2*a2*mshank*cos(theta6)*cos(theta9)*sin(theta3)*sin(theta7)*sin(theta8) + 2*a2*mshank*cos(theta7)*cos(theta9)*sin(theta3)*sin(theta6)*sin(theta8) + 2*a2*mshank*cos(theta8)*cos(theta9)*sin(theta3)*sin(theta6)*sin(theta7) + 2*a2*mthigh*cos(theta6)*cos(theta9)*sin(theta3)*sin(theta7)*sin(theta8) + 2*a2*mthigh*cos(theta7)*cos(theta9)*sin(theta3)*sin(theta6)*sin(theta8) + 2*a2*mthigh*cos(theta8)*cos(theta9)*sin(theta3)*sin(theta6)*sin(theta7) - 2*mtrunk*xpelvis*cos(theta6)*cos(theta7)*cos(theta9)*sin(theta5)*sin(theta8) - 2*mtrunk*xpelvis*cos(theta6)*cos(theta8)*cos(theta9)*sin(theta5)*sin(theta7) - 2*mtrunk*xpelvis*cos(theta7)*cos(theta8)*cos(theta9)*sin(theta5)*sin(theta6) - lthigh*mthigh*cos(theta6)*cos(theta9)*sin(theta3)*sin(theta7)*sin(theta8) - lthigh*mthigh*cos(theta7)*cos(theta9)*sin(theta3)*sin(theta6)*sin(theta8) - lthigh*mthigh*cos(theta8)*cos(theta9)*sin(theta3)*sin(theta6)*sin(theta7) - 2*a4*mshank*cos(theta9)*sin(theta5)*sin(theta6)*sin(theta7)*sin(theta8) - 2*a4*mthigh*cos(theta9)*sin(theta5)*sin(theta6)*sin(theta7)*sin(theta8) - 2*a4*mtrunk*cos(theta9)*sin(theta5)*sin(theta6)*sin(theta7)*sin(theta8) + 2*mtrunk*ypelvis*cos(theta5)*cos(theta9)*sin(theta6)*sin(theta7)*sin(theta8) + 2*mtrunk*xpelvis*cos(theta9)*sin(theta5)*sin(theta6)*sin(theta7)*sin(theta8) - 2*a1*mshank*cos(theta2)*cos(theta6)*cos(theta7)*cos(theta8)*cos(theta9)*sin(theta3) - 2*a1*mshank*cos(theta3)*cos(theta6)*cos(theta7)*cos(theta8)*cos(theta9)*sin(theta2) + lshank*mshank*cos(theta2)*cos(theta6)*cos(theta7)*cos(theta8)*cos(theta9)*sin(theta3) + lshank*mshank*cos(theta3)*cos(theta6)*cos(theta7)*cos(theta8)*cos(theta9)*sin(theta2) - 2*d3*mshank*cos(theta4)*cos(theta6)*cos(theta7)*cos(theta9)*sin(theta5)*sin(theta8) - 2*d3*mshank*cos(theta4)*cos(theta6)*cos(theta8)*cos(theta9)*sin(theta5)*sin(theta7) - 2*d3*mshank*cos(theta4)*cos(theta7)*cos(theta8)*cos(theta9)*sin(theta5)*sin(theta6) + 2*d3*mshank*cos(theta5)*cos(theta6)*cos(theta7)*cos(theta9)*sin(theta4)*sin(theta8) + 2*d3*mshank*cos(theta5)*cos(theta6)*cos(theta8)*cos(theta9)*sin(theta4)*sin(theta7) + 2*d3*mshank*cos(theta5)*cos(theta7)*cos(theta8)*cos(theta9)*sin(theta4)*sin(theta6) - 2*d3*mthigh*cos(theta4)*cos(theta6)*cos(theta7)*cos(theta9)*sin(theta5)*sin(theta8) - 2*d3*mthigh*cos(theta4)*cos(theta6)*cos(theta8)*cos(theta9)*sin(theta5)*sin(theta7) - 2*d3*mthigh*cos(theta4)*cos(theta7)*cos(theta8)*cos(theta9)*sin(theta5)*sin(theta6) + 2*d3*mthigh*cos(theta5)*cos(theta6)*cos(theta7)*cos(theta9)*sin(theta4)*sin(theta8) + 2*d3*mthigh*cos(theta5)*cos(theta6)*cos(theta8)*cos(theta9)*sin(theta4)*sin(theta7) + 2*d3*mthigh*cos(theta5)*cos(theta7)*cos(theta8)*cos(theta9)*sin(theta4)*sin(theta6) + 2*a1*mshank*cos(theta2)*cos(theta6)*cos(theta9)*sin(theta3)*sin(theta7)*sin(theta8) + 2*a1*mshank*cos(theta2)*cos(theta7)*cos(theta9)*sin(theta3)*sin(theta6)*sin(theta8) + 2*a1*mshank*cos(theta2)*cos(theta8)*cos(theta9)*sin(theta3)*sin(theta6)*sin(theta7) + 2*a1*mshank*cos(theta3)*cos(theta6)*cos(theta9)*sin(theta2)*sin(theta7)*sin(theta8) + 2*a1*mshank*cos(theta3)*cos(theta7)*cos(theta9)*sin(theta2)*sin(theta6)*sin(theta8) + 2*a1*mshank*cos(theta3)*cos(theta8)*cos(theta9)*sin(theta2)*sin(theta6)*sin(theta7) - lshank*mshank*cos(theta2)*cos(theta6)*cos(theta9)*sin(theta3)*sin(theta7)*sin(theta8) - lshank*mshank*cos(theta2)*cos(theta7)*cos(theta9)*sin(theta3)*sin(theta6)*sin(theta8) - lshank*mshank*cos(theta2)*cos(theta8)*cos(theta9)*sin(theta3)*sin(theta6)*sin(theta7) - lshank*mshank*cos(theta3)*cos(theta6)*cos(theta9)*sin(theta2)*sin(theta7)*sin(theta8) - lshank*mshank*cos(theta3)*cos(theta7)*cos(theta9)*sin(theta2)*sin(theta6)*sin(theta8) - lshank*mshank*cos(theta3)*cos(theta8)*cos(theta9)*sin(theta2)*sin(theta6)*sin(theta7) + 2*d3*mshank*cos(theta4)*cos(theta9)*sin(theta5)*sin(theta6)*sin(theta7)*sin(theta8) - 2*d3*mshank*cos(theta5)*cos(theta9)*sin(theta4)*sin(theta6)*sin(theta7)*sin(theta8) + 2*d3*mthigh*cos(theta4)*cos(theta9)*sin(theta5)*sin(theta6)*sin(theta7)*sin(theta8) - 2*d3*mthigh*cos(theta5)*cos(theta9)*sin(theta4)*sin(theta6)*sin(theta7)*sin(theta8) + 2*a2*mshank*cos(theta3)*cos(theta4)*cos(theta5)*cos(theta6)*cos(theta7)*cos(theta9)*sin(theta8) + 2*a2*mshank*cos(theta3)*cos(theta4)*cos(theta5)*cos(theta6)*cos(theta8)*cos(theta9)*sin(theta7) + 2*a2*mshank*cos(theta3)*cos(theta4)*cos(theta5)*cos(theta7)*cos(theta8)*cos(theta9)*sin(theta6) + 2*a2*mthigh*cos(theta3)*cos(theta4)*cos(theta5)*cos(theta6)*cos(theta7)*cos(theta9)*sin(theta8) + 2*a2*mthigh*cos(theta3)*cos(theta4)*cos(theta5)*cos(theta6)*cos(theta8)*cos(theta9)*sin(theta7) + 2*a2*mthigh*cos(theta3)*cos(theta4)*cos(theta5)*cos(theta7)*cos(theta8)*cos(theta9)*sin(theta6) - lthigh*mthigh*cos(theta3)*cos(theta4)*cos(theta5)*cos(theta6)*cos(theta7)*cos(theta9)*sin(theta8) - lthigh*mthigh*cos(theta3)*cos(theta4)*cos(theta5)*cos(theta6)*cos(theta8)*cos(theta9)*sin(theta7) - lthigh*mthigh*cos(theta3)*cos(theta4)*cos(theta5)*cos(theta7)*cos(theta8)*cos(theta9)*sin(theta6) - 2*a2*mshank*cos(theta3)*cos(theta4)*cos(theta5)*cos(theta9)*sin(theta6)*sin(theta7)*sin(theta8) + 2*a2*mshank*cos(theta3)*cos(theta6)*cos(theta7)*cos(theta9)*sin(theta4)*sin(theta5)*sin(theta8) + 2*a2*mshank*cos(theta3)*cos(theta6)*cos(theta8)*cos(theta9)*sin(theta4)*sin(theta5)*sin(theta7) + 2*a2*mshank*cos(theta3)*cos(theta7)*cos(theta8)*cos(theta9)*sin(theta4)*sin(theta5)*sin(theta6) - 2*a2*mthigh*cos(theta3)*cos(theta4)*cos(theta5)*cos(theta9)*sin(theta6)*sin(theta7)*sin(theta8) + 2*a2*mthigh*cos(theta3)*cos(theta6)*cos(theta7)*cos(theta9)*sin(theta4)*sin(theta5)*sin(theta8) + 2*a2*mthigh*cos(theta3)*cos(theta6)*cos(theta8)*cos(theta9)*sin(theta4)*sin(theta5)*sin(theta7) + 2*a2*mthigh*cos(theta3)*cos(theta7)*cos(theta8)*cos(theta9)*sin(theta4)*sin(theta5)*sin(theta6) + lthigh*mthigh*cos(theta3)*cos(theta4)*cos(theta5)*cos(theta9)*sin(theta6)*sin(theta7)*sin(theta8) - lthigh*mthigh*cos(theta3)*cos(theta6)*cos(theta7)*cos(theta9)*sin(theta4)*sin(theta5)*sin(theta8) - lthigh*mthigh*cos(theta3)*cos(theta6)*cos(theta8)*cos(theta9)*sin(theta4)*sin(theta5)*sin(theta7) - lthigh*mthigh*cos(theta3)*cos(theta7)*cos(theta8)*cos(theta9)*sin(theta4)*sin(theta5)*sin(theta6) - 2*a2*mshank*cos(theta3)*cos(theta9)*sin(theta4)*sin(theta5)*sin(theta6)*sin(theta7)*sin(theta8) - 2*a2*mthigh*cos(theta3)*cos(theta9)*sin(theta4)*sin(theta5)*sin(theta6)*sin(theta7)*sin(theta8) + lthigh*mthigh*cos(theta3)*cos(theta9)*sin(theta4)*sin(theta5)*sin(theta6)*sin(theta7)*sin(theta8) - lshank*mshank*cos(theta2)*cos(theta3)*cos(theta4)*cos(theta5)*cos(theta6)*cos(theta7)*cos(theta9)*sin(theta8) - lshank*mshank*cos(theta2)*cos(theta3)*cos(theta4)*cos(theta5)*cos(theta6)*cos(theta8)*cos(theta9)*sin(theta7) - lshank*mshank*cos(theta2)*cos(theta3)*cos(theta4)*cos(theta5)*cos(theta7)*cos(theta8)*cos(theta9)*sin(theta6) - 2*a1*mshank*cos(theta2)*cos(theta3)*cos(theta4)*cos(theta5)*cos(theta9)*sin(theta6)*sin(theta7)*sin(theta8) + 2*a1*mshank*cos(theta2)*cos(theta3)*cos(theta6)*cos(theta7)*cos(theta9)*sin(theta4)*sin(theta5)*sin(theta8) + 2*a1*mshank*cos(theta2)*cos(theta3)*cos(theta6)*cos(theta8)*cos(theta9)*sin(theta4)*sin(theta5)*sin(theta7) + 2*a1*mshank*cos(theta2)*cos(theta3)*cos(theta7)*cos(theta8)*cos(theta9)*sin(theta4)*sin(theta5)*sin(theta6) - 2*a1*mshank*cos(theta4)*cos(theta5)*cos(theta6)*cos(theta7)*cos(theta9)*sin(theta2)*sin(theta3)*sin(theta8) - 2*a1*mshank*cos(theta4)*cos(theta5)*cos(theta6)*cos(theta8)*cos(theta9)*sin(theta2)*sin(theta3)*sin(theta7) - 2*a1*mshank*cos(theta4)*cos(theta5)*cos(theta7)*cos(theta8)*cos(theta9)*sin(theta2)*sin(theta3)*sin(theta6) + lshank*mshank*cos(theta2)*cos(theta3)*cos(theta4)*cos(theta5)*cos(theta9)*sin(theta6)*sin(theta7)*sin(theta8) - lshank*mshank*cos(theta2)*cos(theta3)*cos(theta6)*cos(theta7)*cos(theta9)*sin(theta4)*sin(theta5)*sin(theta8) - lshank*mshank*cos(theta2)*cos(theta3)*cos(theta6)*cos(theta8)*cos(theta9)*sin(theta4)*sin(theta5)*sin(theta7) - lshank*mshank*cos(theta2)*cos(theta3)*cos(theta7)*cos(theta8)*cos(theta9)*sin(theta4)*sin(theta5)*sin(theta6) + lshank*mshank*cos(theta4)*cos(theta5)*cos(theta6)*cos(theta7)*cos(theta9)*sin(theta2)*sin(theta3)*sin(theta8) + lshank*mshank*cos(theta4)*cos(theta5)*cos(theta6)*cos(theta8)*cos(theta9)*sin(theta2)*sin(theta3)*sin(theta7) + lshank*mshank*cos(theta4)*cos(theta5)*cos(theta7)*cos(theta8)*cos(theta9)*sin(theta2)*sin(theta3)*sin(theta6) - 2*a1*mshank*cos(theta2)*cos(theta3)*cos(theta9)*sin(theta4)*sin(theta5)*sin(theta6)*sin(theta7)*sin(theta8) + 2*a1*mshank*cos(theta4)*cos(theta5)*cos(theta9)*sin(theta2)*sin(theta3)*sin(theta6)*sin(theta7)*sin(theta8) - 2*a1*mshank*cos(theta6)*cos(theta7)*cos(theta9)*sin(theta2)*sin(theta3)*sin(theta4)*sin(theta5)*sin(theta8) - 2*a1*mshank*cos(theta6)*cos(theta8)*cos(theta9)*sin(theta2)*sin(theta3)*sin(theta4)*sin(theta5)*sin(theta7) - 2*a1*mshank*cos(theta7)*cos(theta8)*cos(theta9)*sin(theta2)*sin(theta3)*sin(theta4)*sin(theta5)*sin(theta6) + lshank*mshank*cos(theta2)*cos(theta3)*cos(theta9)*sin(theta4)*sin(theta5)*sin(theta6)*sin(theta7)*sin(theta8) - lshank*mshank*cos(theta4)*cos(theta5)*cos(theta9)*sin(theta2)*sin(theta3)*sin(theta6)*sin(theta7)*sin(theta8) + lshank*mshank*cos(theta6)*cos(theta7)*cos(theta9)*sin(theta2)*sin(theta3)*sin(theta4)*sin(theta5)*sin(theta8) + lshank*mshank*cos(theta6)*cos(theta8)*cos(theta9)*sin(theta2)*sin(theta3)*sin(theta4)*sin(theta5)*sin(theta7) + lshank*mshank*cos(theta7)*cos(theta8)*cos(theta9)*sin(theta2)*sin(theta3)*sin(theta4)*sin(theta5)*sin(theta6) + 2*a1*mshank*cos(theta9)*sin(theta2)*sin(theta3)*sin(theta4)*sin(theta5)*sin(theta6)*sin(theta7)*sin(theta8) - lshank*mshank*cos(theta9)*sin(theta2)*sin(theta3)*sin(theta4)*sin(theta5)*sin(theta6)*sin(theta7)*sin(theta8) + 2*a1*mshank*cos(theta2)*cos(theta3)*cos(theta4)*cos(theta5)*cos(theta6)*cos(theta7)*cos(theta9)*sin(theta8) + 2*a1*mshank*cos(theta2)*cos(theta3)*cos(theta4)*cos(theta5)*cos(theta6)*cos(theta8)*cos(theta9)*sin(theta7) + 2*a1*mshank*cos(theta2)*cos(theta3)*cos(theta4)*cos(theta5)*cos(theta7)*cos(theta8)*cos(theta9)*sin(theta6))/(4*mshank + 4*mthigh + 2*mtrunk);
JLcom(1,8)=(4*a7*mshank*cos(theta9)*sin(theta8) + 4*a7*mthigh*cos(theta9)*sin(theta8) + 2*a7*mtrunk*cos(theta9)*sin(theta8) + lshank*mshank*cos(theta9)*sin(theta8) + 2*a6*mshank*cos(theta7)*cos(theta9)*sin(theta8) + 2*a6*mshank*cos(theta8)*cos(theta9)*sin(theta7) + 4*a6*mthigh*cos(theta7)*cos(theta9)*sin(theta8) + 4*a6*mthigh*cos(theta8)*cos(theta9)*sin(theta7) + 2*a6*mtrunk*cos(theta7)*cos(theta9)*sin(theta8) + 2*a6*mtrunk*cos(theta8)*cos(theta9)*sin(theta7) + lthigh*mthigh*cos(theta7)*cos(theta9)*sin(theta8) + lthigh*mthigh*cos(theta8)*cos(theta9)*sin(theta7) + 2*mtrunk*zpelvis*cos(theta6)*cos(theta7)*cos(theta8)*cos(theta9) - 2*mtrunk*zpelvis*cos(theta6)*cos(theta9)*sin(theta7)*sin(theta8) - 2*mtrunk*zpelvis*cos(theta7)*cos(theta9)*sin(theta6)*sin(theta8) - 2*mtrunk*zpelvis*cos(theta8)*cos(theta9)*sin(theta6)*sin(theta7) - 2*a2*mshank*cos(theta6)*cos(theta7)*cos(theta8)*cos(theta9)*sin(theta3) - 2*a2*mthigh*cos(theta6)*cos(theta7)*cos(theta8)*cos(theta9)*sin(theta3) + lthigh*mthigh*cos(theta6)*cos(theta7)*cos(theta8)*cos(theta9)*sin(theta3) + 2*a4*mshank*cos(theta6)*cos(theta7)*cos(theta9)*sin(theta5)*sin(theta8) + 2*a4*mshank*cos(theta6)*cos(theta8)*cos(theta9)*sin(theta5)*sin(theta7) + 2*a4*mshank*cos(theta7)*cos(theta8)*cos(theta9)*sin(theta5)*sin(theta6) + 2*a4*mthigh*cos(theta6)*cos(theta7)*cos(theta9)*sin(theta5)*sin(theta8) + 2*a4*mthigh*cos(theta6)*cos(theta8)*cos(theta9)*sin(theta5)*sin(theta7) + 2*a4*mthigh*cos(theta7)*cos(theta8)*cos(theta9)*sin(theta5)*sin(theta6) + 2*a4*mtrunk*cos(theta6)*cos(theta7)*cos(theta9)*sin(theta5)*sin(theta8) + 2*a4*mtrunk*cos(theta6)*cos(theta8)*cos(theta9)*sin(theta5)*sin(theta7) + 2*a4*mtrunk*cos(theta7)*cos(theta8)*cos(theta9)*sin(theta5)*sin(theta6) - 2*mtrunk*ypelvis*cos(theta5)*cos(theta6)*cos(theta7)*cos(theta9)*sin(theta8) - 2*mtrunk*ypelvis*cos(theta5)*cos(theta6)*cos(theta8)*cos(theta9)*sin(theta7) - 2*mtrunk*ypelvis*cos(theta5)*cos(theta7)*cos(theta8)*cos(theta9)*sin(theta6) + 2*a2*mshank*cos(theta6)*cos(theta9)*sin(theta3)*sin(theta7)*sin(theta8) + 2*a2*mshank*cos(theta7)*cos(theta9)*sin(theta3)*sin(theta6)*sin(theta8) + 2*a2*mshank*cos(theta8)*cos(theta9)*sin(theta3)*sin(theta6)*sin(theta7) + 2*a2*mthigh*cos(theta6)*cos(theta9)*sin(theta3)*sin(theta7)*sin(theta8) + 2*a2*mthigh*cos(theta7)*cos(theta9)*sin(theta3)*sin(theta6)*sin(theta8) + 2*a2*mthigh*cos(theta8)*cos(theta9)*sin(theta3)*sin(theta6)*sin(theta7) - 2*mtrunk*xpelvis*cos(theta6)*cos(theta7)*cos(theta9)*sin(theta5)*sin(theta8) - 2*mtrunk*xpelvis*cos(theta6)*cos(theta8)*cos(theta9)*sin(theta5)*sin(theta7) - 2*mtrunk*xpelvis*cos(theta7)*cos(theta8)*cos(theta9)*sin(theta5)*sin(theta6) - lthigh*mthigh*cos(theta6)*cos(theta9)*sin(theta3)*sin(theta7)*sin(theta8) - lthigh*mthigh*cos(theta7)*cos(theta9)*sin(theta3)*sin(theta6)*sin(theta8) - lthigh*mthigh*cos(theta8)*cos(theta9)*sin(theta3)*sin(theta6)*sin(theta7) - 2*a4*mshank*cos(theta9)*sin(theta5)*sin(theta6)*sin(theta7)*sin(theta8) - 2*a4*mthigh*cos(theta9)*sin(theta5)*sin(theta6)*sin(theta7)*sin(theta8) - 2*a4*mtrunk*cos(theta9)*sin(theta5)*sin(theta6)*sin(theta7)*sin(theta8) + 2*mtrunk*ypelvis*cos(theta5)*cos(theta9)*sin(theta6)*sin(theta7)*sin(theta8) + 2*mtrunk*xpelvis*cos(theta9)*sin(theta5)*sin(theta6)*sin(theta7)*sin(theta8) - 2*a1*mshank*cos(theta2)*cos(theta6)*cos(theta7)*cos(theta8)*cos(theta9)*sin(theta3) - 2*a1*mshank*cos(theta3)*cos(theta6)*cos(theta7)*cos(theta8)*cos(theta9)*sin(theta2) + lshank*mshank*cos(theta2)*cos(theta6)*cos(theta7)*cos(theta8)*cos(theta9)*sin(theta3) + lshank*mshank*cos(theta3)*cos(theta6)*cos(theta7)*cos(theta8)*cos(theta9)*sin(theta2) - 2*d3*mshank*cos(theta4)*cos(theta6)*cos(theta7)*cos(theta9)*sin(theta5)*sin(theta8) - 2*d3*mshank*cos(theta4)*cos(theta6)*cos(theta8)*cos(theta9)*sin(theta5)*sin(theta7) - 2*d3*mshank*cos(theta4)*cos(theta7)*cos(theta8)*cos(theta9)*sin(theta5)*sin(theta6) + 2*d3*mshank*cos(theta5)*cos(theta6)*cos(theta7)*cos(theta9)*sin(theta4)*sin(theta8) + 2*d3*mshank*cos(theta5)*cos(theta6)*cos(theta8)*cos(theta9)*sin(theta4)*sin(theta7) + 2*d3*mshank*cos(theta5)*cos(theta7)*cos(theta8)*cos(theta9)*sin(theta4)*sin(theta6) - 2*d3*mthigh*cos(theta4)*cos(theta6)*cos(theta7)*cos(theta9)*sin(theta5)*sin(theta8) - 2*d3*mthigh*cos(theta4)*cos(theta6)*cos(theta8)*cos(theta9)*sin(theta5)*sin(theta7) - 2*d3*mthigh*cos(theta4)*cos(theta7)*cos(theta8)*cos(theta9)*sin(theta5)*sin(theta6) + 2*d3*mthigh*cos(theta5)*cos(theta6)*cos(theta7)*cos(theta9)*sin(theta4)*sin(theta8) + 2*d3*mthigh*cos(theta5)*cos(theta6)*cos(theta8)*cos(theta9)*sin(theta4)*sin(theta7) + 2*d3*mthigh*cos(theta5)*cos(theta7)*cos(theta8)*cos(theta9)*sin(theta4)*sin(theta6) + 2*a1*mshank*cos(theta2)*cos(theta6)*cos(theta9)*sin(theta3)*sin(theta7)*sin(theta8) + 2*a1*mshank*cos(theta2)*cos(theta7)*cos(theta9)*sin(theta3)*sin(theta6)*sin(theta8) + 2*a1*mshank*cos(theta2)*cos(theta8)*cos(theta9)*sin(theta3)*sin(theta6)*sin(theta7) + 2*a1*mshank*cos(theta3)*cos(theta6)*cos(theta9)*sin(theta2)*sin(theta7)*sin(theta8) + 2*a1*mshank*cos(theta3)*cos(theta7)*cos(theta9)*sin(theta2)*sin(theta6)*sin(theta8) + 2*a1*mshank*cos(theta3)*cos(theta8)*cos(theta9)*sin(theta2)*sin(theta6)*sin(theta7) - lshank*mshank*cos(theta2)*cos(theta6)*cos(theta9)*sin(theta3)*sin(theta7)*sin(theta8) - lshank*mshank*cos(theta2)*cos(theta7)*cos(theta9)*sin(theta3)*sin(theta6)*sin(theta8) - lshank*mshank*cos(theta2)*cos(theta8)*cos(theta9)*sin(theta3)*sin(theta6)*sin(theta7) - lshank*mshank*cos(theta3)*cos(theta6)*cos(theta9)*sin(theta2)*sin(theta7)*sin(theta8) - lshank*mshank*cos(theta3)*cos(theta7)*cos(theta9)*sin(theta2)*sin(theta6)*sin(theta8) - lshank*mshank*cos(theta3)*cos(theta8)*cos(theta9)*sin(theta2)*sin(theta6)*sin(theta7) + 2*d3*mshank*cos(theta4)*cos(theta9)*sin(theta5)*sin(theta6)*sin(theta7)*sin(theta8) - 2*d3*mshank*cos(theta5)*cos(theta9)*sin(theta4)*sin(theta6)*sin(theta7)*sin(theta8) + 2*d3*mthigh*cos(theta4)*cos(theta9)*sin(theta5)*sin(theta6)*sin(theta7)*sin(theta8) - 2*d3*mthigh*cos(theta5)*cos(theta9)*sin(theta4)*sin(theta6)*sin(theta7)*sin(theta8) + 2*a2*mshank*cos(theta3)*cos(theta4)*cos(theta5)*cos(theta6)*cos(theta7)*cos(theta9)*sin(theta8) + 2*a2*mshank*cos(theta3)*cos(theta4)*cos(theta5)*cos(theta6)*cos(theta8)*cos(theta9)*sin(theta7) + 2*a2*mshank*cos(theta3)*cos(theta4)*cos(theta5)*cos(theta7)*cos(theta8)*cos(theta9)*sin(theta6) + 2*a2*mthigh*cos(theta3)*cos(theta4)*cos(theta5)*cos(theta6)*cos(theta7)*cos(theta9)*sin(theta8) + 2*a2*mthigh*cos(theta3)*cos(theta4)*cos(theta5)*cos(theta6)*cos(theta8)*cos(theta9)*sin(theta7) + 2*a2*mthigh*cos(theta3)*cos(theta4)*cos(theta5)*cos(theta7)*cos(theta8)*cos(theta9)*sin(theta6) - lthigh*mthigh*cos(theta3)*cos(theta4)*cos(theta5)*cos(theta6)*cos(theta7)*cos(theta9)*sin(theta8) - lthigh*mthigh*cos(theta3)*cos(theta4)*cos(theta5)*cos(theta6)*cos(theta8)*cos(theta9)*sin(theta7) - lthigh*mthigh*cos(theta3)*cos(theta4)*cos(theta5)*cos(theta7)*cos(theta8)*cos(theta9)*sin(theta6) - 2*a2*mshank*cos(theta3)*cos(theta4)*cos(theta5)*cos(theta9)*sin(theta6)*sin(theta7)*sin(theta8) + 2*a2*mshank*cos(theta3)*cos(theta6)*cos(theta7)*cos(theta9)*sin(theta4)*sin(theta5)*sin(theta8) + 2*a2*mshank*cos(theta3)*cos(theta6)*cos(theta8)*cos(theta9)*sin(theta4)*sin(theta5)*sin(theta7) + 2*a2*mshank*cos(theta3)*cos(theta7)*cos(theta8)*cos(theta9)*sin(theta4)*sin(theta5)*sin(theta6) - 2*a2*mthigh*cos(theta3)*cos(theta4)*cos(theta5)*cos(theta9)*sin(theta6)*sin(theta7)*sin(theta8) + 2*a2*mthigh*cos(theta3)*cos(theta6)*cos(theta7)*cos(theta9)*sin(theta4)*sin(theta5)*sin(theta8) + 2*a2*mthigh*cos(theta3)*cos(theta6)*cos(theta8)*cos(theta9)*sin(theta4)*sin(theta5)*sin(theta7) + 2*a2*mthigh*cos(theta3)*cos(theta7)*cos(theta8)*cos(theta9)*sin(theta4)*sin(theta5)*sin(theta6) + lthigh*mthigh*cos(theta3)*cos(theta4)*cos(theta5)*cos(theta9)*sin(theta6)*sin(theta7)*sin(theta8) - lthigh*mthigh*cos(theta3)*cos(theta6)*cos(theta7)*cos(theta9)*sin(theta4)*sin(theta5)*sin(theta8) - lthigh*mthigh*cos(theta3)*cos(theta6)*cos(theta8)*cos(theta9)*sin(theta4)*sin(theta5)*sin(theta7) - lthigh*mthigh*cos(theta3)*cos(theta7)*cos(theta8)*cos(theta9)*sin(theta4)*sin(theta5)*sin(theta6) - 2*a2*mshank*cos(theta3)*cos(theta9)*sin(theta4)*sin(theta5)*sin(theta6)*sin(theta7)*sin(theta8) - 2*a2*mthigh*cos(theta3)*cos(theta9)*sin(theta4)*sin(theta5)*sin(theta6)*sin(theta7)*sin(theta8) + lthigh*mthigh*cos(theta3)*cos(theta9)*sin(theta4)*sin(theta5)*sin(theta6)*sin(theta7)*sin(theta8) - lshank*mshank*cos(theta2)*cos(theta3)*cos(theta4)*cos(theta5)*cos(theta6)*cos(theta7)*cos(theta9)*sin(theta8) - lshank*mshank*cos(theta2)*cos(theta3)*cos(theta4)*cos(theta5)*cos(theta6)*cos(theta8)*cos(theta9)*sin(theta7) - lshank*mshank*cos(theta2)*cos(theta3)*cos(theta4)*cos(theta5)*cos(theta7)*cos(theta8)*cos(theta9)*sin(theta6) - 2*a1*mshank*cos(theta2)*cos(theta3)*cos(theta4)*cos(theta5)*cos(theta9)*sin(theta6)*sin(theta7)*sin(theta8) + 2*a1*mshank*cos(theta2)*cos(theta3)*cos(theta6)*cos(theta7)*cos(theta9)*sin(theta4)*sin(theta5)*sin(theta8) + 2*a1*mshank*cos(theta2)*cos(theta3)*cos(theta6)*cos(theta8)*cos(theta9)*sin(theta4)*sin(theta5)*sin(theta7) + 2*a1*mshank*cos(theta2)*cos(theta3)*cos(theta7)*cos(theta8)*cos(theta9)*sin(theta4)*sin(theta5)*sin(theta6) - 2*a1*mshank*cos(theta4)*cos(theta5)*cos(theta6)*cos(theta7)*cos(theta9)*sin(theta2)*sin(theta3)*sin(theta8) - 2*a1*mshank*cos(theta4)*cos(theta5)*cos(theta6)*cos(theta8)*cos(theta9)*sin(theta2)*sin(theta3)*sin(theta7) - 2*a1*mshank*cos(theta4)*cos(theta5)*cos(theta7)*cos(theta8)*cos(theta9)*sin(theta2)*sin(theta3)*sin(theta6) + lshank*mshank*cos(theta2)*cos(theta3)*cos(theta4)*cos(theta5)*cos(theta9)*sin(theta6)*sin(theta7)*sin(theta8) - lshank*mshank*cos(theta2)*cos(theta3)*cos(theta6)*cos(theta7)*cos(theta9)*sin(theta4)*sin(theta5)*sin(theta8) - lshank*mshank*cos(theta2)*cos(theta3)*cos(theta6)*cos(theta8)*cos(theta9)*sin(theta4)*sin(theta5)*sin(theta7) - lshank*mshank*cos(theta2)*cos(theta3)*cos(theta7)*cos(theta8)*cos(theta9)*sin(theta4)*sin(theta5)*sin(theta6) + lshank*mshank*cos(theta4)*cos(theta5)*cos(theta6)*cos(theta7)*cos(theta9)*sin(theta2)*sin(theta3)*sin(theta8) + lshank*mshank*cos(theta4)*cos(theta5)*cos(theta6)*cos(theta8)*cos(theta9)*sin(theta2)*sin(theta3)*sin(theta7) + lshank*mshank*cos(theta4)*cos(theta5)*cos(theta7)*cos(theta8)*cos(theta9)*sin(theta2)*sin(theta3)*sin(theta6) - 2*a1*mshank*cos(theta2)*cos(theta3)*cos(theta9)*sin(theta4)*sin(theta5)*sin(theta6)*sin(theta7)*sin(theta8) + 2*a1*mshank*cos(theta4)*cos(theta5)*cos(theta9)*sin(theta2)*sin(theta3)*sin(theta6)*sin(theta7)*sin(theta8) - 2*a1*mshank*cos(theta6)*cos(theta7)*cos(theta9)*sin(theta2)*sin(theta3)*sin(theta4)*sin(theta5)*sin(theta8) - 2*a1*mshank*cos(theta6)*cos(theta8)*cos(theta9)*sin(theta2)*sin(theta3)*sin(theta4)*sin(theta5)*sin(theta7) - 2*a1*mshank*cos(theta7)*cos(theta8)*cos(theta9)*sin(theta2)*sin(theta3)*sin(theta4)*sin(theta5)*sin(theta6) + lshank*mshank*cos(theta2)*cos(theta3)*cos(theta9)*sin(theta4)*sin(theta5)*sin(theta6)*sin(theta7)*sin(theta8) - lshank*mshank*cos(theta4)*cos(theta5)*cos(theta9)*sin(theta2)*sin(theta3)*sin(theta6)*sin(theta7)*sin(theta8) + lshank*mshank*cos(theta6)*cos(theta7)*cos(theta9)*sin(theta2)*sin(theta3)*sin(theta4)*sin(theta5)*sin(theta8) + lshank*mshank*cos(theta6)*cos(theta8)*cos(theta9)*sin(theta2)*sin(theta3)*sin(theta4)*sin(theta5)*sin(theta7) + lshank*mshank*cos(theta7)*cos(theta8)*cos(theta9)*sin(theta2)*sin(theta3)*sin(theta4)*sin(theta5)*sin(theta6) + 2*a1*mshank*cos(theta9)*sin(theta2)*sin(theta3)*sin(theta4)*sin(theta5)*sin(theta6)*sin(theta7)*sin(theta8) - lshank*mshank*cos(theta9)*sin(theta2)*sin(theta3)*sin(theta4)*sin(theta5)*sin(theta6)*sin(theta7)*sin(theta8) + 2*a1*mshank*cos(theta2)*cos(theta3)*cos(theta4)*cos(theta5)*cos(theta6)*cos(theta7)*cos(theta9)*sin(theta8) + 2*a1*mshank*cos(theta2)*cos(theta3)*cos(theta4)*cos(theta5)*cos(theta6)*cos(theta8)*cos(theta9)*sin(theta7) + 2*a1*mshank*cos(theta2)*cos(theta3)*cos(theta4)*cos(theta5)*cos(theta7)*cos(theta8)*cos(theta9)*sin(theta6))/(4*mshank + 4*mthigh + 2*mtrunk);

JLcom(2,5)=-(2*a2*mshank*cos(theta3 + theta4 - theta5 + theta6 + theta7 + theta8) - 2*a2*mshank*cos(theta3 - theta4 + theta5 + theta6 + theta7 + theta8) + 2*a2*mthigh*cos(theta3 + theta4 - theta5 + theta6 + theta7 + theta8) - 2*a2*mthigh*cos(theta3 - theta4 + theta5 + theta6 + theta7 + theta8) - lthigh*mthigh*cos(theta3 + theta4 - theta5 + theta6 + theta7 + theta8) + lthigh*mthigh*cos(theta3 - theta4 + theta5 + theta6 + theta7 + theta8) - 4*a4*mshank*sin(theta6 - theta5 + theta7 + theta8) - 4*a4*mthigh*sin(theta6 - theta5 + theta7 + theta8) - 4*a4*mtrunk*sin(theta6 - theta5 + theta7 + theta8) - 4*mtrunk*ypelvis*cos(theta6 - theta5 + theta7 + theta8) + 2*a1*mshank*cos(theta4 - theta3 - theta2 - theta5 + theta6 + theta7 + theta8) - 2*a1*mshank*cos(theta5 - theta3 - theta4 - theta2 + theta6 + theta7 + theta8) + 4*mtrunk*xpelvis*sin(theta6 - theta5 + theta7 + theta8) - lshank*mshank*cos(theta4 - theta3 - theta2 - theta5 + theta6 + theta7 + theta8) + lshank*mshank*cos(theta5 - theta3 - theta4 - theta2 + theta6 + theta7 + theta8) + 2*a2*mshank*cos(theta4 - theta3 - theta5 + theta6 + theta7 + theta8) - 2*a2*mshank*cos(theta5 - theta4 - theta3 + theta6 + theta7 + theta8) + 2*a2*mthigh*cos(theta4 - theta3 - theta5 + theta6 + theta7 + theta8) - 2*a2*mthigh*cos(theta5 - theta4 - theta3 + theta6 + theta7 + theta8) - lthigh*mthigh*cos(theta4 - theta3 - theta5 + theta6 + theta7 + theta8) + lthigh*mthigh*cos(theta5 - theta4 - theta3 + theta6 + theta7 + theta8) + 2*a1*mshank*cos(theta2 + theta3 + theta4 - theta5 + theta6 + theta7 + theta8) - 2*a1*mshank*cos(theta2 + theta3 - theta4 + theta5 + theta6 + theta7 + theta8) - lshank*mshank*cos(theta2 + theta3 + theta4 - theta5 + theta6 + theta7 + theta8) + lshank*mshank*cos(theta2 + theta3 - theta4 + theta5 + theta6 + theta7 + theta8) + 4*d3*mshank*sin(theta4 - theta5 + theta6 + theta7 + theta8) + 4*d3*mshank*sin(theta5 - theta4 + theta6 + theta7 + theta8) + 4*d3*mthigh*sin(theta4 - theta5 + theta6 + theta7 + theta8) + 4*d3*mthigh*sin(theta5 - theta4 + theta6 + theta7 + theta8) - 4*a4*mshank*sin(theta5 + theta6 + theta7 + theta8) - 4*a4*mthigh*sin(theta5 + theta6 + theta7 + theta8) - 4*a4*mtrunk*sin(theta5 + theta6 + theta7 + theta8) + 4*mtrunk*ypelvis*cos(theta5 + theta6 + theta7 + theta8) + 4*mtrunk*xpelvis*sin(theta5 + theta6 + theta7 + theta8))/(8*(2*mshank + 2*mthigh + mtrunk));
